simulink model "ABB_1010"  (R2024a)
(part 11 of 16)

et336 = Lxcm6.*Lz5.*dQ4.*dQ5.*m6.*t3.*t4.*t5.*t6.*t7.*t10.*-4.0-Lxcm6.*Lz5.*dQ1.*dQ2.*m6.*t2.*t4.*t7.*t9.*t10.*t11.*4.0-Lxcm6.*Lz5.*dQ1.*dQ4.*m6.*t2.*t3.*t7.*t8.*t10.*t11.*4.0+Lxcm6.*Lz4.*dQ1.*dQ6.*m6.*t2.*t3.*t7.*t8.*t10.*t11.*4.0-Lxcm6.*Lz5.*dQ1.*dQ3.*m6.*t2.*t4.*t7.*t9.*t10.*t11.*4.0-Lxcm6.*Lz5.*dQ1.*dQ2.*m6.*t3.*t4.*t8.*t9.*t10.*t11.*4.0-Lxcm6.*Lz5.*dQ1.*dQ3.*m6.*t3.*t4.*t8.*t9.*t10.*t11.*4.0-Lxcm6.*Lz5.*dQ2.*dQ4.*m6.*t2.*t4.*t8.*t9.*t10.*t11.*4.0-Lxcm6.*Lz5.*dQ2.*dQ4.*m6.*t3.*t4.*t7.*t9.*t10.*t11.*4.0-Lxcm6.*Lz5.*dQ3.*dQ4.*m6.*t2.*t4.*t8.*t9.*t10.*t11.*4.0-Lxcm6.*Lz5.*dQ3.*dQ4.*m6.*t3.*t4.*t7.*t9.*t10.*t11.*4.0-Lxcm6.*Lz5.*dQ2.*dQ5.*m6.*t5.*t6.*t7.*t8.*t9.*t10.*4.0-Lxcm6.*Lz5.*dQ3.*dQ5.*m6.*t5.*t6.*t7.*t8.*t9.*t10.*4.0-Lxcm6.*Lz4.*dQ1.*dQ4.*m6.*t2.*t5.*t6.*t7.*t9.*t33.*4.0;
et337 = Lxcm6.*Lz5.*dQ1.*dQ2.*m6.*t2.*t5.*t6.*t7.*t10.*t33.*-8.0+Lxcm6.*Lz5.*dQ1.*dQ5.*m6.*t2.*t3.*t6.*t7.*t8.*t34.*4.0-Lxcm6.*Lz4.*dQ1.*dQ4.*m6.*t3.*t5.*t6.*t8.*t9.*t32.*4.0-Lxcm6.*Lz4.*dQ1.*dQ5.*m6.*t2.*t4.*t6.*t7.*t10.*t33.*4.0+Lxcm6.*Lz5.*dQ1.*dQ2.*m6.*t2.*t5.*t6.*t7.*t10.*t34.*4.0-Lxcm6.*Lz5.*dQ1.*dQ2.*m6.*t3.*t5.*t6.*t8.*t10.*t32.*8.0-Lxcm6.*Lz5.*dQ1.*dQ3.*m6.*t2.*t5.*t6.*t7.*t10.*t33.*8.0-Lxcm6.*Lz5.*dQ1.*dQ4.*m6.*t2.*t4.*t5.*t7.*t11.*t33.*4.0-Lxcm6.*Lz5.*dQ1.*dQ5.*m6.*t2.*t3.*t6.*t7.*t8.*t35.*8.0-Lxcm6.*Lz4.*dQ1.*dQ5.*m6.*t3.*t4.*t6.*t8.*t10.*t32.*4.0-Lxcm6.*Lz4.*dQ1.*dQ6.*m6.*t2.*t4.*t5.*t7.*t11.*t33.*4.0+Lxcm6.*Lz5.*dQ1.*dQ3.*m6.*t2.*t5.*t6.*t7.*t10.*t34.*4.0-Lxcm6.*Lz5.*dQ1.*dQ3.*m6.*t3.*t5.*t6.*t8.*t10.*t32.*8.0-Lxcm6.*Lz5.*dQ1.*dQ4.*m6.*t3.*t4.*t5.*t8.*t11.*t32.*4.0;
et338 = Lxcm6.*Lz4.*dQ1.*dQ6.*m6.*t3.*t4.*t5.*t8.*t11.*t32.*-4.0+Lxcm6.*Lz5.*dQ1.*dQ2.*m6.*t3.*t5.*t6.*t8.*t10.*t34.*4.0-Lxcm6.*Lz5.*dQ1.*dQ6.*m6.*t2.*t5.*t6.*t7.*t9.*t33.*4.0+Lxcm6.*Lz5.*dQ1.*dQ3.*m6.*t3.*t5.*t6.*t8.*t10.*t34.*4.0-Lxcm6.*Lz5.*dQ1.*dQ6.*m6.*t3.*t5.*t6.*t8.*t9.*t32.*4.0+Lxcm6.*Lz5.*dQ1.*dQ4.*m6.*t4.*t5.*t6.*t9.*t10.*t32.*4.0+Lxcm6.*Lz5.*dQ2.*dQ4.*m6.*t2.*t5.*t6.*t8.*t10.*t34.*4.0+Lxcm6.*Lz5.*dQ2.*dQ4.*m6.*t3.*t5.*t6.*t7.*t10.*t34.*4.0+Lxcm6.*Lz5.*dQ1.*dQ4.*m6.*t4.*t5.*t6.*t9.*t10.*t33.*4.0+Lxcm6.*Lz5.*dQ3.*dQ4.*m6.*t2.*t5.*t6.*t8.*t10.*t34.*4.0+Lxcm6.*Lz5.*dQ3.*dQ4.*m6.*t3.*t5.*t6.*t7.*t10.*t34.*4.0+Lxcm6.*Lz5.*dQ1.*dQ5.*m6.*t2.*t7.*t9.*t10.*t11.*t33.*4.0+Lxcm6.*Lz5.*dQ1.*dQ5.*m6.*t3.*t8.*t9.*t10.*t11.*t32.*4.0-Lxcm6.*Lz5.*dQ1.*dQ4.*m6.*t2.*t6.*t7.*t9.*t33.*t35.*8.0;
et339 = Lxcm6.*Lz5.*dQ1.*dQ4.*m6.*t3.*t6.*t8.*t9.*t32.*t35.*-8.0-Lxcm6.*Lz5.*dQ1.*dQ6.*m6.*t2.*t4.*t7.*t11.*t33.*t35.*8.0-Lxcm6.*Lz5.*dQ1.*dQ5.*m6.*t4.*t5.*t9.*t11.*t32.*t33.*4.0-Lxcm6.*Lz5.*dQ1.*dQ6.*m6.*t3.*t4.*t8.*t11.*t32.*t35.*8.0-Lxcm6.*Lz5.*dQ1.*dQ6.*m6.*t4.*t6.*t9.*t10.*t32.*t33.*4.0-Lxcm6.*Lz5.*dQ1.*dQ6.*m6.*t5.*t10.*t11.*t32.*t33.*t34.*4.0+Lxcm6.*Lzcm6.*dQ1.*dQ2.*m6.*t2.*t3.*t4.*t6.*t7.*t8.*8.0+Lxcm6.*Lzcm6.*dQ1.*dQ3.*m6.*t2.*t3.*t4.*t6.*t7.*t8.*8.0+Lxcm5.*Lzcm5.*dQ2.*dQ3.*m5.*t2.*t3.*t4.*t5.*t9.*t10.*4.0+Lxcm6.*Lzcm6.*dQ1.*dQ5.*m6.*t2.*t4.*t5.*t6.*t7.*t10.*8.0+Lxcm6.*Lzcm6.*dQ1.*dQ5.*m6.*t3.*t4.*t5.*t6.*t8.*t10.*8.0+Lxcm6.*Lzcm6.*dQ2.*dQ5.*m6.*t2.*t3.*t5.*t6.*t9.*t10.*4.0+Lxcm6.*Lzcm6.*dQ3.*dQ5.*m6.*t2.*t3.*t5.*t6.*t9.*t10.*4.0-Lxcm6.*Lzcm6.*dQ4.*dQ5.*m6.*t2.*t4.*t5.*t6.*t8.*t10.*4.0;
et340 = Lxcm6.*Lzcm6.*dQ4.*dQ5.*m6.*t3.*t4.*t5.*t6.*t7.*t10.*-4.0-Lxcm5.*Lzcm5.*dQ2.*dQ3.*m5.*t4.*t5.*t7.*t8.*t9.*t10.*4.0-Lxcm6.*Lzcm6.*dQ1.*dQ2.*m6.*t2.*t4.*t7.*t9.*t10.*t11.*4.0-Lxcm6.*Lzcm6.*dQ1.*dQ4.*m6.*t2.*t3.*t7.*t8.*t10.*t11.*4.0-Lxcm6.*Lzcm6.*dQ1.*dQ3.*m6.*t2.*t4.*t7.*t9.*t10.*t11.*4.0-Lxcm6.*Lzcm6.*dQ1.*dQ2.*m6.*t3.*t4.*t8.*t9.*t10.*t11.*4.0-Lxcm6.*Lzcm6.*dQ1.*dQ3.*m6.*t3.*t4.*t8.*t9.*t10.*t11.*4.0-Lxcm6.*Lzcm6.*dQ2.*dQ4.*m6.*t2.*t4.*t8.*t9.*t10.*t11.*4.0-Lxcm6.*Lzcm6.*dQ2.*dQ4.*m6.*t3.*t4.*t7.*t9.*t10.*t11.*4.0-Lxcm6.*Lzcm6.*dQ3.*dQ4.*m6.*t2.*t4.*t8.*t9.*t10.*t11.*4.0-Lxcm6.*Lzcm6.*dQ3.*dQ4.*m6.*t3.*t4.*t7.*t9.*t10.*t11.*4.0-Lxcm6.*Lzcm6.*dQ2.*dQ5.*m6.*t5.*t6.*t7.*t8.*t9.*t10.*4.0-Lxcm6.*Lzcm6.*dQ3.*dQ5.*m6.*t5.*t6.*t7.*t8.*t9.*t10.*4.0-Lxcm5.*Lzcm5.*dQ1.*dQ2.*m5.*t2.*t3.*t4.*t7.*t8.*t35.*1.6e+1;
et341 = Lxcm5.*Lzcm5.*dQ1.*dQ3.*m5.*t2.*t3.*t4.*t7.*t8.*t35.*-1.6e+1-Lxcm5.*Lzcm5.*dQ1.*dQ5.*m5.*t2.*t4.*t5.*t7.*t10.*t33.*1.6e+1-Lxcm5.*Lzcm5.*dQ1.*dQ5.*m5.*t3.*t4.*t5.*t8.*t10.*t32.*1.6e+1-Lxcm6.*Lzcm6.*dQ1.*dQ2.*m6.*t2.*t5.*t6.*t7.*t10.*t33.*8.0+Lxcm6.*Lzcm6.*dQ1.*dQ5.*m6.*t2.*t3.*t6.*t7.*t8.*t34.*4.0+Lxcm6.*Lzcm6.*dQ1.*dQ2.*m6.*t2.*t5.*t6.*t7.*t10.*t34.*4.0-Lxcm6.*Lzcm6.*dQ1.*dQ2.*m6.*t3.*t5.*t6.*t8.*t10.*t32.*8.0-Lxcm6.*Lzcm6.*dQ1.*dQ3.*m6.*t2.*t5.*t6.*t7.*t10.*t33.*8.0-Lxcm6.*Lzcm6.*dQ1.*dQ4.*m6.*t2.*t4.*t5.*t7.*t11.*t33.*4.0-Lxcm6.*Lzcm6.*dQ1.*dQ5.*m6.*t2.*t3.*t6.*t7.*t8.*t35.*8.0+Lxcm6.*Lzcm6.*dQ1.*dQ3.*m6.*t2.*t5.*t6.*t7.*t10.*t34.*4.0-Lxcm6.*Lzcm6.*dQ1.*dQ3.*m6.*t3.*t5.*t6.*t8.*t10.*t32.*8.0-Lxcm6.*Lzcm6.*dQ1.*dQ4.*m6.*t3.*t4.*t5.*t8.*t11.*t32.*4.0+Lxcm6.*Lzcm6.*dQ1.*dQ2.*m6.*t3.*t5.*t6.*t8.*t10.*t34.*4.0;
et342 = Lxcm6.*Lzcm6.*dQ1.*dQ6.*m6.*t2.*t5.*t6.*t7.*t9.*t33.*-4.0+Lxcm6.*Lzcm6.*dQ1.*dQ3.*m6.*t3.*t5.*t6.*t8.*t10.*t34.*4.0-Lxcm6.*Lzcm6.*dQ1.*dQ6.*m6.*t3.*t5.*t6.*t8.*t9.*t32.*4.0+Lxcm6.*Lzcm6.*dQ1.*dQ4.*m6.*t4.*t5.*t6.*t9.*t10.*t32.*4.0+Lxcm6.*Lzcm6.*dQ2.*dQ4.*m6.*t2.*t5.*t6.*t8.*t10.*t34.*4.0+Lxcm6.*Lzcm6.*dQ2.*dQ4.*m6.*t3.*t5.*t6.*t7.*t10.*t34.*4.0+Lxcm6.*Lzcm6.*dQ1.*dQ4.*m6.*t4.*t5.*t6.*t9.*t10.*t33.*4.0+Lxcm6.*Lzcm6.*dQ3.*dQ4.*m6.*t2.*t5.*t6.*t8.*t10.*t34.*4.0+Lxcm6.*Lzcm6.*dQ3.*dQ4.*m6.*t3.*t5.*t6.*t7.*t10.*t34.*4.0+Lxcm6.*Lzcm6.*dQ1.*dQ5.*m6.*t2.*t7.*t9.*t10.*t11.*t33.*4.0+Lxcm6.*Lzcm6.*dQ1.*dQ5.*m6.*t3.*t8.*t9.*t10.*t11.*t32.*4.0-Lxcm5.*Lzcm5.*dQ1.*dQ2.*m5.*t2.*t5.*t7.*t10.*t33.*t34.*8.0-Lxcm5.*Lzcm5.*dQ1.*dQ2.*m5.*t3.*t5.*t8.*t10.*t32.*t34.*8.0-Lxcm5.*Lzcm5.*dQ1.*dQ3.*m5.*t2.*t5.*t7.*t10.*t33.*t34.*8.0;
et343 = Lxcm5.*Lzcm5.*dQ1.*dQ5.*m5.*t2.*t3.*t7.*t8.*t34.*t35.*-8.0-Lxcm5.*Lzcm5.*dQ1.*dQ3.*m5.*t3.*t5.*t8.*t10.*t32.*t34.*8.0-Lxcm5.*Lzcm5.*dQ1.*dQ4.*m5.*t4.*t5.*t9.*t10.*t32.*t33.*8.0-Lxcm6.*Lzcm6.*dQ1.*dQ4.*m6.*t2.*t6.*t7.*t9.*t33.*t35.*8.0-Lxcm6.*Lzcm6.*dQ1.*dQ4.*m6.*t3.*t6.*t8.*t9.*t32.*t35.*8.0-Lxcm6.*Lzcm6.*dQ1.*dQ6.*m6.*t2.*t4.*t7.*t11.*t33.*t35.*8.0-Lxcm6.*Lzcm6.*dQ1.*dQ5.*m6.*t4.*t5.*t9.*t11.*t32.*t33.*4.0-Lxcm6.*Lzcm6.*dQ1.*dQ6.*m6.*t3.*t4.*t8.*t11.*t32.*t35.*8.0-Lxcm6.*Lzcm6.*dQ1.*dQ6.*m6.*t4.*t6.*t9.*t10.*t32.*t33.*4.0-Lxcm6.*Lzcm6.*dQ1.*dQ6.*m6.*t5.*t10.*t11.*t32.*t33.*t34.*4.0+Lycm6.*Lz4.*dQ1.*dQ2.*m6.*t2.*t3.*t6.*t7.*t8.*t9.*8.0+Lycm6.*Lz4.*dQ1.*dQ3.*m6.*t2.*t3.*t6.*t7.*t8.*t9.*8.0-Lycm6.*Lz5.*dQ1.*dQ2.*m6.*t2.*t3.*t4.*t7.*t8.*t11.*8.0;
et344 = Lycm6.*Lz5.*dQ1.*dQ3.*m6.*t2.*t3.*t4.*t7.*t8.*t11.*-8.0+Lycm6.*Lz4.*dQ1.*dQ5.*m6.*t2.*t3.*t5.*t7.*t8.*t11.*4.0-Lycm6.*Lz5.*dQ1.*dQ2.*m6.*t2.*t4.*t6.*t7.*t9.*t10.*4.0-Lycm6.*Lz5.*dQ1.*dQ4.*m6.*t2.*t3.*t6.*t7.*t8.*t10.*4.0+Lycm6.*Lz4.*dQ1.*dQ6.*m6.*t2.*t3.*t6.*t7.*t8.*t10.*4.0-Lycm6.*Lz5.*dQ1.*dQ3.*m6.*t2.*t4.*t6.*t7.*t9.*t10.*4.0-Lycm6.*Lz5.*dQ1.*dQ2.*m6.*t3.*t4.*t6.*t8.*t9.*t10.*4.0-Lycm6.*Lz5.*dQ1.*dQ3.*m6.*t3.*t4.*t6.*t8.*t9.*t10.*4.0-Lycm6.*Lz5.*dQ1.*dQ5.*m6.*t2.*t4.*t5.*t7.*t10.*t11.*8.0-Lycm6.*Lz5.*dQ2.*dQ4.*m6.*t2.*t4.*t6.*t8.*t9.*t10.*4.0-Lycm6.*Lz5.*dQ2.*dQ4.*m6.*t3.*t4.*t6.*t7.*t9.*t10.*4.0-Lycm6.*Lz5.*dQ3.*dQ4.*m6.*t2.*t4.*t6.*t8.*t9.*t10.*4.0-Lycm6.*Lz5.*dQ3.*dQ4.*m6.*t3.*t4.*t6.*t7.*t9.*t10.*4.0-Lycm6.*Lz5.*dQ1.*dQ5.*m6.*t3.*t4.*t5.*t8.*t10.*t11.*8.0;
et345 = Lycm6.*Lz5.*dQ2.*dQ5.*m6.*t2.*t3.*t5.*t9.*t10.*t11.*-4.0-Lycm6.*Lz5.*dQ3.*dQ5.*m6.*t2.*t3.*t5.*t9.*t10.*t11.*4.0+Lycm6.*Lz5.*dQ4.*dQ5.*m6.*t2.*t4.*t5.*t8.*t10.*t11.*4.0+Lycm6.*Lz5.*dQ4.*dQ5.*m6.*t3.*t4.*t5.*t7.*t10.*t11.*4.0+Lycm6.*Lz5.*dQ2.*dQ5.*m6.*t5.*t7.*t8.*t9.*t10.*t11.*4.0+Lycm6.*Lz5.*dQ3.*dQ5.*m6.*t5.*t7.*t8.*t9.*t10.*t11.*4.0-Lycm6.*Lz5.*dQ1.*dQ4.*m6.*t2.*t4.*t5.*t6.*t7.*t33.*4.0-Lycm6.*Lz4.*dQ1.*dQ6.*m6.*t2.*t4.*t5.*t6.*t7.*t33.*4.0-Lycm6.*Lz5.*dQ1.*dQ4.*m6.*t3.*t4.*t5.*t6.*t8.*t32.*4.0-Lycm6.*Lz4.*dQ1.*dQ6.*m6.*t3.*t4.*t5.*t6.*t8.*t32.*4.0+Lycm6.*Lz4.*dQ1.*dQ4.*m6.*t2.*t5.*t7.*t9.*t11.*t33.*4.0+Lycm6.*Lz5.*dQ1.*dQ2.*m6.*t2.*t5.*t7.*t10.*t11.*t33.*8.0-Lycm6.*Lz5.*dQ1.*dQ5.*m6.*t2.*t3.*t7.*t8.*t11.*t34.*4.0+Lycm6.*Lz4.*dQ1.*dQ4.*m6.*t3.*t5.*t8.*t9.*t11.*t32.*4.0;
et346 = Lycm6.*Lz4.*dQ1.*dQ5.*m6.*t2.*t4.*t7.*t10.*t11.*t33.*4.0-Lycm6.*Lz5.*dQ1.*dQ2.*m6.*t2.*t5.*t7.*t10.*t11.*t34.*4.0+Lycm6.*Lz5.*dQ1.*dQ2.*m6.*t3.*t5.*t8.*t10.*t11.*t32.*8.0+Lycm6.*Lz5.*dQ1.*dQ3.*m6.*t2.*t5.*t7.*t10.*t11.*t33.*8.0+Lycm6.*Lz5.*dQ1.*dQ5.*m6.*t2.*t3.*t7.*t8.*t11.*t35.*8.0+Lycm6.*Lz4.*dQ1.*dQ5.*m6.*t3.*t4.*t8.*t10.*t11.*t32.*4.0-Lycm6.*Lz5.*dQ1.*dQ3.*m6.*t2.*t5.*t7.*t10.*t11.*t34.*4.0+Lycm6.*Lz5.*dQ1.*dQ3.*m6.*t3.*t5.*t8.*t10.*t11.*t32.*8.0+Lycm6.*Lz5.*dQ1.*dQ5.*m6.*t2.*t6.*t7.*t9.*t10.*t33.*4.0-Lycm6.*Lz5.*dQ1.*dQ2.*m6.*t3.*t5.*t8.*t10.*t11.*t34.*4.0+Lycm6.*Lz5.*dQ1.*dQ5.*m6.*t3.*t6.*t8.*t9.*t10.*t32.*4.0+Lycm6.*Lz5.*dQ1.*dQ6.*m6.*t2.*t5.*t7.*t9.*t11.*t33.*4.0-Lycm6.*Lz5.*dQ1.*dQ3.*m6.*t3.*t5.*t8.*t10.*t11.*t34.*4.0+Lycm6.*Lz5.*dQ1.*dQ6.*m6.*t3.*t5.*t8.*t9.*t11.*t32.*4.0;
et347 = Lycm6.*Lz5.*dQ1.*dQ4.*m6.*t4.*t5.*t9.*t10.*t11.*t32.*-4.0-Lycm6.*Lz5.*dQ2.*dQ4.*m6.*t2.*t5.*t8.*t10.*t11.*t34.*4.0-Lycm6.*Lz5.*dQ2.*dQ4.*m6.*t3.*t5.*t7.*t10.*t11.*t34.*4.0-Lycm6.*Lz5.*dQ2.*dQ5.*m6.*t2.*t4.*t8.*t9.*t11.*t35.*4.0-Lycm6.*Lz5.*dQ2.*dQ5.*m6.*t3.*t4.*t7.*t9.*t11.*t35.*4.0-Lycm6.*Lz5.*dQ1.*dQ4.*m6.*t4.*t5.*t9.*t10.*t11.*t33.*4.0-Lycm6.*Lz5.*dQ3.*dQ4.*m6.*t2.*t5.*t8.*t10.*t11.*t34.*4.0-Lycm6.*Lz5.*dQ3.*dQ4.*m6.*t3.*t5.*t7.*t10.*t11.*t34.*4.0-Lycm6.*Lz5.*dQ3.*dQ5.*m6.*t2.*t4.*t8.*t9.*t11.*t35.*4.0-Lycm6.*Lz5.*dQ3.*dQ5.*m6.*t3.*t4.*t7.*t9.*t11.*t35.*4.0-Lycm6.*Lz5.*dQ1.*dQ6.*m6.*t2.*t4.*t6.*t7.*t33.*t35.*8.0-Lycm6.*Lz5.*dQ1.*dQ5.*m6.*t4.*t5.*t6.*t9.*t32.*t33.*4.0-Lycm6.*Lz5.*dQ1.*dQ6.*m6.*t3.*t4.*t6.*t8.*t32.*t35.*8.0+Lycm6.*Lz5.*dQ1.*dQ4.*m6.*t2.*t7.*t9.*t11.*t33.*t35.*8.0;
et348 = Lycm6.*Lz5.*dQ1.*dQ4.*m6.*t3.*t8.*t9.*t11.*t32.*t35.*8.0+Lycm6.*Lz5.*dQ1.*dQ6.*m6.*t4.*t9.*t10.*t11.*t32.*t33.*4.0-Lycm6.*Lz5.*dQ1.*dQ6.*m6.*t5.*t6.*t10.*t32.*t33.*t34.*4.0+Lycm5.*Lzcm5.*dQ1.*dQ2.*m5.*t2.*t3.*t5.*t7.*t8.*t9.*8.0+Lycm5.*Lzcm5.*dQ1.*dQ3.*m5.*t2.*t3.*t5.*t7.*t8.*t9.*8.0-Lycm6.*Lzcm6.*dQ1.*dQ2.*m6.*t2.*t3.*t4.*t7.*t8.*t11.*8.0-Lycm6.*Lzcm6.*dQ1.*dQ3.*m6.*t2.*t3.*t4.*t7.*t8.*t11.*8.0-Lycm6.*Lzcm6.*dQ1.*dQ2.*m6.*t2.*t4.*t6.*t7.*t9.*t10.*4.0-Lycm6.*Lzcm6.*dQ1.*dQ4.*m6.*t2.*t3.*t6.*t7.*t8.*t10.*4.0-Lycm6.*Lzcm6.*dQ1.*dQ3.*m6.*t2.*t4.*t6.*t7.*t9.*t10.*4.0-Lycm6.*Lzcm6.*dQ1.*dQ2.*m6.*t3.*t4.*t6.*t8.*t9.*t10.*4.0-Lycm6.*Lzcm6.*dQ1.*dQ3.*m6.*t3.*t4.*t6.*t8.*t9.*t10.*4.0-Lycm6.*Lzcm6.*dQ1.*dQ5.*m6.*t2.*t4.*t5.*t7.*t10.*t11.*8.0-Lycm6.*Lzcm6.*dQ2.*dQ4.*m6.*t2.*t4.*t6.*t8.*t9.*t10.*4.0;
et349 = Lycm6.*Lzcm6.*dQ2.*dQ4.*m6.*t3.*t4.*t6.*t7.*t9.*t10.*-4.0-Lycm6.*Lzcm6.*dQ3.*dQ4.*m6.*t2.*t4.*t6.*t8.*t9.*t10.*4.0-Lycm6.*Lzcm6.*dQ3.*dQ4.*m6.*t3.*t4.*t6.*t7.*t9.*t10.*4.0-Lycm6.*Lzcm6.*dQ1.*dQ5.*m6.*t3.*t4.*t5.*t8.*t10.*t11.*8.0-Lycm6.*Lzcm6.*dQ2.*dQ5.*m6.*t2.*t3.*t5.*t9.*t10.*t11.*4.0-Lycm6.*Lzcm6.*dQ3.*dQ5.*m6.*t2.*t3.*t5.*t9.*t10.*t11.*4.0+Lycm6.*Lzcm6.*dQ4.*dQ5.*m6.*t2.*t4.*t5.*t8.*t10.*t11.*4.0+Lycm6.*Lzcm6.*dQ4.*dQ5.*m6.*t3.*t4.*t5.*t7.*t10.*t11.*4.0+Lycm6.*Lzcm6.*dQ2.*dQ5.*m6.*t5.*t7.*t8.*t9.*t10.*t11.*4.0+Lycm6.*Lzcm6.*dQ3.*dQ5.*m6.*t5.*t7.*t8.*t9.*t10.*t11.*4.0-Lycm6.*Lzcm6.*dQ1.*dQ4.*m6.*t2.*t4.*t5.*t6.*t7.*t33.*4.0-Lycm6.*Lzcm6.*dQ1.*dQ4.*m6.*t3.*t4.*t5.*t6.*t8.*t32.*4.0+Lycm5.*Lzcm5.*dQ1.*dQ2.*m5.*t2.*t4.*t7.*t9.*t10.*t33.*8.0+Lycm5.*Lzcm5.*dQ1.*dQ2.*m5.*t3.*t4.*t8.*t9.*t10.*t32.*8.0;
et350 = Lycm5.*Lzcm5.*dQ1.*dQ3.*m5.*t2.*t4.*t7.*t9.*t10.*t33.*8.0+Lycm5.*Lzcm5.*dQ1.*dQ4.*m5.*t2.*t3.*t7.*t8.*t10.*t34.*8.0+Lycm5.*Lzcm5.*dQ1.*dQ3.*m5.*t3.*t4.*t8.*t9.*t10.*t32.*8.0+Lycm6.*Lzcm6.*dQ1.*dQ2.*m6.*t2.*t5.*t7.*t10.*t11.*t33.*8.0-Lycm6.*Lzcm6.*dQ1.*dQ5.*m6.*t2.*t3.*t7.*t8.*t11.*t34.*4.0-Lycm6.*Lzcm6.*dQ1.*dQ2.*m6.*t2.*t5.*t7.*t10.*t11.*t34.*4.0+Lycm6.*Lzcm6.*dQ1.*dQ2.*m6.*t3.*t5.*t8.*t10.*t11.*t32.*8.0+Lycm6.*Lzcm6.*dQ1.*dQ3.*m6.*t2.*t5.*t7.*t10.*t11.*t33.*8.0+Lycm6.*Lzcm6.*dQ1.*dQ5.*m6.*t2.*t3.*t7.*t8.*t11.*t35.*8.0-Lycm6.*Lzcm6.*dQ1.*dQ3.*m6.*t2.*t5.*t7.*t10.*t11.*t34.*4.0+Lycm6.*Lzcm6.*dQ1.*dQ3.*m6.*t3.*t5.*t8.*t10.*t11.*t32.*8.0+Lycm6.*Lzcm6.*dQ1.*dQ5.*m6.*t2.*t6.*t7.*t9.*t10.*t33.*4.0-Lycm6.*Lzcm6.*dQ1.*dQ2.*m6.*t3.*t5.*t8.*t10.*t11.*t34.*4.0+Lycm6.*Lzcm6.*dQ1.*dQ5.*m6.*t3.*t6.*t8.*t9.*t10.*t32.*4.0;
et351 = Lycm6.*Lzcm6.*dQ1.*dQ6.*m6.*t2.*t5.*t7.*t9.*t11.*t33.*4.0-Lycm6.*Lzcm6.*dQ1.*dQ3.*m6.*t3.*t5.*t8.*t10.*t11.*t34.*4.0+Lycm6.*Lzcm6.*dQ1.*dQ6.*m6.*t3.*t5.*t8.*t9.*t11.*t32.*4.0-Lycm6.*Lzcm6.*dQ1.*dQ4.*m6.*t4.*t5.*t9.*t10.*t11.*t32.*4.0-Lycm6.*Lzcm6.*dQ2.*dQ4.*m6.*t2.*t5.*t8.*t10.*t11.*t34.*4.0-Lycm6.*Lzcm6.*dQ2.*dQ4.*m6.*t3.*t5.*t7.*t10.*t11.*t34.*4.0-Lycm6.*Lzcm6.*dQ2.*dQ5.*m6.*t2.*t4.*t8.*t9.*t11.*t35.*4.0-Lycm6.*Lzcm6.*dQ2.*dQ5.*m6.*t3.*t4.*t7.*t9.*t11.*t35.*4.0-Lycm6.*Lzcm6.*dQ1.*dQ4.*m6.*t4.*t5.*t9.*t10.*t11.*t33.*4.0-Lycm6.*Lzcm6.*dQ3.*dQ4.*m6.*t2.*t5.*t8.*t10.*t11.*t34.*4.0-Lycm6.*Lzcm6.*dQ3.*dQ4.*m6.*t3.*t5.*t7.*t10.*t11.*t34.*4.0-Lycm6.*Lzcm6.*dQ3.*dQ5.*m6.*t2.*t4.*t8.*t9.*t11.*t35.*4.0-Lycm6.*Lzcm6.*dQ3.*dQ5.*m6.*t3.*t4.*t7.*t9.*t11.*t35.*4.0-Lycm6.*Lzcm6.*dQ1.*dQ6.*m6.*t2.*t4.*t6.*t7.*t33.*t35.*8.0;
et352 = Lycm6.*Lzcm6.*dQ1.*dQ5.*m6.*t4.*t5.*t6.*t9.*t32.*t33.*-4.0-Lycm6.*Lzcm6.*dQ1.*dQ6.*m6.*t3.*t4.*t6.*t8.*t32.*t35.*8.0+Lycm6.*Lzcm6.*dQ1.*dQ4.*m6.*t2.*t7.*t9.*t11.*t33.*t35.*8.0+Lycm6.*Lzcm6.*dQ1.*dQ4.*m6.*t3.*t8.*t9.*t11.*t32.*t35.*8.0+Lycm6.*Lzcm6.*dQ1.*dQ6.*m6.*t4.*t9.*t10.*t11.*t32.*t33.*4.0-Lycm6.*Lzcm6.*dQ1.*dQ6.*m6.*t5.*t6.*t10.*t32.*t33.*t34.*4.0-Lz4.*Lz5.*dQ1.*dQ2.*m6.*t2.*t3.*t4.*t7.*t8.*t10.*8.0-Lz4.*Lz5.*dQ1.*dQ3.*m6.*t2.*t3.*t4.*t7.*t8.*t10.*8.0-Lz4.*Lzcm5.*dQ1.*dQ2.*m5.*t2.*t3.*t4.*t7.*t8.*t10.*8.0-Lz4.*Lzcm5.*dQ1.*dQ3.*m5.*t2.*t3.*t4.*t7.*t8.*t10.*8.0-Lz4.*Lzcm6.*dQ1.*dQ2.*m6.*t2.*t3.*t4.*t7.*t8.*t10.*8.0-Lz4.*Lzcm6.*dQ1.*dQ3.*m6.*t2.*t3.*t4.*t7.*t8.*t10.*8.0+Lz5.*Lzcm6.*dQ1.*dQ4.*m6.*t2.*t3.*t4.*t7.*t8.*t9.*8.0;
et353 = Lz5.*Lzcm6.*dQ1.*dQ5.*m6.*t2.*t3.*t5.*t7.*t8.*t10.*-8.0+Lz5.*Lzcm6.*dQ2.*dQ5.*m6.*t2.*t4.*t5.*t8.*t9.*t10.*4.0+Lz5.*Lzcm6.*dQ2.*dQ5.*m6.*t3.*t4.*t5.*t7.*t9.*t10.*4.0+Lz5.*Lzcm6.*dQ3.*dQ5.*m6.*t2.*t4.*t5.*t8.*t9.*t10.*4.0+Lz5.*Lzcm6.*dQ3.*dQ5.*m6.*t3.*t4.*t5.*t7.*t9.*t10.*4.0-Lz5.*Lzcm6.*dQ1.*dQ4.*m6.*t2.*t5.*t7.*t9.*t10.*t33.*8.0-Lz5.*Lzcm6.*dQ1.*dQ4.*m6.*t3.*t5.*t8.*t9.*t10.*t32.*8.0+Lx3.*Lxcm6.*dQ1.*dQ4.*m6.*t2.*t3.*t5.*t6.*t7.*t8.*t9.*4.0+Lx3.*Lxcm6.*dQ1.*dQ5.*m6.*t2.*t3.*t4.*t6.*t7.*t8.*t10.*4.0+Lx3.*Lxcm6.*dQ1.*dQ6.*m6.*t2.*t3.*t4.*t5.*t7.*t8.*t11.*4.0+Lx3.*Lycm6.*dQ1.*dQ6.*m6.*t2.*t3.*t4.*t5.*t6.*t7.*t8.*4.0-Lx3.*Lycm6.*dQ1.*dQ4.*m6.*t2.*t3.*t5.*t7.*t8.*t9.*t11.*4.0-Lx3.*Lycm6.*dQ1.*dQ5.*m6.*t2.*t3.*t4.*t7.*t8.*t10.*t11.*4.0-Lxcm5.*Lycm5.*dQ1.*dQ5.*m5.*t2.*t3.*t4.*t7.*t8.*t9.*t10.*4.0;
et354 = Lxcm6.*Lycm6.*dQ1.*dQ5.*m6.*t2.*t3.*t4.*t7.*t8.*t9.*t10.*4.0+Lxcm6.*Lycm6.*dQ1.*dQ4.*m6.*t2.*t5.*t6.*t7.*t9.*t10.*t11.*4.0+Lxcm6.*Lycm6.*dQ2.*dQ3.*m6.*t2.*t5.*t6.*t8.*t9.*t10.*t11.*4.0+Lxcm6.*Lycm6.*dQ2.*dQ3.*m6.*t3.*t5.*t6.*t7.*t9.*t10.*t11.*4.0+Lxcm6.*Lycm6.*dQ1.*dQ4.*m6.*t3.*t5.*t6.*t8.*t9.*t10.*t11.*4.0-Lxcm6.*Lycm6.*dQ2.*dQ3.*m6.*t2.*t3.*t4.*t6.*t9.*t11.*t35.*4.0-Lxcm6.*Lycm6.*dQ1.*dQ2.*m6.*t2.*t3.*t7.*t8.*t9.*t10.*t36.*1.6e+1-Lxcm6.*Lycm6.*dQ1.*dQ3.*m6.*t2.*t3.*t7.*t8.*t9.*t10.*t36.*1.6e+1-Lxcm6.*Lycm6.*dQ1.*dQ6.*m6.*t2.*t6.*t7.*t9.*t10.*t11.*t33.*1.6e+1+Lxcm6.*Lycm6.*dQ2.*dQ3.*m6.*t4.*t6.*t7.*t8.*t9.*t11.*t35.*4.0-Lxcm6.*Lycm6.*dQ1.*dQ6.*m6.*t3.*t6.*t8.*t9.*t10.*t11.*t32.*1.6e+1+Lxcm6.*Lycm6.*dQ1.*dQ2.*m6.*t2.*t4.*t5.*t7.*t9.*t33.*t36.*1.6e+1+Lxcm6.*Lycm6.*dQ1.*dQ2.*m6.*t3.*t4.*t5.*t8.*t9.*t32.*t36.*1.6e+1;
et355 = Lxcm6.*Lycm6.*dQ1.*dQ3.*m6.*t2.*t4.*t5.*t7.*t9.*t33.*t36.*1.6e+1+Lxcm6.*Lycm6.*dQ1.*dQ4.*m6.*t2.*t3.*t5.*t7.*t8.*t34.*t36.*1.6e+1+Lxcm6.*Lycm6.*dQ1.*dQ3.*m6.*t3.*t4.*t5.*t8.*t9.*t32.*t36.*1.6e+1+Lxcm6.*Lycm6.*dQ1.*dQ2.*m6.*t4.*t5.*t6.*t10.*t11.*t32.*t33.*1.6e+1+Lxcm6.*Lycm6.*dQ1.*dQ5.*m6.*t2.*t4.*t6.*t7.*t11.*t33.*t35.*1.6e+1+Lxcm6.*Lycm6.*dQ1.*dQ6.*m6.*t2.*t4.*t5.*t7.*t10.*t33.*t36.*1.6e+1+Lxcm6.*Lycm6.*dQ1.*dQ3.*m6.*t4.*t5.*t6.*t10.*t11.*t32.*t33.*1.6e+1+Lxcm6.*Lycm6.*dQ1.*dQ5.*m6.*t3.*t4.*t6.*t8.*t11.*t32.*t35.*1.6e+1+Lxcm6.*Lycm6.*dQ1.*dQ6.*m6.*t3.*t4.*t5.*t8.*t10.*t32.*t36.*1.6e+1+Lxcm6.*Lycm6.*dQ1.*dQ6.*m6.*t4.*t5.*t6.*t9.*t11.*t32.*t33.*1.6e+1+Lxcm6.*Lycm6.*dQ1.*dQ2.*m6.*t2.*t6.*t7.*t11.*t33.*t34.*t35.*8.0+Lxcm6.*Lycm6.*dQ1.*dQ2.*m6.*t3.*t6.*t8.*t11.*t32.*t34.*t35.*8.0+Lxcm6.*Lycm6.*dQ1.*dQ3.*m6.*t2.*t6.*t7.*t11.*t33.*t34.*t35.*8.0;
et356 = Lxcm6.*Lycm6.*dQ1.*dQ6.*m6.*t2.*t3.*t7.*t8.*t34.*t35.*t36.*8.0+Lxcm6.*Lycm6.*dQ1.*dQ3.*m6.*t3.*t6.*t8.*t11.*t32.*t34.*t35.*8.0+Lxcm6.*Lycm6.*dQ1.*dQ4.*m6.*t4.*t6.*t9.*t11.*t32.*t33.*t35.*8.0+Lxcm6.*Lycm6.*dQ1.*dQ5.*m6.*t5.*t6.*t10.*t11.*t32.*t33.*t34.*8.0-Lxcm6.*Lz4.*dQ1.*dQ2.*m6.*t2.*t3.*t4.*t5.*t6.*t7.*t8.*8.0-Lxcm6.*Lz4.*dQ1.*dQ3.*m6.*t2.*t3.*t4.*t5.*t6.*t7.*t8.*8.0+Lxcm6.*Lz5.*dQ2.*dQ3.*m6.*t2.*t3.*t4.*t5.*t6.*t9.*t10.*4.0+Lxcm6.*Lz5.*dQ1.*dQ2.*m6.*t2.*t3.*t5.*t7.*t8.*t9.*t11.*8.0+Lxcm6.*Lz5.*dQ1.*dQ3.*m6.*t2.*t3.*t5.*t7.*t8.*t9.*t11.*8.0+Lxcm6.*Lz5.*dQ1.*dQ6.*m6.*t2.*t3.*t5.*t7.*t8.*t10.*t11.*4.0-Lxcm6.*Lz5.*dQ2.*dQ3.*m6.*t4.*t5.*t6.*t7.*t8.*t9.*t10.*4.0-Lxcm6.*Lz5.*dQ2.*dQ6.*m6.*t2.*t4.*t5.*t8.*t9.*t10.*t11.*2.0-Lxcm6.*Lz5.*dQ2.*dQ6.*m6.*t3.*t4.*t5.*t7.*t9.*t10.*t11.*2.0;
et357 = Lxcm6.*Lz5.*dQ3.*dQ6.*m6.*t2.*t4.*t5.*t8.*t9.*t10.*t11.*-2.0-Lxcm6.*Lz5.*dQ3.*dQ6.*m6.*t3.*t4.*t5.*t7.*t9.*t10.*t11.*2.0-Lxcm6.*Lz5.*dQ1.*dQ2.*m6.*t2.*t3.*t4.*t6.*t7.*t8.*t35.*1.6e+1-Lxcm6.*Lz5.*dQ1.*dQ3.*m6.*t2.*t3.*t4.*t6.*t7.*t8.*t35.*1.6e+1-Lxcm6.*Lz5.*dQ1.*dQ5.*m6.*t2.*t4.*t5.*t6.*t7.*t10.*t33.*1.6e+1-Lxcm6.*Lz5.*dQ1.*dQ5.*m6.*t3.*t4.*t5.*t6.*t8.*t10.*t32.*1.6e+1+Lxcm6.*Lz5.*dQ1.*dQ2.*m6.*t2.*t4.*t7.*t9.*t10.*t11.*t33.*8.0+Lxcm6.*Lz5.*dQ1.*dQ2.*m6.*t3.*t4.*t8.*t9.*t10.*t11.*t32.*8.0+Lxcm6.*Lz5.*dQ1.*dQ3.*m6.*t2.*t4.*t7.*t9.*t10.*t11.*t33.*8.0+Lxcm6.*Lz5.*dQ1.*dQ4.*m6.*t2.*t3.*t7.*t8.*t10.*t11.*t34.*8.0+Lxcm6.*Lz5.*dQ1.*dQ3.*m6.*t3.*t4.*t8.*t9.*t10.*t11.*t32.*8.0-Lxcm6.*Lz5.*dQ1.*dQ2.*m6.*t2.*t5.*t6.*t7.*t10.*t33.*t34.*8.0;
et358 = Lxcm6.*Lz5.*dQ1.*dQ2.*m6.*t3.*t5.*t6.*t8.*t10.*t32.*t34.*-8.0-Lxcm6.*Lz5.*dQ1.*dQ3.*m6.*t2.*t5.*t6.*t7.*t10.*t33.*t34.*8.0-Lxcm6.*Lz5.*dQ1.*dQ5.*m6.*t2.*t3.*t6.*t7.*t8.*t34.*t35.*8.0-Lxcm6.*Lz5.*dQ1.*dQ3.*m6.*t3.*t5.*t6.*t8.*t10.*t32.*t34.*8.0-Lxcm6.*Lz5.*dQ1.*dQ4.*m6.*t4.*t5.*t6.*t9.*t10.*t32.*t33.*8.0+Lxcm6.*Lzcm6.*dQ2.*dQ3.*m6.*t2.*t3.*t4.*t5.*t6.*t9.*t10.*4.0+Lxcm6.*Lzcm6.*dQ1.*dQ2.*m6.*t2.*t3.*t5.*t7.*t8.*t9.*t11.*8.0+Lxcm6.*Lzcm6.*dQ1.*dQ3.*m6.*t2.*t3.*t5.*t7.*t8.*t9.*t11.*8.0+Lxcm6.*Lzcm6.*dQ1.*dQ6.*m6.*t2.*t3.*t5.*t7.*t8.*t10.*t11.*4.0-Lxcm6.*Lzcm6.*dQ2.*dQ3.*m6.*t4.*t5.*t6.*t7.*t8.*t9.*t10.*4.0-Lxcm6.*Lzcm6.*dQ2.*dQ6.*m6.*t2.*t4.*t5.*t8.*t9.*t10.*t11.*2.0-Lxcm6.*Lzcm6.*dQ2.*dQ6.*m6.*t3.*t4.*t5.*t7.*t9.*t10.*t11.*2.0-Lxcm6.*Lzcm6.*dQ3.*dQ6.*m6.*t2.*t4.*t5.*t8.*t9.*t10.*t11.*2.0;
et359 = Lxcm6.*Lzcm6.*dQ3.*dQ6.*m6.*t3.*t4.*t5.*t7.*t9.*t10.*t11.*-2.0-Lxcm6.*Lzcm6.*dQ1.*dQ2.*m6.*t2.*t3.*t4.*t6.*t7.*t8.*t35.*1.6e+1-Lxcm6.*Lzcm6.*dQ1.*dQ3.*m6.*t2.*t3.*t4.*t6.*t7.*t8.*t35.*1.6e+1-Lxcm6.*Lzcm6.*dQ1.*dQ5.*m6.*t2.*t4.*t5.*t6.*t7.*t10.*t33.*1.6e+1-Lxcm6.*Lzcm6.*dQ1.*dQ5.*m6.*t3.*t4.*t5.*t6.*t8.*t10.*t32.*1.6e+1+Lxcm6.*Lzcm6.*dQ1.*dQ2.*m6.*t2.*t4.*t7.*t9.*t10.*t11.*t33.*8.0+Lxcm6.*Lzcm6.*dQ1.*dQ2.*m6.*t3.*t4.*t8.*t9.*t10.*t11.*t32.*8.0+Lxcm6.*Lzcm6.*dQ1.*dQ3.*m6.*t2.*t4.*t7.*t9.*t10.*t11.*t33.*8.0+Lxcm6.*Lzcm6.*dQ1.*dQ4.*m6.*t2.*t3.*t7.*t8.*t10.*t11.*t34.*8.0+Lxcm6.*Lzcm6.*dQ1.*dQ3.*m6.*t3.*t4.*t8.*t9.*t10.*t11.*t32.*8.0-Lxcm6.*Lzcm6.*dQ1.*dQ2.*m6.*t2.*t5.*t6.*t7.*t10.*t33.*t34.*8.0-Lxcm6.*Lzcm6.*dQ1.*dQ2.*m6.*t3.*t5.*t6.*t8.*t10.*t32.*t34.*8.0;
et360 = Lxcm6.*Lzcm6.*dQ1.*dQ3.*m6.*t2.*t5.*t6.*t7.*t10.*t33.*t34.*-8.0-Lxcm6.*Lzcm6.*dQ1.*dQ5.*m6.*t2.*t3.*t6.*t7.*t8.*t34.*t35.*8.0-Lxcm6.*Lzcm6.*dQ1.*dQ3.*m6.*t3.*t5.*t6.*t8.*t10.*t32.*t34.*8.0-Lxcm6.*Lzcm6.*dQ1.*dQ4.*m6.*t4.*t5.*t6.*t9.*t10.*t32.*t33.*8.0+Lycm6.*Lz4.*dQ1.*dQ2.*m6.*t2.*t3.*t4.*t5.*t7.*t8.*t11.*8.0+Lycm6.*Lz4.*dQ1.*dQ3.*m6.*t2.*t3.*t4.*t5.*t7.*t8.*t11.*8.0+Lycm6.*Lz5.*dQ1.*dQ2.*m6.*t2.*t3.*t5.*t6.*t7.*t8.*t9.*8.0+Lycm6.*Lz5.*dQ1.*dQ3.*m6.*t2.*t3.*t5.*t6.*t7.*t8.*t9.*8.0+Lycm6.*Lz5.*dQ1.*dQ6.*m6.*t2.*t3.*t5.*t6.*t7.*t8.*t10.*4.0-Lycm6.*Lz5.*dQ2.*dQ3.*m6.*t2.*t3.*t4.*t5.*t9.*t10.*t11.*4.0-Lycm6.*Lz5.*dQ2.*dQ6.*m6.*t2.*t4.*t5.*t6.*t8.*t9.*t10.*2.0-Lycm6.*Lz5.*dQ2.*dQ6.*m6.*t3.*t4.*t5.*t6.*t7.*t9.*t10.*2.0-Lycm6.*Lz5.*dQ3.*dQ6.*m6.*t2.*t4.*t5.*t6.*t8.*t9.*t10.*2.0;
et361 = Lycm6.*Lz5.*dQ3.*dQ6.*m6.*t3.*t4.*t5.*t6.*t7.*t9.*t10.*-2.0+Lycm6.*Lz5.*dQ2.*dQ3.*m6.*t4.*t5.*t7.*t8.*t9.*t10.*t11.*4.0+Lycm6.*Lz5.*dQ1.*dQ2.*m6.*t2.*t3.*t4.*t7.*t8.*t11.*t35.*1.6e+1+Lycm6.*Lz5.*dQ1.*dQ2.*m6.*t2.*t4.*t6.*t7.*t9.*t10.*t33.*8.0+Lycm6.*Lz5.*dQ1.*dQ3.*m6.*t2.*t3.*t4.*t7.*t8.*t11.*t35.*1.6e+1+Lycm6.*Lz5.*dQ1.*dQ2.*m6.*t3.*t4.*t6.*t8.*t9.*t10.*t32.*8.0+Lycm6.*Lz5.*dQ1.*dQ3.*m6.*t2.*t4.*t6.*t7.*t9.*t10.*t33.*8.0+Lycm6.*Lz5.*dQ1.*dQ4.*m6.*t2.*t3.*t6.*t7.*t8.*t10.*t34.*8.0+Lycm6.*Lz5.*dQ1.*dQ3.*m6.*t3.*t4.*t6.*t8.*t9.*t10.*t32.*8.0+Lycm6.*Lz5.*dQ1.*dQ5.*m6.*t2.*t4.*t5.*t7.*t10.*t11.*t33.*1.6e+1+Lycm6.*Lz5.*dQ1.*dQ5.*m6.*t3.*t4.*t5.*t8.*t10.*t11.*t32.*1.6e+1+Lycm6.*Lz5.*dQ1.*dQ2.*m6.*t2.*t5.*t7.*t10.*t11.*t33.*t34.*8.0+Lycm6.*Lz5.*dQ1.*dQ2.*m6.*t3.*t5.*t8.*t10.*t11.*t32.*t34.*8.0;
et362 = Lycm6.*Lz5.*dQ1.*dQ3.*m6.*t2.*t5.*t7.*t10.*t11.*t33.*t34.*8.0+Lycm6.*Lz5.*dQ1.*dQ5.*m6.*t2.*t3.*t7.*t8.*t11.*t34.*t35.*8.0+Lycm6.*Lz5.*dQ1.*dQ3.*m6.*t3.*t5.*t8.*t10.*t11.*t32.*t34.*8.0+Lycm6.*Lz5.*dQ1.*dQ4.*m6.*t4.*t5.*t9.*t10.*t11.*t32.*t33.*8.0+Lycm5.*Lzcm5.*dQ1.*dQ5.*m5.*t2.*t3.*t4.*t5.*t7.*t8.*t9.*4.0+Lycm6.*Lzcm6.*dQ1.*dQ2.*m6.*t2.*t3.*t5.*t6.*t7.*t8.*t9.*8.0+Lycm6.*Lzcm6.*dQ1.*dQ3.*m6.*t2.*t3.*t5.*t6.*t7.*t8.*t9.*8.0+Lycm6.*Lzcm6.*dQ1.*dQ6.*m6.*t2.*t3.*t5.*t6.*t7.*t8.*t10.*4.0-Lycm6.*Lzcm6.*dQ2.*dQ3.*m6.*t2.*t3.*t4.*t5.*t9.*t10.*t11.*4.0-Lycm6.*Lzcm6.*dQ2.*dQ6.*m6.*t2.*t4.*t5.*t6.*t8.*t9.*t10.*2.0-Lycm6.*Lzcm6.*dQ2.*dQ6.*m6.*t3.*t4.*t5.*t6.*t7.*t9.*t10.*2.0-Lycm6.*Lzcm6.*dQ3.*dQ6.*m6.*t2.*t4.*t5.*t6.*t8.*t9.*t10.*2.0-Lycm6.*Lzcm6.*dQ3.*dQ6.*m6.*t3.*t4.*t5.*t6.*t7.*t9.*t10.*2.0;
et363 = Lycm6.*Lzcm6.*dQ2.*dQ3.*m6.*t4.*t5.*t7.*t8.*t9.*t10.*t11.*4.0+Lycm6.*Lzcm6.*dQ1.*dQ2.*m6.*t2.*t3.*t4.*t7.*t8.*t11.*t35.*1.6e+1+Lycm6.*Lzcm6.*dQ1.*dQ2.*m6.*t2.*t4.*t6.*t7.*t9.*t10.*t33.*8.0+Lycm6.*Lzcm6.*dQ1.*dQ3.*m6.*t2.*t3.*t4.*t7.*t8.*t11.*t35.*1.6e+1+Lycm6.*Lzcm6.*dQ1.*dQ2.*m6.*t3.*t4.*t6.*t8.*t9.*t10.*t32.*8.0+Lycm6.*Lzcm6.*dQ1.*dQ3.*m6.*t2.*t4.*t6.*t7.*t9.*t10.*t33.*8.0+Lycm6.*Lzcm6.*dQ1.*dQ4.*m6.*t2.*t3.*t6.*t7.*t8.*t10.*t34.*8.0+Lycm6.*Lzcm6.*dQ1.*dQ3.*m6.*t3.*t4.*t6.*t8.*t9.*t10.*t32.*8.0+Lycm6.*Lzcm6.*dQ1.*dQ5.*m6.*t2.*t4.*t5.*t7.*t10.*t11.*t33.*1.6e+1+Lycm6.*Lzcm6.*dQ1.*dQ5.*m6.*t3.*t4.*t5.*t8.*t10.*t11.*t32.*1.6e+1+Lycm6.*Lzcm6.*dQ1.*dQ2.*m6.*t2.*t5.*t7.*t10.*t11.*t33.*t34.*8.0+Lycm6.*Lzcm6.*dQ1.*dQ2.*m6.*t3.*t5.*t8.*t10.*t11.*t32.*t34.*8.0+Lycm6.*Lzcm6.*dQ1.*dQ3.*m6.*t2.*t5.*t7.*t10.*t11.*t33.*t34.*8.0;
et364 = Lycm6.*Lzcm6.*dQ1.*dQ5.*m6.*t2.*t3.*t7.*t8.*t11.*t34.*t35.*8.0+Lycm6.*Lzcm6.*dQ1.*dQ3.*m6.*t3.*t5.*t8.*t10.*t11.*t32.*t34.*8.0+Lycm6.*Lzcm6.*dQ1.*dQ4.*m6.*t4.*t5.*t9.*t10.*t11.*t32.*t33.*8.0-Lz5.*Lzcm6.*dQ1.*dQ2.*m6.*t2.*t3.*t4.*t5.*t7.*t8.*t10.*1.6e+1-Lz5.*Lzcm6.*dQ1.*dQ3.*m6.*t2.*t3.*t4.*t5.*t7.*t8.*t10.*1.6e+1-Lz5.*Lzcm6.*dQ1.*dQ4.*m6.*t2.*t3.*t4.*t7.*t8.*t9.*t35.*8.0-Lz5.*Lzcm6.*dQ1.*dQ5.*m6.*t2.*t3.*t5.*t7.*t8.*t10.*t34.*8.0-Ixy6.*dQ1.*dQ2.*t2.*t3.*t4.*t5.*t6.*t7.*t8.*t10.*t11.*8.0-Ixy6.*dQ1.*dQ3.*t2.*t3.*t4.*t5.*t6.*t7.*t8.*t10.*t11.*8.0-Ixy6.*dQ1.*dQ4.*t2.*t3.*t4.*t6.*t7.*t8.*t9.*t11.*t35.*4.0-Iyx6.*dQ1.*dQ2.*t2.*t3.*t4.*t5.*t6.*t7.*t8.*t10.*t11.*8.0-Iyx6.*dQ1.*dQ3.*t2.*t3.*t4.*t5.*t6.*t7.*t8.*t10.*t11.*8.0;
et365 = Iyx6.*dQ1.*dQ4.*t2.*t3.*t4.*t6.*t7.*t8.*t9.*t11.*t35.*-4.0-dQ1.*dQ2.*m6.*t2.*t3.*t6.*t7.*t8.*t9.*t10.*t11.*t17.*8.0-dQ1.*dQ3.*m6.*t2.*t3.*t6.*t7.*t8.*t9.*t10.*t11.*t17.*8.0+dQ1.*dQ2.*m6.*t2.*t3.*t6.*t7.*t8.*t9.*t10.*t11.*t20.*8.0+dQ1.*dQ3.*m6.*t2.*t3.*t6.*t7.*t8.*t9.*t10.*t11.*t20.*8.0+dQ1.*dQ2.*m6.*t2.*t3.*t4.*t5.*t7.*t8.*t10.*t17.*t36.*8.0+dQ1.*dQ3.*m6.*t2.*t3.*t4.*t5.*t7.*t8.*t10.*t17.*t36.*8.0+dQ1.*dQ2.*m6.*t2.*t4.*t5.*t6.*t7.*t9.*t11.*t17.*t33.*8.0-dQ1.*dQ2.*m6.*t2.*t3.*t4.*t5.*t7.*t8.*t10.*t20.*t36.*8.0+dQ1.*dQ2.*m6.*t3.*t4.*t5.*t6.*t8.*t9.*t11.*t17.*t32.*8.0+dQ1.*dQ3.*m6.*t2.*t4.*t5.*t6.*t7.*t9.*t11.*t17.*t33.*8.0+dQ1.*dQ4.*m6.*t2.*t3.*t5.*t6.*t7.*t8.*t11.*t17.*t34.*8.0+dQ1.*dQ6.*m6.*t2.*t3.*t4.*t5.*t7.*t8.*t9.*t17.*t36.*8.0;
et366 = dQ1.*dQ3.*m6.*t2.*t3.*t4.*t5.*t7.*t8.*t10.*t20.*t36.*-8.0+dQ1.*dQ3.*m6.*t3.*t4.*t5.*t6.*t8.*t9.*t11.*t17.*t32.*8.0-dQ1.*dQ2.*m6.*t2.*t4.*t5.*t6.*t7.*t9.*t11.*t20.*t33.*8.0-dQ1.*dQ2.*m6.*t3.*t4.*t5.*t6.*t8.*t9.*t11.*t20.*t32.*8.0-dQ1.*dQ3.*m6.*t2.*t4.*t5.*t6.*t7.*t9.*t11.*t20.*t33.*8.0-dQ1.*dQ4.*m6.*t2.*t3.*t5.*t6.*t7.*t8.*t11.*t20.*t34.*8.0-dQ1.*dQ6.*m6.*t2.*t3.*t4.*t5.*t7.*t8.*t9.*t20.*t36.*8.0-dQ1.*dQ3.*m6.*t3.*t4.*t5.*t6.*t8.*t9.*t11.*t20.*t32.*8.0+dQ1.*dQ6.*m6.*t2.*t4.*t5.*t6.*t7.*t10.*t11.*t17.*t33.*8.0+dQ1.*dQ6.*m6.*t3.*t4.*t5.*t6.*t8.*t10.*t11.*t17.*t32.*8.0-dQ1.*dQ6.*m6.*t2.*t4.*t5.*t6.*t7.*t10.*t11.*t20.*t33.*8.0-dQ1.*dQ6.*m6.*t3.*t4.*t5.*t6.*t8.*t10.*t11.*t20.*t32.*8.0;
et367 = dQ1.*dQ4.*m6.*t2.*t3.*t4.*t7.*t8.*t9.*t17.*t35.*t36.*4.0+dQ1.*dQ5.*m6.*t2.*t3.*t5.*t7.*t8.*t10.*t17.*t34.*t36.*4.0-dQ1.*dQ4.*m6.*t2.*t3.*t4.*t7.*t8.*t9.*t20.*t35.*t36.*4.0+dQ1.*dQ6.*m6.*t2.*t3.*t6.*t7.*t8.*t11.*t17.*t34.*t35.*4.0-dQ1.*dQ5.*m6.*t2.*t3.*t5.*t7.*t8.*t10.*t20.*t34.*t36.*4.0-dQ1.*dQ6.*m6.*t2.*t3.*t6.*t7.*t8.*t11.*t20.*t34.*t35.*4.0-dQ1.*dQ5.*m6.*t2.*t3.*t4.*t6.*t7.*t8.*t9.*t10.*t11.*t17.*4.0+dQ1.*dQ5.*m6.*t2.*t3.*t4.*t6.*t7.*t8.*t9.*t10.*t11.*t20.*4.0-Lxcm6.*Lycm6.*dQ1.*dQ4.*m6.*t2.*t3.*t4.*t6.*t7.*t8.*t9.*t11.*8.0-Lxcm6.*Lycm6.*dQ1.*dQ5.*m6.*t2.*t3.*t5.*t6.*t7.*t8.*t10.*t11.*8.0-Lxcm6.*Lycm6.*dQ1.*dQ5.*m6.*t2.*t3.*t4.*t7.*t8.*t9.*t10.*t36.*8.0-Lxcm6.*Lycm6.*dQ1.*dQ4.*m6.*t2.*t5.*t6.*t7.*t9.*t10.*t11.*t33.*8.0;
et368 = Lxcm6.*Lycm6.*dQ1.*dQ4.*m6.*t3.*t5.*t6.*t8.*t9.*t10.*t11.*t32.*-8.0+Lxcm6.*Lz5.*dQ1.*dQ5.*m6.*t2.*t3.*t4.*t5.*t7.*t8.*t9.*t11.*4.0+Lxcm6.*Lz5.*dQ1.*dQ6.*m6.*t2.*t3.*t4.*t6.*t7.*t8.*t9.*t10.*4.0+Lxcm6.*Lz5.*dQ1.*dQ6.*m6.*t2.*t3.*t5.*t7.*t8.*t10.*t11.*t34.*4.0+Lxcm5.*Lzcm5.*dQ1.*dQ4.*m5.*t2.*t3.*t4.*t5.*t7.*t8.*t9.*t10.*8.0+Lxcm6.*Lzcm6.*dQ1.*dQ5.*m6.*t2.*t3.*t4.*t5.*t7.*t8.*t9.*t11.*4.0+Lxcm6.*Lzcm6.*dQ1.*dQ6.*m6.*t2.*t3.*t4.*t6.*t7.*t8.*t9.*t10.*4.0+Lxcm6.*Lzcm6.*dQ1.*dQ6.*m6.*t2.*t3.*t5.*t7.*t8.*t10.*t11.*t34.*4.0+Lycm6.*Lz5.*dQ1.*dQ5.*m6.*t2.*t3.*t4.*t5.*t6.*t7.*t8.*t9.*4.0-Lycm6.*Lz5.*dQ1.*dQ6.*m6.*t2.*t3.*t4.*t7.*t8.*t9.*t10.*t11.*4.0+Lycm6.*Lz5.*dQ1.*dQ6.*m6.*t2.*t3.*t5.*t6.*t7.*t8.*t10.*t34.*4.0+Lycm6.*Lzcm6.*dQ1.*dQ5.*m6.*t2.*t3.*t4.*t5.*t6.*t7.*t8.*t9.*4.0-Lycm6.*Lzcm6.*dQ1.*dQ6.*m6.*t2.*t3.*t4.*t7.*t8.*t9.*t10.*t11.*4.0;
et369 = Lycm6.*Lzcm6.*dQ1.*dQ6.*m6.*t2.*t3.*t5.*t6.*t7.*t8.*t10.*t34.*4.0-Lxcm6.*Lycm6.*dQ1.*dQ2.*m6.*t2.*t3.*t4.*t5.*t6.*t7.*t8.*t10.*t11.*1.6e+1-Lxcm6.*Lycm6.*dQ1.*dQ3.*m6.*t2.*t3.*t4.*t5.*t6.*t7.*t8.*t10.*t11.*1.6e+1-Lxcm6.*Lycm6.*dQ1.*dQ6.*m6.*t2.*t3.*t4.*t5.*t6.*t7.*t8.*t9.*t11.*1.6e+1-Lxcm6.*Lycm6.*dQ1.*dQ4.*m6.*t2.*t3.*t4.*t6.*t7.*t8.*t9.*t11.*t35.*8.0-Lxcm6.*Lycm6.*dQ1.*dQ5.*m6.*t2.*t3.*t5.*t6.*t7.*t8.*t10.*t11.*t34.*8.0+Lxcm6.*Lz5.*dQ1.*dQ4.*m6.*t2.*t3.*t4.*t5.*t6.*t7.*t8.*t9.*t10.*8.0+Lxcm6.*Lzcm6.*dQ1.*dQ4.*m6.*t2.*t3.*t4.*t5.*t6.*t7.*t8.*t9.*t10.*8.0-Lycm6.*Lz5.*dQ1.*dQ4.*m6.*t2.*t3.*t4.*t5.*t7.*t8.*t9.*t10.*t11.*8.0-Lycm6.*Lzcm6.*dQ1.*dQ4.*m6.*t2.*t3.*t4.*t5.*t7.*t8.*t9.*t10.*t11.*8.0;
et370 = et1+et2+et3+et4+et5+et6+et7+et8+et9+et10+et11+et12+et13+et14+et15+et16+et17+et18+et19+et20+et21+et22+et23+et24+et25+et26+et27+et28+et29+et30+et31+et32+et33+et34+et35+et36+et37+et38+et39+et40+et41+et42+et43+et44+et45+et46+et47+et48+et49+et50+et51+et52+et53+et54+et55+et56+et57+et58+et59+et60+et61+et62+et63+et64+et65+et66+et67+et68+et69+et70+et71+et72+et73+et74+et75+et76+et77+et78+et79+et80+et81+et82+et83+et84+et85+et86+et87+et88+et89+et90+et91+et92+et93+et94+et95+et96+et97+et98+et99+et100+et101+et102+et103+et104+et105+et106+et107+et108+et109+et110+et111+et112+et113+et114+et115+et116+et117+et118+et119+et120+et121+et122+et123+et124+et125+et126+et127+et128+et129+et130+et131+et132+et133+et134+et135+et136+et137+et138+et139+et140+et141+et142+et143+et144+et145+et146+et147+et148+et149+et150+et151+et152+et153+et154+et155+et156+et157+et158+et159+et160+et161+et162+et163+et164+et165+et166+et167+et168+et169+et170+et171+et172+et173+et174+et175+et176+et177+et178+et179+et180+et181+et182+et183+et184+et185+et186+et187+et188+et189+et190+et191+et192+et193+et194+et195+et196+et197+et198+et199+et200;
et371 = et201+et202+et203+et204+et205+et206+et207+et208+et209+et210+et211+et212+et213+et214+et215+et216+et217+et218+et219+et220+et221+et222+et223+et224+et225+et226+et227+et228+et229+et230+et231+et232+et233+et234+et235+et236+et237+et238+et239+et240+et241+et242+et243+et244+et245+et246+et247+et248+et249+et250+et251+et252+et253+et254+et255+et256+et257+et258+et259+et260+et261+et262+et263+et264+et265+et266+et267+et268+et269+et270+et271+et272+et273+et274+et275+et276+et277+et278+et279+et280+et281+et282+et283+et284+et285+et286+et287+et288+et289+et290+et291+et292+et293+et294+et295+et296+et297+et298+et299+et300+et301+et302+et303+et304+et305+et306+et307+et308+et309+et310+et311+et312+et313+et314+et315+et316+et317+et318+et319+et320+et321+et322+et323+et324+et325+et326+et327+et328+et329+et330+et331+et332+et333+et334+et335+et336+et337+et338+et339+et340+et341+et342+et343+et344+et345+et346+et347+et348+et349+et350+et351+et352+et353+et354+et355+et356+et357+et358+et359+et360+et361+et362+et363+et364+et365+et366+et367+et368+et369;
et372 = t42+t43+t44+t45+t46+t47+t48+t49+t50+t51+t54+t55+t56+t57+t58+t61+t62+t63+t64+t67+t68+t69+t72+t73+t78+t79+t80+t81+t82+t83+t84+t85+t86+t87+t88+t89+t90+t91+t92+t93+t94+t96+t100+t102+t106+t107+t118+t119+t120+t121+t122+t123+t124+t125+t126+t127+t128+t129+t132+t138+t139+t141+t142+t143+t144+t145+t146+t147+t148+t149+t150+t151+t152+t153+t154+t155+t156+t157+t170+t171+t174+t177+t178+t179+t180+t185+t186+t201+t202+t203+t204+t205+t206+t207+t208+t209+t210+t211+t212+t213+t214+t215+t216+t217+t218+t219+t220+t222+t225+t227+t228+t229+t230+t231+t232+t233+t234+t235+t236+t237+t242+t243+t244+t245+t250+t251+t252+t253+t258+t259+t260+t263+t264+t265+t266+t269+t270+t273+t274+t276+t277+t278+t279+t282+t283+t286+t287+t289+t290+t292+t293+t297+t298+t299+t300+t301+t302+t303+t304+t305+t306+t307+t308+t309+t310+t311+t312+t313+t314+t315+t316+t317+t318+t319+t320+t321+t322+t323+t324+t325+t326+t327+t328+t331+t332+t333+t334+t340+t341+t342+t343+t349+t351+t358+t363+t364+t367+t368+t369+t370;
et373 = t377+t378+t379+t380+t381+t382+t383+t384+t385+t386+t402+t403+t404+t405+t406+t407+t415+t416+t417+t418+t419+t430+t431+t432+t433+t434+t435+t436+t437+t438+t442+t443+t444+t445+t446+t447+t454+t455+t456+t457+t458+t459+t460+t461+t462+t463+t464+t465+t466+t467+t468+t469+t470+t471+t472+t473+t474+t475+t476+t477+t478+t479+t480+t481+t482+t483+t484+t485+t486+t487+t488+t489+t490+t491+t492+t493+t494+t495+t496+t497+t498+t500+t506+t512+t514+t515+t516+t527+t528+t529+t540+t542+t543+t544+t546+t547+t548+t550+t552+t554+t555+t556+t557+t558+t559+t560+t561+t562+t563+t564+t565+t566+t567+t568+t569+t570+t571+t572+t573+t574+t575+t576+t577+t578+t579+t580+t581+t582+t583+t584+t585+t586+t587+t588+t589+t590+t591+t592+t593+t594+t595+t596+t597+t598+t599+t600+t601+t602+t603+t604+t605+t606+t607+t608+t609+t610+t611+t612+t613+t614+t615+t616+t617+t618+t619+t620+t621+t622+t623+t624+t625+t626+t627+t628+t629+t630+t631+t632+t635+t636+t637+t638+t648+t650+t651+t658+t659+t660+t661+t662+t663+t664+t669+t670+t671+t674+t675+t676+t677+t681;
et374 = t684+t687+t688+t689+t690+t694+t697+t698+t699+t700+t701+t702+t703+t704+t705+t706+t707+t708+t709+t710+t711+t716+t717+t718+t719+t720+t721+t724+t725+t728+t729+t730+t731+t732+t733+t734+t735+t737+t738+t739+t746+t748+t749+t750+t752+t754+t755+t756+t759+t760+t761+t762+t774+t775+t776+t777+t778+t779+t780+t781+t782+t783+t785+t788+t791+t792+t793+t794+t795+t798+t800+t801+t803+t804+t806+t807+t809+t810+t828+t829+t830+t831+t832+t833+t834+t835+t836+t837+t838+t839+t840+t843+t844+t845+t848+t849+t851+t852+t857+t858+t861+t862+t868+t869+t870+t871+t872+t873+t874+t875+t876+t877+t878+t879+t880+t881+t882+t883+t884+t885+t886+t887+t888+t889+t890+t891+t892+t893+t894+t895+t896+t897+t898+t899+t900+t901+t902+t903+t904+t905+t906+t907+t908+t909+t910+t911+t912+t913+t914+t915+t916+t917+t918+t919+t920+t921+t922+t923+t924+t925+t926+t927+t928+t929+t930+t931+t932+t933+t934+t935+t936+t938+t939+t940+t941+t942+t943+t950+t951+t952+t953+t954+t955+t956+t957+t958+t959+t960+t961+t962+t963+t964+t965+t966+t967+t968+t969+t972+t973+t978;
et375 = t979+t984+t985+t988+t989+t990+t991+t992+t993+t994+t995+t996+t997+t998+t1001+t1002+t1003+t1004+t1005+t1006+t1007+t1008+t1009+t1010+t1011+t1012+t1013+t1014+t1015+t1016+t1017+t1018+t1019+t1020+t1021+t1022+t1023+t1024+t1025+t1026+t1027+t1028+t1029+t1030+t1033+t1034+t1035+t1036+t1037+t1038+t1039+t1041+t1046+t1060+t1061+t1062+t1063+t1064+t1065+t1066+t1067+t1072+t1073+t1074+t1075+t1076+t1077+t1078+t1079+t1082+t1083+t1084+t1085+t1093+t1094+t1095+t1096+t1097+t1098+t1099+t1103+t1104+t1105+t1106+t1107+t1108+t1109+t1110+t1111+t1112+t1113+t1114+t1115+t1116+t1117+t1118+t1120+t1127+t1139+t1140+t1145+t1146+t1147+t1148+t1149+t1150+t1154+t1155+t1158+t1159+t1167+t1169+t1170+t1173+t1174+t1175+t1177+t1178+t1179+t1180+t1181+t1182+t1187+t1193+t1194+t1197+t1198+t1199+t1200+t1202+t1204+t1205+t1206+t1208+t1213+t1214+t1215+t1216+t1217+t1218+t1219+t1223+t1224+t1225+t1226+t1227+t1228+t1229+t1230+t1231+t1242+t1243+t1246+t1249+t1250+t1251+t1252+t1253+t1254+t1255+t1256+t1257+t1258+t1259+t1262+t1263+t1264+t1265+t1266+t1269+t1272+t1275+t1276+t1278+t1279+t1283+t1285+t1286+t1287+t1288+t1289+t1290+t1291+t1292+t1293+t1294+t1295+t1296+t1297+t1298+t1299+t1300+t1301+t1302+t1303+t1304+t1305+t1306+t1307+t1308;
et376 = t1309+t1310+t1311+t1312+t1313+t1314+t1315+t1316+t1317+t1318+t1319+t1320+t1321+t1322+t1323+t1324+t1325+t1326+t1327+t1328+t1329+t1330+t1331+t1332+t1333+t1334+t1335+t1336+t1337+t1338+t1339+t1340+t1341+t1342+t1343+t1344+t1345+t1346+t1347+t1348+t1349+t1350+t1351+t1352+t1353+t1354+t1355+t1356+t1357+t1358+t1359+t1360+t1361+t1362+t1363+t1364+t1365+t1366+t1367+t1368+t1369+t1370+t1371+t1372+t1373+t1374+t1375+t1376+t1377+t1378+t1379+t1381+t1382+t1383+t1384+t1385+t1386+t1387+t1388+t1389+t1390+t1391+t1392+t1393+t1394+t1395+t1396+t1397+t1398+t1399+t1400+t1401+t1402+t1403+t1404+t1405+t1406+t1407+t1408+t1409+t1410+t1411+t1420+t1421+t1422+t1423+t1424+t1425+t1426+t1427+t1428+t1429+t1430+t1431+t1432+t1433+t1434+t1435+t1436+t1437+t1438+t1439+t1440+t1441+t1442+t1443+t1444+t1445+t1446+t1447+t1448+t1449+t1450+t1451+t1452+t1453+t1454+t1455+t1456+t1457+t1458+t1469+t1471+t1472+t1474+t1475+t1481+t1482+t1484+t1487+t1490+t1493+t1496+t1497+t1498+t1499+t1500+t1501+t1502+t1503+t1504+t1505+t1506+t1507+t1508+t1509+t1510+t1511+t1512+t1513+t1514+t1515+t1516+t1517+t1518+t1519+t1520+t1521+t1522+t1523+t1524+t1525+t1526+t1531+t1532+t1533+t1534+t1535+t1536+t1539+t1540+t1547+t1548+t1549+t1550+t1555+t1560+t1561+t1562+t1565;
et377 = t1566+t1575+t1576+t1577+t1578+t1579+t1580+t1581+t1582+t1583+t1589+t1590+t1591+t1592+t1593+t1594+t1595+t1596+t1597+t1600+t1601+t1602+t1603+t1604+t1605+t1610+t1613+t1617+t1618+t1619+t1627+t1628+t1629+t1630+t1631+t1632+t1633+t1634+t1637+t1639+t1640+t1641+t1642+t1643+t1644+t1645+t1646+t1647+t1648+t1649+t1650+t1651+t1652+t1653+t1654+t1655+t1656+t1657+t1658+t1659+t1660+t1661+t1662+t1663+t1664+t1665+t1672+t1673+t1674+t1675+t1676+t1677+t1678+t1679+t1680+t1683+t1684+t1687+t1688+t1691+t1694+t1695+t1696+t1697+t1698+t1699+t1700+t1721+t1722+t1725+t1726+t1730+t1731+t1733+t1734+t1735+t1736+t1740+t1744+t1745+t1754+t1755+t1756+t1759+t1760+t1761+t1762+t1763+t1764+t1765+t1766+t1767+t1768+t1769+t1770+t1771+t1772+t1773+t1774+t1775+t1777+t1778+t1779+t1780+t1781+t1782+t1783+t1784+t1785+t1786+t1787+t1788+t1789+t1790+t1791+t1792+t1793+t1794+t1795+t1796+t1797+t1798+t1799+t1800+t1801+t1802+t1803+t1804+t1814+t1815+t1816+t1817+t1818+t1819+t1820+t1821+t1822+t1823+t1827+t1828+t1829+t1830+t1831+t1832+t1833+t1834+t1835+t1840+t1841+t1847+t1850+t1851+t1852+t1853+t1854+t1855+t1856+t1857+t1858+t1859+t1860+t1861+t1862+t1863+t1864+t1865+t1866+t1867+t1868+t1869+t1870+t1871+t1872+t1873+t1874+t1875+t1876+t1877+t1878+t1879;
et378 = t1880+t1884+t1885+t1886+t1887+t1888+t1889+t1890+t1891+t1892+t1893+t1894+t1895+t1896+t1897+t1898+t1899+t1900+t1901+t1902+t1903+t1904+t1905+t1906+t1907+t1908+t1909+t1910+t1911+t1912+t1913+t1914+t1915+t1916+t1917+t1918+t1919+t1920+t1921+t1922+t1924+t1925+t1926+t1927+t1934+t1935+t1936+t1937+t1938+t1939+t1940+t1944+t1945+t1946+t1947+t1948+t1949+t1950+t1951+t1952+t1959+t1960+t1961+t1962+t1969+t1970+t1971+t1972+t1973+t1974+t1975+t1981+t1982+t1983+t1984+t1985+t1986+t1987+t1988+t1989+t1990+t1991+t1992+t1993+t1994+t1995+t1996+t1997+t1998+t1999+t2000+t2001+t2002+t2003+t2023+t2024+t2025+t2026+t2027+t2034+t2035+t2036+t2037+t2038+t2039+t2040+t2041+t2042+t2043+t2044+t2045+t2047+t2048+t2049+t2050+t2051+t2061+t2062+t2063+t2064+t2065+t2066+t2067+t2068+t2076+t2077+t2078+t2082+t2083+t2084+t2091+t2092+t2093+t2094+t2096+t2097+t2098+t2099+t2100+t2101+t2102+t2103+t2104+t2105+t2106+t2107+t2108+t2109+t2110+t2111+t2112+t2113+t2114+t2115+t2116+t2117+t2118+t2119+t2120+t2121+t2122+t2123+t2125+t2126+t2127+t2128+t2129+t2130+t2131+t2132+t2133+t2134+t2135+t2136+t2137+t2138+t2139+t2140+t2141+t2142+t2143+t2144+t2145+t2147+t2148+t2149+t2150+t2151+t2152+t2153+t2154+t2155+t2156+t2157+t2158+t2159+t2160+t2161+t2162+t2163;
et379 = t2164+t2165+t2166+t2167+t2168+t2169+t2170+t2171+t2172+t2173+t2174+t2175+t2183+t2184+t2185+t2186+t2187+t2188+t2189+t2190+t2191+t2192+t2193+t2194+t2195+t2196+t2198+t2199+t2200+t2201+t2202+t2203+t2204+t2205+t2206+t2207+t2214+t2215+t2218+t2219+t2220+t2221+t2222+t2223+t2230+t2231+t2232+t2235+t2236+t2237+t2243+t2244+t2245+t2246+t2247+t2248+t2263+t2264+t2265+t2266+t2267+t2268+t2269+t2270+t2271+t2272+t2273+t2274+t2275+t2276+t2277+t2278+t2279+t2280+t2281+t2282+t2283+t2284+t2287+t2288+t2289+t2290+t2291+t2292+t2293+t2294+t2295+t2296+t2297+t2298+t2314+t2315+t2316+t2317+t2318+t2319+t2320+t2321+t2322+t2323+t2324+t2325+t2326+t2327+t2331+t2332+t2333+t2334+t2336+t2337+t2338+t2339+t2340+t2341+t2342+t2343+t2344+t2345+t2346+t2347+t2348+t2353+t2354+t2355+t2360+t2362+t2363+t2364+t2365+t2366+t2367+t2368+t2369+t2370+t2371+t2372+t2373+t2374+t2375+t2376+t2377+t2378+t2383+t2384+t2385+t2386+t2387+t2388+t2389+t2390+t2391+t2392+t2393+t2394+t2395+t2396+t2397+t2398+t2399+t2404+t2405+t2406+t2407+t2408+t2409+t2412+t2413+t2414+t2415+t2416+t2417-Lx2.*Lx3.*dQ2.*dQ3.*m4.*t8.*2.0-Lx2.*Lx3.*dQ2.*dQ3.*m5.*t8.*2.0-Lx2.*Lx3.*dQ2.*dQ3.*m6.*t8.*2.0;
et380 = Lx2.*Lxcm3.*dQ2.*dQ3.*m3.*t8.*-2.0+Lx2.*Lz4.*dQ2.*dQ3.*m5.*t3.*2.0+Lx2.*Lz4.*dQ2.*dQ3.*m6.*t3.*2.0+Lx2.*Lzcm3.*dQ2.*dQ3.*m3.*t3.*2.0+Lx2.*Lzcm4.*dQ2.*dQ3.*m4.*t3.*2.0+Lx2.*Lxcm4.*dQ1.*dQ4.*m4.*t4.*t7.*2.0-Lx2.*Lxcm4.*dQ2.*dQ3.*m4.*t4.*t8.*2.0-Lx2.*Lxcm4.*dQ2.*dQ4.*m4.*t3.*t9.*2.0-Lx2.*Lxcm4.*dQ3.*dQ4.*m4.*t3.*t9.*2.0-Lx2.*Lxcm5.*dQ2.*dQ3.*m5.*t3.*t10.*2.0-Lx2.*Lxcm5.*dQ2.*dQ5.*m5.*t5.*t8.*2.0-Lx2.*Lxcm5.*dQ3.*dQ5.*m5.*t5.*t8.*2.0-Lx2.*Lycm4.*dQ2.*dQ4.*m4.*t3.*t4.*2.0-Lx2.*Lycm4.*dQ3.*dQ4.*m4.*t3.*t4.*2.0-Lx2.*Lycm5.*dQ2.*dQ4.*m5.*t3.*t4.*2.0-Lx2.*Lycm5.*dQ3.*dQ4.*m5.*t3.*t4.*2.0-Lx2.*Lycm4.*dQ1.*dQ4.*m4.*t7.*t9.*2.0+Lx2.*Lycm4.*dQ2.*dQ3.*m4.*t8.*t9.*2.0-Lx2.*Lycm5.*dQ1.*dQ4.*m5.*t7.*t9.*2.0+Lx2.*Lycm5.*dQ2.*dQ3.*m5.*t8.*t9.*2.0+Lx2.*Lz5.*dQ2.*dQ3.*m6.*t3.*t5.*2.0;
et381 = Lx2.*Lz5.*dQ2.*dQ5.*m6.*t8.*t10.*-2.0-Lx2.*Lz5.*dQ3.*dQ5.*m6.*t8.*t10.*2.0+Lx2.*Lzcm5.*dQ2.*dQ3.*m5.*t3.*t5.*2.0+Lx2.*Lzcm6.*dQ2.*dQ3.*m6.*t3.*t5.*2.0-Lx2.*Lzcm5.*dQ2.*dQ5.*m5.*t8.*t10.*2.0-Lx2.*Lzcm5.*dQ3.*dQ5.*m5.*t8.*t10.*2.0-Lx2.*Lzcm6.*dQ2.*dQ5.*m6.*t8.*t10.*2.0-Lx2.*Lzcm6.*dQ3.*dQ5.*m6.*t8.*t10.*2.0+Lx2.*Lxcm5.*dQ1.*dQ4.*m5.*t4.*t5.*t7.*2.0-Lx2.*Lxcm5.*dQ2.*dQ3.*m5.*t4.*t5.*t8.*2.0-Lx2.*Lxcm5.*dQ2.*dQ4.*m5.*t3.*t5.*t9.*2.0-Lx2.*Lxcm5.*dQ2.*dQ5.*m5.*t3.*t4.*t10.*2.0-Lx2.*Lxcm5.*dQ3.*dQ4.*m5.*t3.*t5.*t9.*2.0-Lx2.*Lxcm5.*dQ3.*dQ5.*m5.*t3.*t4.*t10.*2.0+Lx2.*Lxcm6.*dQ1.*dQ6.*m6.*t4.*t6.*t7.*2.0-Lx2.*Lxcm6.*dQ2.*dQ3.*m6.*t3.*t6.*t10.*2.0-Lx2.*Lxcm6.*dQ2.*dQ4.*m6.*t3.*t4.*t11.*2.0-Lx2.*Lxcm6.*dQ3.*dQ4.*m6.*t3.*t4.*t11.*2.0-Lx2.*Lxcm6.*dQ2.*dQ5.*m6.*t5.*t6.*t8.*2.0;
et382 = Lx2.*Lxcm6.*dQ2.*dQ6.*m6.*t3.*t6.*t9.*-2.0-Lx2.*Lxcm6.*dQ3.*dQ5.*m6.*t5.*t6.*t8.*2.0-Lx2.*Lxcm6.*dQ3.*dQ6.*m6.*t3.*t6.*t9.*2.0-Lx2.*Lxcm6.*dQ4.*dQ6.*m6.*t4.*t6.*t8.*2.0-Lx2.*Lxcm5.*dQ1.*dQ5.*m5.*t7.*t9.*t10.*2.0-Lx2.*Lxcm6.*dQ5.*dQ6.*m6.*t3.*t5.*t11.*2.0-Lx2.*Lxcm6.*dQ1.*dQ4.*m6.*t7.*t9.*t11.*2.0+Lx2.*Lxcm6.*dQ2.*dQ3.*m6.*t8.*t9.*t11.*2.0+Lx2.*Lxcm5.*dQ4.*dQ5.*m5.*t8.*t9.*t10.*2.0+Lx2.*Lxcm6.*dQ2.*dQ6.*m6.*t8.*t10.*t11.*2.0+Lx2.*Lxcm6.*dQ3.*dQ6.*m6.*t8.*t10.*t11.*2.0-Lx2.*Lycm6.*dQ2.*dQ4.*m6.*t3.*t4.*t6.*2.0-Lx2.*Lycm6.*dQ3.*dQ4.*m6.*t3.*t4.*t6.*2.0-Lx2.*Lycm6.*dQ5.*dQ6.*m6.*t3.*t5.*t6.*2.0-Lx2.*Lycm6.*dQ1.*dQ4.*m6.*t6.*t7.*t9.*2.0+Lx2.*Lycm6.*dQ2.*dQ3.*m6.*t6.*t8.*t9.*2.0-Lx2.*Lycm6.*dQ1.*dQ6.*m6.*t4.*t7.*t11.*2.0+Lx2.*Lycm6.*dQ2.*dQ3.*m6.*t3.*t10.*t11.*2.0;
et383 = Lx2.*Lycm6.*dQ2.*dQ5.*m6.*t5.*t8.*t11.*2.0+Lx2.*Lycm6.*dQ2.*dQ6.*m6.*t3.*t9.*t11.*2.0+Lx2.*Lycm6.*dQ2.*dQ6.*m6.*t6.*t8.*t10.*2.0+Lx2.*Lycm6.*dQ3.*dQ5.*m6.*t5.*t8.*t11.*2.0+Lx2.*Lycm6.*dQ3.*dQ6.*m6.*t3.*t9.*t11.*2.0+Lx2.*Lycm6.*dQ3.*dQ6.*m6.*t6.*t8.*t10.*2.0+Lx2.*Lycm6.*dQ4.*dQ6.*m6.*t4.*t8.*t11.*2.0+Lx2.*Lz5.*dQ2.*dQ5.*m6.*t3.*t4.*t5.*2.0+Lx2.*Lz5.*dQ3.*dQ5.*m6.*t3.*t4.*t5.*2.0+Lx2.*Lz5.*dQ1.*dQ4.*m6.*t4.*t7.*t10.*2.0+Lx2.*Lz5.*dQ1.*dQ5.*m6.*t5.*t7.*t9.*2.0-Lx2.*Lz5.*dQ2.*dQ3.*m6.*t4.*t8.*t10.*2.0-Lx2.*Lz5.*dQ2.*dQ4.*m6.*t3.*t9.*t10.*2.0-Lx2.*Lz5.*dQ3.*dQ4.*m6.*t3.*t9.*t10.*2.0-Lx2.*Lz5.*dQ4.*dQ5.*m6.*t5.*t8.*t9.*2.0+Lx2.*Lzcm5.*dQ2.*dQ5.*m5.*t3.*t4.*t5.*2.0+Lx2.*Lzcm5.*dQ3.*dQ5.*m5.*t3.*t4.*t5.*2.0+Lx2.*Lzcm6.*dQ2.*dQ5.*m6.*t3.*t4.*t5.*2.0+Lx2.*Lzcm6.*dQ3.*dQ5.*m6.*t3.*t4.*t5.*2.0;
et384 = Lx2.*Lzcm5.*dQ1.*dQ4.*m5.*t4.*t7.*t10.*2.0+Lx2.*Lzcm5.*dQ1.*dQ5.*m5.*t5.*t7.*t9.*2.0-Lx2.*Lzcm5.*dQ2.*dQ3.*m5.*t4.*t8.*t10.*2.0-Lx2.*Lzcm5.*dQ2.*dQ4.*m5.*t3.*t9.*t10.*2.0+Lx2.*Lzcm6.*dQ1.*dQ4.*m6.*t4.*t7.*t10.*2.0-Lx2.*Lzcm5.*dQ3.*dQ4.*m5.*t3.*t9.*t10.*2.0+Lx2.*Lzcm6.*dQ1.*dQ5.*m6.*t5.*t7.*t9.*2.0-Lx2.*Lzcm6.*dQ2.*dQ3.*m6.*t4.*t8.*t10.*2.0-Lx2.*Lzcm6.*dQ2.*dQ4.*m6.*t3.*t9.*t10.*2.0-Lx2.*Lzcm5.*dQ4.*dQ5.*m5.*t5.*t8.*t9.*2.0-Lx2.*Lzcm6.*dQ3.*dQ4.*m6.*t3.*t9.*t10.*2.0-Lx2.*Lzcm6.*dQ4.*dQ5.*m6.*t5.*t8.*t9.*2.0+Lx2.*Lxcm6.*dQ1.*dQ4.*m6.*t4.*t5.*t6.*t7.*2.0-Lx2.*Lxcm6.*dQ2.*dQ3.*m6.*t4.*t5.*t6.*t8.*2.0-Lx2.*Lxcm6.*dQ2.*dQ4.*m6.*t3.*t5.*t6.*t9.*2.0-Lx2.*Lxcm6.*dQ2.*dQ5.*m6.*t3.*t4.*t6.*t10.*2.0-Lx2.*Lxcm6.*dQ3.*dQ4.*m6.*t3.*t5.*t6.*t9.*2.0-Lx2.*Lxcm6.*dQ2.*dQ6.*m6.*t3.*t4.*t5.*t11.*2.0;
et385 = Lx2.*Lxcm6.*dQ3.*dQ5.*m6.*t3.*t4.*t6.*t10.*-2.0-Lx2.*Lxcm6.*dQ3.*dQ6.*m6.*t3.*t4.*t5.*t11.*2.0-Lx2.*Lxcm6.*dQ1.*dQ5.*m6.*t6.*t7.*t9.*t10.*2.0-Lx2.*Lxcm6.*dQ1.*dQ6.*m6.*t5.*t7.*t9.*t11.*2.0+Lx2.*Lxcm6.*dQ4.*dQ5.*m6.*t6.*t8.*t9.*t10.*2.0+Lx2.*Lxcm6.*dQ4.*dQ6.*m6.*t5.*t8.*t9.*t11.*2.0+Lx2.*Lxcm6.*dQ5.*dQ6.*m6.*t4.*t8.*t10.*t11.*2.0-Lx2.*Lycm6.*dQ2.*dQ6.*m6.*t3.*t4.*t5.*t6.*2.0-Lx2.*Lycm6.*dQ3.*dQ6.*m6.*t3.*t4.*t5.*t6.*2.0-Lx2.*Lycm6.*dQ1.*dQ4.*m6.*t4.*t5.*t7.*t11.*2.0+Lx2.*Lycm6.*dQ2.*dQ3.*m6.*t4.*t5.*t8.*t11.*2.0-Lx2.*Lycm6.*dQ1.*dQ6.*m6.*t5.*t6.*t7.*t9.*2.0+Lx2.*Lycm6.*dQ2.*dQ4.*m6.*t3.*t5.*t9.*t11.*2.0+Lx2.*Lycm6.*dQ2.*dQ5.*m6.*t3.*t4.*t10.*t11.*2.0+Lx2.*Lycm6.*dQ3.*dQ4.*m6.*t3.*t5.*t9.*t11.*2.0+Lx2.*Lycm6.*dQ3.*dQ5.*m6.*t3.*t4.*t10.*t11.*2.0+Lx2.*Lycm6.*dQ4.*dQ6.*m6.*t5.*t6.*t8.*t9.*2.0;
et386 = Lx2.*Lycm6.*dQ5.*dQ6.*m6.*t4.*t6.*t8.*t10.*2.0+Lx2.*Lycm6.*dQ1.*dQ5.*m6.*t7.*t9.*t10.*t11.*2.0-Lx2.*Lycm6.*dQ4.*dQ5.*m6.*t8.*t9.*t10.*t11.*2.0;
et387 = t42+t43+t44+t45+t46+t47+t48+t49+t50+t51+t54+t55+t56+t57+t58+t61+t62+t63+t64+t67+t68+t69+t72+t73+t78+t79+t80+t81+t82+t83+t84+t85+t86+t87+t88+t89+t90+t91+t92+t93+t94+t96+t100+t102+t106+t107+t118+t119+t120+t121+t122+t123+t124+t125+t126+t127+t128+t129+t132+t138+t139+t141+t142+t143+t144+t145+t146+t147+t148+t149+t150+t151+t152+t153+t154+t155+t156+t157+t170+t171+t174+t177+t178+t179+t180+t185+t186+t201+t202+t203+t204+t205+t206+t207+t208+t209+t210+t211+t212+t213+t214+t215+t216+t217+t218+t219+t220+t222+t225+t227+t228+t229+t230+t231+t232+t233+t234+t235+t236+t237+t242+t243+t244+t245+t250+t251+t252+t253+t258+t259+t260+t263+t264+t265+t266+t269+t270+t273+t274+t276+t277+t278+t279+t282+t283+t286+t287+t289+t290+t292+t293+t297+t298+t299+t300+t301+t302+t303+t304+t305+t306+t307+t308+t309+t310+t311+t312+t313+t314+t315+t316+t317+t318+t319+t320+t321+t322+t323+t324+t325+t326+t327+t328+t331+t332+t333+t334+t340+t341+t342+t343+t349+t351+t358+t363+t364+t367+t368+t369+t370;
et388 = t377+t378+t379+t380+t381+t382+t383+t384+t385+t386+t402+t403+t404+t405+t406+t407+t415+t416+t417+t418+t419+t430+t431+t432+t433+t434+t435+t436+t437+t438+t442+t443+t444+t445+t446+t447+t454+t455+t456+t457+t458+t459+t460+t461+t462+t463+t464+t465+t466+t467+t468+t469+t470+t471+t472+t473+t474+t475+t476+t477+t478+t479+t480+t481+t482+t483+t484+t485+t486+t487+t488+t489+t490+t491+t492+t493+t494+t495+t496+t497+t498+t500+t506+t512+t514+t515+t516+t527+t528+t529+t540+t542+t543+t544+t546+t547+t548+t550+t552+t554+t555+t556+t557+t558+t559+t560+t561+t562+t563+t564+t565+t566+t567+t568+t569+t570+t571+t572+t573+t574+t575+t576+t577+t578+t579+t580+t581+t582+t583+t584+t585+t586+t587+t588+t589+t590+t591+t592+t593+t594+t595+t596+t597+t598+t599+t600+t601+t602+t603+t604+t605+t606+t607+t608+t609+t610+t611+t612+t613+t614+t615+t616+t617+t618+t619+t620+t621+t622+t623+t624+t625+t626+t627+t628+t629+t630+t631+t632+t635+t636+t637+t638+t648+t650+t651+t658+t659+t660+t661+t662+t663+t664+t669+t670+t671+t674+t675+t676+t677+t681;
et389 = t684+t687+t688+t689+t690+t694+t697+t698+t699+t700+t701+t702+t703+t704+t705+t706+t707+t708+t709+t710+t711+t716+t717+t718+t719+t720+t721+t724+t725+t728+t729+t730+t731+t732+t733+t734+t735+t737+t738+t739+t746+t748+t749+t750+t752+t754+t755+t756+t759+t760+t761+t762+t774+t775+t776+t777+t778+t779+t780+t781+t782+t783+t785+t788+t791+t792+t793+t794+t795+t798+t800+t801+t803+t804+t806+t807+t809+t810+t828+t829+t830+t831+t832+t833+t834+t835+t836+t837+t838+t839+t840+t843+t844+t845+t848+t849+t851+t852+t857+t858+t861+t862+t868+t869+t870+t871+t872+t873+t874+t875+t876+t877+t878+t879+t880+t881+t882+t883+t884+t885+t886+t887+t888+t889+t890+t891+t892+t893+t894+t895+t896+t897+t898+t899+t900+t901+t902+t903+t904+t905+t906+t907+t908+t909+t910+t911+t912+t913+t914+t915+t916+t917+t918+t919+t920+t921+t922+t923+t924+t925+t926+t927+t928+t929+t930+t931+t932+t933+t934+t935+t936+t938+t939+t940+t941+t942+t943+t950+t951+t952+t953+t954+t955+t956+t957+t958+t959+t960+t961+t962+t963+t964+t965+t966+t967+t968+t969+t972+t973+t978;
et390 = t979+t984+t985+t988+t989+t990+t991+t992+t993+t994+t995+t996+t997+t998+t1001+t1002+t1003+t1004+t1005+t1006+t1007+t1008+t1009+t1010+t1011+t1012+t1013+t1014+t1015+t1016+t1017+t1018+t1019+t1020+t1021+t1022+t1023+t1024+t1025+t1026+t1027+t1028+t1029+t1030+t1033+t1034+t1035+t1036+t1037+t1038+t1039+t1041+t1046+t1060+t1061+t1062+t1063+t1064+t1065+t1066+t1067+t1072+t1073+t1074+t1075+t1076+t1077+t1078+t1079+t1082+t1083+t1084+t1085+t1093+t1094+t1095+t1096+t1097+t1098+t1099+t1103+t1104+t1105+t1106+t1107+t1108+t1109+t1110+t1111+t1112+t1113+t1114+t1115+t1116+t1117+t1118+t1120+t1127+t1139+t1140+t1145+t1146+t1147+t1148+t1149+t1150+t1154+t1155+t1158+t1159+t1167+t1169+t1170+t1173+t1174+t1175+t1177+t1178+t1179+t1180+t1181+t1182+t1187+t1193+t1194+t1197+t1198+t1199+t1200+t1202+t1204+t1205+t1206+t1208+t1213+t1214+t1215+t1216+t1217+t1218+t1219+t1223+t1224+t1225+t1226+t1227+t1228+t1229+t1230+t1231+t1242+t1243+t1246+t1249+t1250+t1251+t1252+t1253+t1254+t1255+t1256+t1257+t1258+t1259+t1262+t1263+t1264+t1265+t1266+t1269+t1272+t1275+t1276+t1278+t1279+t1283+t1285+t1286+t1287+t1288+t1289+t1290+t1291+t1292+t1293+t1294+t1295+t1296+t1297+t1298+t1299+t1300+t1301+t1302+t1303+t1304+t1305+t1306+t1307+t1308;
et391 = t1309+t1310+t1311+t1312+t1313+t1314+t1315+t1316+t1317+t1318+t1319+t1320+t1321+t1322+t1323+t1324+t1325+t1326+t1327+t1328+t1329+t1330+t1331+t1332+t1333+t1334+t1335+t1336+t1337+t1338+t1339+t1340+t1341+t1342+t1343+t1344+t1345+t1346+t1347+t1348+t1349+t1350+t1351+t1352+t1353+t1354+t1355+t1356+t1357+t1358+t1359+t1360+t1361+t1362+t1363+t1364+t1365+t1366+t1367+t1368+t1369+t1370+t1371+t1372+t1373+t1374+t1375+t1376+t1377+t1378+t1379+t1381+t1382+t1383+t1384+t1385+t1386+t1387+t1388+t1389+t1390+t1391+t1392+t1393+t1394+t1395+t1396+t1397+t1398+t1399+t1400+t1401+t1402+t1403+t1404+t1405+t1406+t1407+t1408+t1409+t1410+t1411+t1420+t1421+t1422+t1423+t1424+t1425+t1426+t1427+t1428+t1429+t1430+t1431+t1432+t1433+t1434+t1435+t1436+t1437+t1438+t1439+t1440+t1441+t1442+t1443+t1444+t1445+t1446+t1447+t1448+t1449+t1450+t1451+t1452+t1453+t1454+t1455+t1456+t1457+t1458+t1469+t1471+t1472+t1474+t1475+t1481+t1482+t1484+t1487+t1490+t1493+t1496+t1497+t1498+t1499+t1500+t1501+t1502+t1503+t1504+t1505+t1506+t1507+t1508+t1509+t1510+t1511+t1512+t1513+t1514+t1515+t1516+t1517+t1518+t1519+t1520+t1521+t1522+t1523+t1524+t1525+t1526+t1531+t1532+t1533+t1534+t1535+t1536+t1539+t1540+t1547+t1548+t1549+t1550+t1555+t1560+t1561+t1562+t1565;
et392 = t1566+t1575+t1576+t1577+t1578+t1579+t1580+t1581+t1582+t1583+t1589+t1590+t1591+t1592+t1593+t1594+t1595+t1596+t1597+t1600+t1601+t1602+t1603+t1604+t1605+t1610+t1613+t1617+t1618+t1619+t1627+t1628+t1629+t1630+t1631+t1632+t1633+t1634+t1637+t1639+t1640+t1641+t1642+t1643+t1644+t1645+t1646+t1647+t1648+t1649+t1650+t1651+t1652+t1653+t1654+t1655+t1656+t1657+t1658+t1659+t1660+t1661+t1662+t1663+t1664+t1665+t1672+t1673+t1674+t1675+t1676+t1677+t1678+t1679+t1680+t1683+t1684+t1687+t1688+t1691+t1694+t1695+t1696+t1697+t1698+t1699+t1700+t1721+t1722+t1725+t1726+t1730+t1731+t1733+t1734+t1735+t1736+t1740+t1744+t1745+t1754+t1755+t1756+t1759+t1760+t1761+t1762+t1763+t1764+t1765+t1766+t1767+t1768+t1769+t1770+t1771+t1772+t1773+t1774+t1775+t1777+t1778+t1779+t1780+t1781+t1782+t1783+t1784+t1785+t1786+t1787+t1788+t1789+t1790+t1791+t1792+t1793+t1794+t1795+t1796+t1797+t1798+t1799+t1800+t1801+t1802+t1803+t1804+t1814+t1815+t1816+t1817+t1818+t1819+t1820+t1821+t1822+t1823+t1827+t1828+t1829+t1830+t1831+t1832+t1833+t1834+t1835+t1840+t1841+t1847+t1850+t1851+t1852+t1853+t1854+t1855+t1856+t1857+t1858+t1859+t1860+t1861+t1862+t1863+t1864+t1865+t1866+t1867+t1868+t1869+t1870+t1871+t1872+t1873+t1874+t1875+t1876+t1877+t1878+t1879;
et393 = t1880+t1884+t1885+t1886+t1887+t1888+t1889+t1890+t1891+t1892+t1893+t1894+t1895+t1896+t1897+t1898+t1899+t1900+t1901+t1902+t1903+t1904+t1905+t1906+t1907+t1908+t1909+t1910+t1911+t1912+t1913+t1914+t1915+t1916+t1917+t1918+t1919+t1920+t1921+t1922+t1924+t1925+t1926+t1927+t1934+t1935+t1936+t1937+t1938+t1939+t1940+t1944+t1945+t1946+t1947+t1948+t1949+t1950+t1951+t1952+t1959+t1960+t1961+t1962+t1969+t1970+t1971+t1972+t1973+t1974+t1975+t1981+t1982+t1983+t1984+t1985+t1986+t1987+t1988+t1989+t1990+t1991+t1992+t1993+t1994+t1995+t1996+t1997+t1998+t1999+t2000+t2001+t2002+t2003+t2023+t2024+t2025+t2026+t2027+t2034+t2035+t2036+t2037+t2038+t2039+t2040+t2041+t2042+t2043+t2044+t2045+t2047+t2048+t2049+t2050+t2051+t2061+t2062+t2063+t2064+t2065+t2066+t2067+t2068+t2076+t2077+t2078+t2082+t2083+t2084+t2091+t2092+t2093+t2094+t2096+t2097+t2098+t2099+t2100+t2101+t2102+t2103+t2104+t2105+t2106+t2107+t2108+t2109+t2110+t2111+t2112+t2113+t2114+t2115+t2116+t2117+t2118+t2119+t2120+t2121+t2122+t2123+t2125+t2126+t2127+t2128+t2129+t2130+t2131+t2132+t2133+t2134+t2135+t2136+t2137+t2138+t2139+t2140+t2141+t2142+t2143+t2144+t2145+t2147+t2148+t2149+t2150+t2151+t2152+t2153+t2154+t2155+t2156+t2157+t2158+t2159+t2160+t2161+t2162+t2163;
et394 = t2164+t2165+t2166+t2167+t2168+t2169+t2170+t2171+t2172+t2173+t2174+t2175+t2183+t2184+t2185+t2186+t2187+t2188+t2189+t2190+t2191+t2192+t2193+t2194+t2195+t2196+t2198+t2199+t2200+t2201+t2202+t2203+t2204+t2205+t2206+t2207+t2214+t2215+t2218+t2219+t2220+t2221+t2222+t2223+t2230+t2231+t2232+t2235+t2236+t2237+t2243+t2244+t2245+t2246+t2247+t2248+t2263+t2264+t2265+t2266+t2267+t2268+t2269+t2270+t2271+t2272+t2273+t2274+t2275+t2276+t2277+t2278+t2279+t2280+t2281+t2282+t2283+t2284+t2287+t2288+t2289+t2290+t2291+t2292+t2293+t2294+t2295+t2296+t2297+t2298+t2314+t2315+t2316+t2317+t2318+t2319+t2320+t2321+t2322+t2323+t2324+t2325+t2326+t2327+t2331+t2332+t2333+t2334+t2336+t2337+t2338+t2339+t2340+t2341+t2342+t2343+t2344+t2345+t2346+t2347+t2348+t2353+t2354+t2355+t2360+t2362+t2363+t2364+t2365+t2366+t2367+t2368+t2369+t2370+t2371+t2372+t2373+t2374+t2375+t2376+t2377+t2378+t2383+t2384+t2385+t2386+t2387+t2388+t2389+t2390+t2391+t2392+t2393+t2394+t2395+t2396+t2397+t2398+t2399+t2404+t2405+t2406+t2407+t2408+t2409+t2412+t2413+t2414+t2415+t2416+t2417;
et395 = -Ixy4.*dQ2.*dQ3-Ixy6.*dQ4.*dQ6-Ixz5.*dQ4.*dQ5-Iyx4.*dQ2.*dQ3-Iyx6.*dQ4.*dQ6-Izx5.*dQ4.*dQ5+t5.*t9.*t10.*t44.*2.0+t5.*t9.*t10.*t45.*2.0+t5.*t9.*t10.*t48.*2.0+t5.*t9.*t10.*t49.*2.0+t5.*t9.*t10.*t55.*2.0+t5.*t9.*t10.*t56.*2.0+t5.*t9.*t10.*t62.*2.0+t5.*t9.*t10.*t63.*2.0-t5.*t9.*t10.*t70.*2.0-t5.*t9.*t10.*t71.*2.0-t5.*t9.*t10.*t74.*2.0-t5.*t9.*t10.*t75.*2.0+Ixx5.*dQ2.*dQ5.*t9+Ixx5.*dQ3.*dQ5.*t9+Ixx6.*dQ2.*dQ5.*t9+Ixx6.*dQ3.*dQ5.*t9+Ixx6.*dQ5.*dQ6.*t10-Ixx4.*dQ2.*dQ3.*t39+Ixx6.*dQ2.*dQ3.*t39+Ixx5.*dQ4.*dQ5.*t40-Ixx6.*dQ4.*dQ6.*t41-Ixy5.*dQ2.*dQ3.*t5+Ixy6.*dQ2.*dQ3.*t5+Ixy4.*dQ2.*dQ3.*t34.*2.0+Ixy6.*dQ4.*dQ6.*t35+Ixy6.*dQ4.*dQ6.*t36.*2.0-Ixz6.*dQ4.*dQ5.*t6;
et396 = Ixz5.*dQ4.*dQ5.*t35.*2.0-Iyx5.*dQ2.*dQ3.*t5+Iyx6.*dQ2.*dQ3.*t5+Iyx4.*dQ2.*dQ3.*t34.*2.0+Iyx6.*dQ4.*dQ6.*t35+Iyx6.*dQ4.*dQ6.*t36.*2.0+Iyy5.*dQ2.*dQ5.*t9+Iyy5.*dQ3.*dQ5.*t9+Iyy6.*dQ2.*dQ5.*t9+Iyy6.*dQ3.*dQ5.*t9-Iyy6.*dQ5.*dQ6.*t10+Iyy4.*dQ2.*dQ3.*t39+Iyy5.*dQ2.*dQ3.*t39+Iyy6.*dQ4.*dQ5.*t40+Iyy6.*dQ4.*dQ6.*t41-Iyz5.*dQ2.*dQ3.*t10+Iyz6.*dQ4.*dQ5.*t11-Izx6.*dQ4.*dQ5.*t6+Izx5.*dQ4.*dQ5.*t35.*2.0-Izy5.*dQ2.*dQ3.*t10+Izy6.*dQ4.*dQ5.*t11-Izz5.*dQ2.*dQ5.*t9-Izz5.*dQ3.*dQ5.*t9-Izz6.*dQ2.*dQ5.*t9-Izz6.*dQ3.*dQ5.*t9-Izz6.*dQ5.*dQ6.*t10-Izz5.*dQ2.*dQ3.*t39-Izz6.*dQ2.*dQ3.*t39-Izz5.*dQ4.*dQ5.*t40-Izz6.*dQ4.*dQ5.*t40-Lxcm4.*Lycm4.*dQ2.*dQ3.*m4.*2.0-Lxcm6.*Lycm6.*dQ4.*dQ6.*m6.*2.0;
et397 = Lxcm5.*Lzcm5.*dQ4.*dQ5.*m5.*-2.0-Ixx4.*dQ1.*dQ2.*t2.*t8-Ixx4.*dQ1.*dQ2.*t3.*t7-Ixx4.*dQ1.*dQ3.*t2.*t8-Ixx4.*dQ1.*dQ3.*t3.*t7-Ixx5.*dQ1.*dQ2.*t2.*t8-Ixx5.*dQ1.*dQ2.*t3.*t7-Ixx5.*dQ1.*dQ3.*t2.*t8-Ixx5.*dQ1.*dQ3.*t3.*t7+Ixx6.*dQ1.*dQ2.*t2.*t8+Ixx6.*dQ1.*dQ2.*t3.*t7+Ixx6.*dQ1.*dQ3.*t2.*t8+Ixx6.*dQ1.*dQ3.*t3.*t7+Ixx6.*dQ2.*dQ6.*t4.*t10+Ixx6.*dQ3.*dQ6.*t4.*t10-Ixx5.*dQ2.*dQ5.*t9.*t35.*2.0-Ixx5.*dQ3.*dQ5.*t9.*t35.*2.0-Ixx6.*dQ5.*dQ6.*t10.*t36.*2.0-Ixy6.*dQ1.*dQ6.*t2.*t3+Ixy5.*dQ2.*dQ5.*t4.*t5+Ixy5.*dQ3.*dQ5.*t4.*t5-Ixy6.*dQ2.*dQ5.*t4.*t5-Ixy6.*dQ3.*dQ5.*t4.*t5+Ixy6.*dQ1.*dQ6.*t7.*t8+Ixy5.*dQ2.*dQ3.*t5.*t34.*2.0-Ixy6.*dQ2.*dQ3.*t5.*t34.*2.0-Ixy6.*dQ2.*dQ3.*t5.*t36.*2.0;
et398 = Ixy6.*dQ4.*dQ6.*t35.*t36.*-2.0-Ixz5.*dQ1.*dQ5.*t2.*t3+Ixz5.*dQ1.*dQ5.*t7.*t8-Ixz6.*dQ2.*dQ3.*t10.*t11-Ixz6.*dQ2.*dQ6.*t9.*t11-Ixz6.*dQ3.*dQ6.*t9.*t11+Ixz6.*dQ4.*dQ5.*t6.*t35.*2.0-Iyx6.*dQ1.*dQ6.*t2.*t3+Iyx5.*dQ2.*dQ5.*t4.*t5+Iyx5.*dQ3.*dQ5.*t4.*t5-Iyx6.*dQ2.*dQ5.*t4.*t5-Iyx6.*dQ3.*dQ5.*t4.*t5+Iyx6.*dQ1.*dQ6.*t7.*t8+Iyx5.*dQ2.*dQ3.*t5.*t34.*2.0-Iyx6.*dQ2.*dQ3.*t5.*t34.*2.0-Iyx6.*dQ2.*dQ3.*t5.*t36.*2.0-Iyx6.*dQ4.*dQ6.*t35.*t36.*2.0+Iyy4.*dQ1.*dQ2.*t2.*t8+Iyy4.*dQ1.*dQ2.*t3.*t7+Iyy4.*dQ1.*dQ3.*t2.*t8+Iyy4.*dQ1.*dQ3.*t3.*t7+Iyy5.*dQ1.*dQ2.*t2.*t8+Iyy5.*dQ1.*dQ2.*t3.*t7+Iyy5.*dQ1.*dQ3.*t2.*t8+Iyy5.*dQ1.*dQ3.*t3.*t7-Iyy6.*dQ1.*dQ2.*t2.*t8-Iyy6.*dQ1.*dQ2.*t3.*t7-Iyy6.*dQ1.*dQ3.*t2.*t8;
et399 = -Iyy6.*dQ1.*dQ3.*t3.*t7-Iyy6.*dQ2.*dQ6.*t4.*t10-Iyy6.*dQ3.*dQ6.*t4.*t10-Iyy6.*dQ2.*dQ5.*t9.*t35.*2.0-Iyy6.*dQ3.*dQ5.*t9.*t35.*2.0+Iyy6.*dQ5.*dQ6.*t10.*t36.*2.0+Iyz5.*dQ2.*dQ5.*t4.*t10+Iyz5.*dQ3.*dQ5.*t4.*t10-Iyz6.*dQ2.*dQ3.*t6.*t10-Iyz6.*dQ2.*dQ6.*t6.*t9-Iyz6.*dQ3.*dQ6.*t6.*t9+Iyz5.*dQ2.*dQ3.*t10.*t34.*2.0-Iyz6.*dQ4.*dQ5.*t11.*t35.*2.0-Izx5.*dQ1.*dQ5.*t2.*t3+Izx5.*dQ1.*dQ5.*t7.*t8-Izx6.*dQ2.*dQ3.*t10.*t11-Izx6.*dQ2.*dQ6.*t9.*t11-Izx6.*dQ3.*dQ6.*t9.*t11+Izx6.*dQ4.*dQ5.*t6.*t35.*2.0+Izy5.*dQ2.*dQ5.*t4.*t10+Izy5.*dQ3.*dQ5.*t4.*t10-Izy6.*dQ2.*dQ3.*t6.*t10-Izy6.*dQ2.*dQ6.*t6.*t9-Izy6.*dQ3.*dQ6.*t6.*t9+Izy5.*dQ2.*dQ3.*t10.*t34.*2.0-Izy6.*dQ4.*dQ5.*t11.*t35.*2.0;
et400 = -Izz4.*dQ1.*dQ2.*t2.*t8-Izz4.*dQ1.*dQ2.*t3.*t7-Izz4.*dQ1.*dQ3.*t2.*t8-Izz4.*dQ1.*dQ3.*t3.*t7-Izz5.*dQ1.*dQ2.*t2.*t8-Izz5.*dQ1.*dQ2.*t3.*t7-Izz5.*dQ1.*dQ3.*t2.*t8-Izz5.*dQ1.*dQ3.*t3.*t7-Izz6.*dQ1.*dQ2.*t2.*t8-Izz6.*dQ1.*dQ2.*t3.*t7-Izz6.*dQ1.*dQ3.*t2.*t8-Izz6.*dQ1.*dQ3.*t3.*t7-Izz6.*dQ2.*dQ6.*t4.*t10-Izz6.*dQ3.*dQ6.*t4.*t10+Izz5.*dQ2.*dQ5.*t9.*t35.*2.0+Izz5.*dQ3.*dQ5.*t9.*t35.*2.0+Izz6.*dQ2.*dQ5.*t9.*t35.*2.0+Izz6.*dQ3.*dQ5.*t9.*t35.*2.0+dQ2.*dQ5.*m6.*t9.*t22.*2.0-dQ5.*dQ6.*m6.*t10.*t17.*2.0+dQ3.*dQ5.*m6.*t9.*t22.*2.0+dQ2.*dQ5.*m5.*t9.*t25.*2.0+dQ3.*dQ5.*m5.*t9.*t25.*2.0+dQ2.*dQ5.*m6.*t9.*t26.*2.0+dQ3.*dQ5.*m6.*t9.*t26.*2.0+dQ2.*dQ3.*m4.*t15.*t39;
et401 = -dQ2.*dQ3.*m4.*t18.*t39-dQ2.*dQ3.*m6.*t17.*t39-dQ2.*dQ3.*m5.*t19.*t39-dQ4.*dQ5.*m5.*t16.*t40+dQ2.*dQ3.*m6.*t22.*t39+dQ2.*dQ3.*m5.*t25.*t39+dQ4.*dQ6.*m6.*t17.*t41-dQ4.*dQ5.*m6.*t20.*t40+dQ2.*dQ3.*m6.*t26.*t39+dQ4.*dQ5.*m6.*t22.*t40-dQ4.*dQ6.*m6.*t20.*t41+dQ4.*dQ5.*m5.*t25.*t40+dQ4.*dQ5.*m6.*t26.*t40-t4.*t6.*t10.*t11.*t239.*2.0-t4.*t6.*t10.*t11.*t240.*2.0+t4.*t6.*t10.*t11.*t243.*2.0+t4.*t6.*t10.*t11.*t244.*2.0+t4.*t6.*t10.*t11.*t938+t4.*t6.*t10.*t11.*t939+Lx3.*Lxcm4.*dQ2.*dQ3.*m4.*t9.*2.0+Lx3.*Lycm4.*dQ2.*dQ3.*m4.*t4.*2.0+Lx3.*Lycm5.*dQ2.*dQ3.*m5.*t4.*2.0-Lxcm5.*Lycm5.*dQ2.*dQ3.*m5.*t5.*2.0+Lxcm6.*Lycm6.*dQ2.*dQ3.*m6.*t5.*2.0+Lxcm4.*Lycm4.*dQ2.*dQ3.*m4.*t34.*4.0+Lxcm6.*Lycm6.*dQ4.*dQ6.*m6.*t35.*2.0+Lxcm6.*Lycm6.*dQ4.*dQ6.*m6.*t36.*4.0;
et402 = Lxcm6.*Lz5.*dQ4.*dQ5.*m6.*t6.*-2.0-Lxcm6.*Lzcm6.*dQ4.*dQ5.*m6.*t6.*2.0+Lxcm5.*Lzcm5.*dQ4.*dQ5.*m5.*t35.*4.0+Lycm6.*Lz5.*dQ4.*dQ5.*m6.*t11.*2.0-Lycm5.*Lzcm5.*dQ2.*dQ3.*m5.*t10.*2.0+Lycm6.*Lzcm6.*dQ4.*dQ5.*m6.*t11.*2.0+Lz5.*Lzcm6.*dQ2.*dQ5.*m6.*t9.*4.0+Lz5.*Lzcm6.*dQ3.*dQ5.*m6.*t9.*4.0+Lz5.*Lzcm6.*dQ2.*dQ3.*m6.*t39.*2.0+Lz5.*Lzcm6.*dQ4.*dQ5.*m6.*t40.*2.0-Ixx5.*dQ1.*dQ5.*t2.*t4.*t8-Ixx5.*dQ1.*dQ5.*t3.*t4.*t7-Ixx6.*dQ1.*dQ5.*t2.*t4.*t8-Ixx6.*dQ1.*dQ5.*t3.*t4.*t7+Ixx6.*dQ2.*dQ3.*t5.*t6.*t11.*2.0+Ixx4.*dQ1.*dQ2.*t2.*t8.*t34.*2.0+Ixx4.*dQ1.*dQ2.*t3.*t7.*t34.*2.0+Ixx4.*dQ1.*dQ3.*t2.*t8.*t34.*2.0+Ixx4.*dQ1.*dQ3.*t3.*t7.*t34.*2.0-Ixx6.*dQ1.*dQ2.*t2.*t8.*t34.*2.0-Ixx6.*dQ1.*dQ2.*t3.*t7.*t34.*2.0-Ixx6.*dQ1.*dQ3.*t2.*t8.*t34.*2.0-Ixx6.*dQ1.*dQ3.*t3.*t7.*t34.*2.0;
et403 = Ixx6.*dQ1.*dQ2.*t2.*t8.*t36.*-2.0-Ixx6.*dQ1.*dQ2.*t3.*t7.*t36.*2.0-Ixx6.*dQ1.*dQ3.*t2.*t8.*t36.*2.0-Ixx6.*dQ1.*dQ3.*t3.*t7.*t36.*2.0-Ixx5.*dQ2.*dQ3.*t4.*t9.*t35.*2.0-Ixx6.*dQ2.*dQ3.*t4.*t9.*t36.*2.0-Ixx6.*dQ2.*dQ6.*t4.*t10.*t36.*2.0-Ixx6.*dQ3.*dQ6.*t4.*t10.*t36.*2.0+Ixx6.*dQ4.*dQ5.*t5.*t10.*t36.*2.0+Ixx6.*dQ4.*dQ6.*t6.*t11.*t35.*2.0-Ixx6.*dQ2.*dQ5.*t9.*t35.*t36.*2.0-Ixx6.*dQ3.*dQ5.*t9.*t35.*t36.*2.0+Ixy6.*dQ2.*dQ6.*t5.*t9.*t10+Ixy6.*dQ3.*dQ6.*t5.*t9.*t10-Ixy6.*dQ5.*dQ6.*t6.*t10.*t11.*2.0+Ixy6.*dQ1.*dQ6.*t2.*t3.*t35+Ixy6.*dQ1.*dQ6.*t2.*t3.*t36.*2.0+Ixy6.*dQ2.*dQ5.*t4.*t5.*t36.*2.0+Ixy6.*dQ3.*dQ5.*t4.*t5.*t36.*2.0-Ixy6.*dQ1.*dQ6.*t7.*t8.*t35-Ixy6.*dQ1.*dQ6.*t7.*t8.*t36.*2.0+Ixy6.*dQ2.*dQ3.*t5.*t34.*t36.*4.0+Ixz4.*dQ1.*dQ2.*t2.*t3.*t4+Ixz4.*dQ1.*dQ3.*t2.*t3.*t4;
et404 = -Ixz5.*dQ1.*dQ2.*t2.*t3.*t4-Ixz5.*dQ1.*dQ3.*t2.*t3.*t4-Ixz6.*dQ1.*dQ5.*t2.*t3.*t6-Ixz4.*dQ1.*dQ2.*t4.*t7.*t8-Ixz4.*dQ1.*dQ3.*t4.*t7.*t8+Ixz5.*dQ1.*dQ2.*t4.*t7.*t8+Ixz5.*dQ1.*dQ3.*t4.*t7.*t8+Ixz6.*dQ1.*dQ5.*t6.*t7.*t8+Ixz6.*dQ2.*dQ5.*t4.*t10.*t11+Ixz6.*dQ3.*dQ5.*t4.*t10.*t11-Ixz6.*dQ4.*dQ6.*t5.*t10.*t11+Ixz5.*dQ1.*dQ5.*t2.*t3.*t35.*2.0-Ixz5.*dQ1.*dQ5.*t7.*t8.*t35.*2.0+Ixz6.*dQ2.*dQ3.*t10.*t11.*t34.*2.0+Ixz6.*dQ2.*dQ6.*t9.*t11.*t35+Ixz6.*dQ3.*dQ6.*t9.*t11.*t35+Iyx6.*dQ2.*dQ6.*t5.*t9.*t10+Iyx6.*dQ3.*dQ6.*t5.*t9.*t10-Iyx6.*dQ5.*dQ6.*t6.*t10.*t11.*2.0+Iyx6.*dQ1.*dQ6.*t2.*t3.*t35+Iyx6.*dQ1.*dQ6.*t2.*t3.*t36.*2.0+Iyx6.*dQ2.*dQ5.*t4.*t5.*t36.*2.0+Iyx6.*dQ3.*dQ5.*t4.*t5.*t36.*2.0-Iyx6.*dQ1.*dQ6.*t7.*t8.*t35-Iyx6.*dQ1.*dQ6.*t7.*t8.*t36.*2.0;
et405 = Iyx6.*dQ2.*dQ3.*t5.*t34.*t36.*4.0-Iyy5.*dQ1.*dQ5.*t2.*t4.*t8-Iyy5.*dQ1.*dQ5.*t3.*t4.*t7-Iyy6.*dQ1.*dQ5.*t2.*t4.*t8-Iyy6.*dQ1.*dQ5.*t3.*t4.*t7-Iyy6.*dQ2.*dQ3.*t5.*t6.*t11.*2.0-Iyy4.*dQ1.*dQ2.*t2.*t8.*t34.*2.0-Iyy4.*dQ1.*dQ2.*t3.*t7.*t34.*2.0-Iyy4.*dQ1.*dQ3.*t2.*t8.*t34.*2.0-Iyy4.*dQ1.*dQ3.*t3.*t7.*t34.*2.0-Iyy5.*dQ1.*dQ2.*t2.*t8.*t34.*2.0-Iyy5.*dQ1.*dQ2.*t3.*t7.*t34.*2.0-Iyy5.*dQ1.*dQ3.*t2.*t8.*t34.*2.0-Iyy5.*dQ1.*dQ3.*t3.*t7.*t34.*2.0+Iyy6.*dQ1.*dQ2.*t2.*t8.*t36.*2.0+Iyy6.*dQ1.*dQ2.*t3.*t7.*t36.*2.0+Iyy6.*dQ1.*dQ3.*t2.*t8.*t36.*2.0+Iyy6.*dQ1.*dQ3.*t3.*t7.*t36.*2.0-Iyy6.*dQ2.*dQ3.*t4.*t9.*t35.*2.0+Iyy6.*dQ2.*dQ3.*t4.*t9.*t36.*2.0+Iyy6.*dQ2.*dQ6.*t4.*t10.*t36.*2.0+Iyy6.*dQ3.*dQ6.*t4.*t10.*t36.*2.0-Iyy6.*dQ4.*dQ5.*t5.*t10.*t36.*2.0;
et406 = Iyy6.*dQ4.*dQ6.*t6.*t11.*t35.*-2.0+Iyy6.*dQ2.*dQ5.*t9.*t35.*t36.*2.0+Iyy6.*dQ3.*dQ5.*t9.*t35.*t36.*2.0-Iyz4.*dQ1.*dQ2.*t2.*t3.*t9-Iyz4.*dQ1.*dQ3.*t2.*t3.*t9+Iyz6.*dQ1.*dQ5.*t2.*t3.*t11+Iyz4.*dQ1.*dQ2.*t7.*t8.*t9+Iyz4.*dQ1.*dQ3.*t7.*t8.*t9+Iyz6.*dQ2.*dQ5.*t4.*t6.*t10+Iyz6.*dQ3.*dQ5.*t4.*t6.*t10-Iyz6.*dQ4.*dQ6.*t5.*t6.*t10-Iyz6.*dQ1.*dQ5.*t7.*t8.*t11+Iyz6.*dQ2.*dQ3.*t6.*t10.*t34.*2.0+Iyz6.*dQ2.*dQ6.*t6.*t9.*t35+Iyz6.*dQ3.*dQ6.*t6.*t9.*t35+Izx4.*dQ1.*dQ2.*t2.*t3.*t4+Izx4.*dQ1.*dQ3.*t2.*t3.*t4-Izx5.*dQ1.*dQ2.*t2.*t3.*t4-Izx5.*dQ1.*dQ3.*t2.*t3.*t4-Izx6.*dQ1.*dQ5.*t2.*t3.*t6-Izx4.*dQ1.*dQ2.*t4.*t7.*t8-Izx4.*dQ1.*dQ3.*t4.*t7.*t8+Izx5.*dQ1.*dQ2.*t4.*t7.*t8+Izx5.*dQ1.*dQ3.*t4.*t7.*t8+Izx6.*dQ1.*dQ5.*t6.*t7.*t8;
et407 = Izx6.*dQ2.*dQ5.*t4.*t10.*t11+Izx6.*dQ3.*dQ5.*t4.*t10.*t11-Izx6.*dQ4.*dQ6.*t5.*t10.*t11+Izx5.*dQ1.*dQ5.*t2.*t3.*t35.*2.0-Izx5.*dQ1.*dQ5.*t7.*t8.*t35.*2.0+Izx6.*dQ2.*dQ3.*t10.*t11.*t34.*2.0+Izx6.*dQ2.*dQ6.*t9.*t11.*t35+Izx6.*dQ3.*dQ6.*t9.*t11.*t35-Izy4.*dQ1.*dQ2.*t2.*t3.*t9-Izy4.*dQ1.*dQ3.*t2.*t3.*t9+Izy6.*dQ1.*dQ5.*t2.*t3.*t11+Izy4.*dQ1.*dQ2.*t7.*t8.*t9+Izy4.*dQ1.*dQ3.*t7.*t8.*t9+Izy6.*dQ2.*dQ5.*t4.*t6.*t10+Izy6.*dQ3.*dQ5.*t4.*t6.*t10-Izy6.*dQ4.*dQ6.*t5.*t6.*t10-Izy6.*dQ1.*dQ5.*t7.*t8.*t11+Izy6.*dQ2.*dQ3.*t6.*t10.*t34.*2.0+Izy6.*dQ2.*dQ6.*t6.*t9.*t35+Izy6.*dQ3.*dQ6.*t6.*t9.*t35+Izz5.*dQ1.*dQ5.*t2.*t4.*t8+Izz5.*dQ1.*dQ5.*t3.*t4.*t7+Izz6.*dQ1.*dQ5.*t2.*t4.*t8+Izz6.*dQ1.*dQ5.*t3.*t4.*t7+Izz5.*dQ1.*dQ2.*t2.*t8.*t34.*2.0+Izz5.*dQ1.*dQ2.*t3.*t7.*t34.*2.0;
et408 = Izz5.*dQ1.*dQ3.*t2.*t8.*t34.*2.0+Izz5.*dQ1.*dQ3.*t3.*t7.*t34.*2.0+Izz6.*dQ1.*dQ2.*t2.*t8.*t34.*2.0+Izz6.*dQ1.*dQ2.*t3.*t7.*t34.*2.0+Izz6.*dQ1.*dQ3.*t2.*t8.*t34.*2.0+Izz6.*dQ1.*dQ3.*t3.*t7.*t34.*2.0+Izz5.*dQ2.*dQ3.*t4.*t9.*t35.*2.0+Izz6.*dQ2.*dQ3.*t4.*t9.*t35.*2.0-dQ1.*dQ2.*m4.*t2.*t8.*t18.*2.0-dQ1.*dQ2.*m4.*t3.*t7.*t18.*2.0-dQ1.*dQ2.*m6.*t2.*t8.*t17.*2.0-dQ1.*dQ2.*m6.*t3.*t7.*t17.*2.0-dQ1.*dQ3.*m4.*t2.*t8.*t18.*2.0-dQ1.*dQ3.*m4.*t3.*t7.*t18.*2.0-dQ1.*dQ2.*m5.*t2.*t8.*t19.*2.0-dQ1.*dQ2.*m5.*t3.*t7.*t19.*2.0-dQ1.*dQ3.*m6.*t2.*t8.*t17.*2.0-dQ1.*dQ3.*m6.*t3.*t7.*t17.*2.0-dQ1.*dQ3.*m5.*t2.*t8.*t19.*2.0-dQ1.*dQ3.*m5.*t3.*t7.*t19.*2.0-dQ2.*dQ6.*m6.*t4.*t10.*t17.*2.0-dQ3.*dQ6.*m6.*t4.*t10.*t17.*2.0+dQ2.*dQ5.*m5.*t9.*t16.*t35.*2.0;
et409 = dQ3.*dQ5.*m5.*t9.*t16.*t35.*2.0+dQ2.*dQ5.*m6.*t9.*t20.*t35.*2.0+dQ3.*dQ5.*m6.*t9.*t20.*t35.*2.0-dQ2.*dQ5.*m6.*t9.*t22.*t35.*2.0-dQ3.*dQ5.*m6.*t9.*t22.*t35.*2.0+dQ5.*dQ6.*m6.*t10.*t17.*t36.*2.0-dQ2.*dQ5.*m5.*t9.*t25.*t35.*2.0-dQ3.*dQ5.*m5.*t9.*t25.*t35.*2.0-dQ2.*dQ5.*m6.*t9.*t26.*t35.*2.0-dQ5.*dQ6.*m6.*t10.*t20.*t36.*2.0-dQ3.*dQ5.*m6.*t9.*t26.*t35.*2.0-Lx2.*Lxcm4.*dQ1.*dQ2.*m4.*t4.*t7.*2.0+Lx3.*Lxcm5.*dQ2.*dQ3.*m5.*t5.*t9.*2.0+Lx3.*Lxcm6.*dQ2.*dQ3.*m6.*t4.*t11.*2.0+Lx2.*Lycm4.*dQ1.*dQ2.*m4.*t7.*t9.*2.0+Lx3.*Lycm6.*dQ2.*dQ3.*m6.*t4.*t6.*2.0+Lx2.*Lycm5.*dQ1.*dQ2.*m5.*t7.*t9.*2.0-Lxcm6.*Lycm6.*dQ1.*dQ6.*m6.*t2.*t3.*2.0+Lxcm5.*Lycm5.*dQ2.*dQ5.*m5.*t4.*t5.*2.0+Lxcm5.*Lycm5.*dQ3.*dQ5.*m5.*t4.*t5.*2.0-Lxcm6.*Lycm6.*dQ2.*dQ5.*m6.*t4.*t5.*2.0-Lxcm6.*Lycm6.*dQ3.*dQ5.*m6.*t4.*t5.*2.0;
et410 = Lxcm6.*Lycm6.*dQ1.*dQ6.*m6.*t7.*t8.*2.0+Lxcm5.*Lycm5.*dQ2.*dQ3.*m5.*t5.*t34.*4.0-Lxcm6.*Lycm6.*dQ2.*dQ3.*m6.*t5.*t34.*4.0-Lxcm6.*Lycm6.*dQ2.*dQ3.*m6.*t5.*t36.*4.0-Lxcm6.*Lycm6.*dQ4.*dQ6.*m6.*t35.*t36.*4.0+Lx3.*Lz5.*dQ2.*dQ3.*m6.*t9.*t10.*2.0+Lx3.*Lzcm5.*dQ2.*dQ3.*m5.*t9.*t10.*2.0+Lx3.*Lzcm6.*dQ2.*dQ3.*m6.*t9.*t10.*2.0-Lxcm6.*Lz5.*dQ2.*dQ3.*m6.*t10.*t11.*2.0-Lxcm6.*Lz5.*dQ2.*dQ6.*m6.*t9.*t11.*2.0-Lxcm6.*Lz5.*dQ3.*dQ6.*m6.*t9.*t11.*2.0+Lxcm6.*Lz5.*dQ4.*dQ5.*m6.*t6.*t35.*4.0-Lxcm5.*Lzcm5.*dQ1.*dQ5.*m5.*t2.*t3.*2.0+Lxcm5.*Lzcm5.*dQ1.*dQ5.*m5.*t7.*t8.*2.0-Lxcm6.*Lzcm6.*dQ2.*dQ3.*m6.*t10.*t11.*2.0-Lxcm6.*Lzcm6.*dQ2.*dQ6.*m6.*t9.*t11.*2.0-Lxcm6.*Lzcm6.*dQ3.*dQ6.*m6.*t9.*t11.*2.0+Lxcm6.*Lzcm6.*dQ4.*dQ5.*m6.*t6.*t35.*4.0-Lycm6.*Lz5.*dQ2.*dQ3.*m6.*t6.*t10.*2.0-Lycm6.*Lz5.*dQ2.*dQ6.*m6.*t6.*t9.*2.0;
et411 = Lycm6.*Lz5.*dQ3.*dQ6.*m6.*t6.*t9.*-2.0-Lycm6.*Lz5.*dQ4.*dQ5.*m6.*t11.*t35.*4.0+Lycm5.*Lzcm5.*dQ2.*dQ5.*m5.*t4.*t10.*2.0+Lycm5.*Lzcm5.*dQ3.*dQ5.*m5.*t4.*t10.*2.0-Lycm6.*Lzcm6.*dQ2.*dQ3.*m6.*t6.*t10.*2.0-Lycm6.*Lzcm6.*dQ2.*dQ6.*m6.*t6.*t9.*2.0-Lycm6.*Lzcm6.*dQ3.*dQ6.*m6.*t6.*t9.*2.0+Lycm5.*Lzcm5.*dQ2.*dQ3.*m5.*t10.*t34.*4.0-Lycm6.*Lzcm6.*dQ4.*dQ5.*m6.*t11.*t35.*4.0-Lz5.*Lzcm6.*dQ2.*dQ5.*m6.*t9.*t35.*4.0-Lz5.*Lzcm6.*dQ3.*dQ5.*m6.*t9.*t35.*4.0+Ixx5.*dQ1.*dQ5.*t2.*t3.*t5.*t10.*2.0-Ixx6.*dQ1.*dQ6.*t2.*t3.*t6.*t11.*2.0-Ixx6.*dQ2.*dQ5.*t4.*t5.*t6.*t11.*2.0-Ixx6.*dQ3.*dQ5.*t4.*t5.*t6.*t11.*2.0-Ixx5.*dQ1.*dQ5.*t5.*t7.*t8.*t10.*2.0+Ixx6.*dQ1.*dQ6.*t2.*t8.*t9.*t10+Ixx6.*dQ1.*dQ6.*t3.*t7.*t9.*t10+Ixx6.*dQ1.*dQ6.*t6.*t7.*t8.*t11.*2.0+Ixx5.*dQ1.*dQ5.*t2.*t4.*t8.*t35.*2.0+Ixx5.*dQ1.*dQ5.*t3.*t4.*t7.*t35.*2.0;
et412 = Ixx6.*dQ2.*dQ3.*t5.*t6.*t11.*t34.*-4.0+Ixx5.*dQ1.*dQ2.*t2.*t8.*t34.*t35.*2.0+Ixx5.*dQ1.*dQ2.*t3.*t7.*t34.*t35.*2.0+Ixx5.*dQ1.*dQ3.*t2.*t8.*t34.*t35.*2.0+Ixx5.*dQ1.*dQ3.*t3.*t7.*t34.*t35.*2.0+Ixx6.*dQ1.*dQ2.*t2.*t8.*t34.*t36.*2.0+Ixx6.*dQ1.*dQ2.*t3.*t7.*t34.*t36.*2.0+Ixx6.*dQ1.*dQ3.*t2.*t8.*t34.*t36.*2.0+Ixx6.*dQ1.*dQ3.*t3.*t7.*t34.*t36.*2.0-Ixx6.*dQ2.*dQ3.*t4.*t9.*t35.*t36.*2.0+Ixy4.*dQ1.*dQ2.*t2.*t4.*t8.*t9.*2.0+Ixy4.*dQ1.*dQ2.*t3.*t4.*t7.*t9.*2.0+Ixy4.*dQ1.*dQ3.*t2.*t4.*t8.*t9.*2.0+Ixy4.*dQ1.*dQ3.*t3.*t4.*t7.*t9.*2.0+Ixy5.*dQ1.*dQ2.*t2.*t3.*t9.*t10+Ixy5.*dQ1.*dQ3.*t2.*t3.*t9.*t10-Ixy6.*dQ1.*dQ2.*t2.*t3.*t9.*t10-Ixy6.*dQ1.*dQ3.*t2.*t3.*t9.*t10+Ixy5.*dQ1.*dQ5.*t2.*t5.*t8.*t9+Ixy5.*dQ1.*dQ5.*t3.*t5.*t7.*t9-Ixy6.*dQ1.*dQ2.*t2.*t6.*t8.*t11.*2.0-Ixy6.*dQ1.*dQ2.*t3.*t6.*t7.*t11.*2.0;
et413 = -Ixy6.*dQ1.*dQ5.*t2.*t5.*t8.*t9-Ixy6.*dQ1.*dQ5.*t3.*t5.*t7.*t9-Ixy6.*dQ1.*dQ3.*t2.*t6.*t8.*t11.*2.0-Ixy6.*dQ1.*dQ3.*t3.*t6.*t7.*t11.*2.0-Ixy6.*dQ2.*dQ3.*t4.*t6.*t9.*t11.*2.0-Ixy5.*dQ1.*dQ2.*t7.*t8.*t9.*t10-Ixy5.*dQ1.*dQ3.*t7.*t8.*t9.*t10+Ixy6.*dQ1.*dQ2.*t7.*t8.*t9.*t10+Ixy6.*dQ1.*dQ3.*t7.*t8.*t9.*t10-Ixy6.*dQ2.*dQ6.*t4.*t6.*t10.*t11.*2.0-Ixy6.*dQ3.*dQ6.*t4.*t6.*t10.*t11.*2.0+Ixy6.*dQ4.*dQ5.*t5.*t6.*t10.*t11.*2.0-Ixy6.*dQ2.*dQ5.*t6.*t9.*t11.*t35.*2.0-Ixy6.*dQ2.*dQ6.*t5.*t9.*t10.*t36.*2.0-Ixy6.*dQ3.*dQ5.*t6.*t9.*t11.*t35.*2.0-Ixy6.*dQ3.*dQ6.*t5.*t9.*t10.*t36.*2.0-Ixy6.*dQ1.*dQ6.*t2.*t3.*t35.*t36.*2.0+Ixy6.*dQ1.*dQ6.*t7.*t8.*t35.*t36.*2.0-Ixz6.*dQ1.*dQ2.*t2.*t3.*t4.*t6-Ixz6.*dQ1.*dQ3.*t2.*t3.*t4.*t6;
et414 = Ixz6.*dQ1.*dQ2.*t4.*t6.*t7.*t8+Ixz6.*dQ1.*dQ3.*t4.*t6.*t7.*t8+Ixz5.*dQ2.*dQ3.*t4.*t5.*t9.*t10.*2.0+Ixz6.*dQ1.*dQ6.*t2.*t4.*t8.*t11+Ixz6.*dQ1.*dQ6.*t3.*t4.*t7.*t11+Ixz5.*dQ1.*dQ2.*t2.*t3.*t4.*t35.*2.0+Ixz5.*dQ1.*dQ3.*t2.*t3.*t4.*t35.*2.0+Ixz6.*dQ1.*dQ5.*t2.*t3.*t6.*t35.*2.0-Ixz5.*dQ1.*dQ2.*t4.*t7.*t8.*t35.*2.0-Ixz5.*dQ1.*dQ3.*t4.*t7.*t8.*t35.*2.0-Ixz6.*dQ1.*dQ5.*t6.*t7.*t8.*t35.*2.0+Iyx4.*dQ1.*dQ2.*t2.*t4.*t8.*t9.*2.0+Iyx4.*dQ1.*dQ2.*t3.*t4.*t7.*t9.*2.0+Iyx4.*dQ1.*dQ3.*t2.*t4.*t8.*t9.*2.0+Iyx4.*dQ1.*dQ3.*t3.*t4.*t7.*t9.*2.0+Iyx5.*dQ1.*dQ2.*t2.*t3.*t9.*t10+Iyx5.*dQ1.*dQ3.*t2.*t3.*t9.*t10-Iyx6.*dQ1.*dQ2.*t2.*t3.*t9.*t10-Iyx6.*dQ1.*dQ3.*t2.*t3.*t9.*t10+Iyx5.*dQ1.*dQ5.*t2.*t5.*t8.*t9+Iyx5.*dQ1.*dQ5.*t3.*t5.*t7.*t9-Iyx6.*dQ1.*dQ2.*t2.*t6.*t8.*t11.*2.0;
et415 = Iyx6.*dQ1.*dQ2.*t3.*t6.*t7.*t11.*-2.0-Iyx6.*dQ1.*dQ5.*t2.*t5.*t8.*t9-Iyx6.*dQ1.*dQ5.*t3.*t5.*t7.*t9-Iyx6.*dQ1.*dQ3.*t2.*t6.*t8.*t11.*2.0-Iyx6.*dQ1.*dQ3.*t3.*t6.*t7.*t11.*2.0-Iyx6.*dQ2.*dQ3.*t4.*t6.*t9.*t11.*2.0-Iyx5.*dQ1.*dQ2.*t7.*t8.*t9.*t10-Iyx5.*dQ1.*dQ3.*t7.*t8.*t9.*t10+Iyx6.*dQ1.*dQ2.*t7.*t8.*t9.*t10+Iyx6.*dQ1.*dQ3.*t7.*t8.*t9.*t10-Iyx6.*dQ2.*dQ6.*t4.*t6.*t10.*t11.*2.0-Iyx6.*dQ3.*dQ6.*t4.*t6.*t10.*t11.*2.0+Iyx6.*dQ4.*dQ5.*t5.*t6.*t10.*t11.*2.0-Iyx6.*dQ2.*dQ5.*t6.*t9.*t11.*t35.*2.0-Iyx6.*dQ2.*dQ6.*t5.*t9.*t10.*t36.*2.0-Iyx6.*dQ3.*dQ5.*t6.*t9.*t11.*t35.*2.0-Iyx6.*dQ3.*dQ6.*t5.*t9.*t10.*t36.*2.0-Iyx6.*dQ1.*dQ6.*t2.*t3.*t35.*t36.*2.0+Iyx6.*dQ1.*dQ6.*t7.*t8.*t35.*t36.*2.0+Iyy6.*dQ1.*dQ5.*t2.*t3.*t5.*t10.*2.0;
et416 = Iyy6.*dQ1.*dQ6.*t2.*t3.*t6.*t11.*2.0+Iyy6.*dQ2.*dQ5.*t4.*t5.*t6.*t11.*2.0+Iyy6.*dQ3.*dQ5.*t4.*t5.*t6.*t11.*2.0-Iyy6.*dQ1.*dQ5.*t5.*t7.*t8.*t10.*2.0-Iyy6.*dQ1.*dQ6.*t2.*t8.*t9.*t10-Iyy6.*dQ1.*dQ6.*t3.*t7.*t9.*t10-Iyy6.*dQ1.*dQ6.*t6.*t7.*t8.*t11.*2.0+Iyy6.*dQ1.*dQ5.*t2.*t4.*t8.*t35.*2.0+Iyy6.*dQ1.*dQ5.*t3.*t4.*t7.*t35.*2.0+Iyy6.*dQ2.*dQ3.*t5.*t6.*t11.*t34.*4.0+Iyy6.*dQ1.*dQ2.*t2.*t8.*t34.*t35.*2.0+Iyy6.*dQ1.*dQ2.*t3.*t7.*t34.*t35.*2.0-Iyy6.*dQ1.*dQ2.*t2.*t8.*t34.*t36.*2.0-Iyy6.*dQ1.*dQ2.*t3.*t7.*t34.*t36.*2.0+Iyy6.*dQ1.*dQ3.*t2.*t8.*t34.*t35.*2.0+Iyy6.*dQ1.*dQ3.*t3.*t7.*t34.*t35.*2.0-Iyy6.*dQ1.*dQ3.*t2.*t8.*t34.*t36.*2.0-Iyy6.*dQ1.*dQ3.*t3.*t7.*t34.*t36.*2.0+Iyy6.*dQ2.*dQ3.*t4.*t9.*t35.*t36.*2.0-Iyz5.*dQ1.*dQ2.*t2.*t3.*t5.*t9-Iyz5.*dQ1.*dQ3.*t2.*t3.*t5.*t9;
et417 = Iyz6.*dQ1.*dQ2.*t2.*t3.*t4.*t11+Iyz6.*dQ1.*dQ3.*t2.*t3.*t4.*t11+Iyz6.*dQ1.*dQ6.*t2.*t4.*t6.*t8+Iyz6.*dQ1.*dQ6.*t3.*t4.*t6.*t7+Iyz5.*dQ1.*dQ2.*t5.*t7.*t8.*t9+Iyz5.*dQ1.*dQ3.*t5.*t7.*t8.*t9-Iyz6.*dQ1.*dQ2.*t4.*t7.*t8.*t11+Iyz5.*dQ1.*dQ5.*t2.*t8.*t9.*t10+Iyz5.*dQ1.*dQ5.*t3.*t7.*t9.*t10-Iyz6.*dQ1.*dQ3.*t4.*t7.*t8.*t11-Iyz6.*dQ1.*dQ5.*t2.*t3.*t11.*t35.*2.0+Iyz6.*dQ1.*dQ5.*t7.*t8.*t11.*t35.*2.0-Izx6.*dQ1.*dQ2.*t2.*t3.*t4.*t6-Izx6.*dQ1.*dQ3.*t2.*t3.*t4.*t6+Izx6.*dQ1.*dQ2.*t4.*t6.*t7.*t8+Izx6.*dQ1.*dQ3.*t4.*t6.*t7.*t8+Izx5.*dQ2.*dQ3.*t4.*t5.*t9.*t10.*2.0+Izx6.*dQ1.*dQ6.*t2.*t4.*t8.*t11+Izx6.*dQ1.*dQ6.*t3.*t4.*t7.*t11+Izx5.*dQ1.*dQ2.*t2.*t3.*t4.*t35.*2.0+Izx5.*dQ1.*dQ3.*t2.*t3.*t4.*t35.*2.0+Izx6.*dQ1.*dQ5.*t2.*t3.*t6.*t35.*2.0;
et418 = Izx5.*dQ1.*dQ2.*t4.*t7.*t8.*t35.*-2.0-Izx5.*dQ1.*dQ3.*t4.*t7.*t8.*t35.*2.0-Izx6.*dQ1.*dQ5.*t6.*t7.*t8.*t35.*2.0-Izy5.*dQ1.*dQ2.*t2.*t3.*t5.*t9-Izy5.*dQ1.*dQ3.*t2.*t3.*t5.*t9+Izy6.*dQ1.*dQ2.*t2.*t3.*t4.*t11+Izy6.*dQ1.*dQ3.*t2.*t3.*t4.*t11+Izy6.*dQ1.*dQ6.*t2.*t4.*t6.*t8+Izy6.*dQ1.*dQ6.*t3.*t4.*t6.*t7+Izy5.*dQ1.*dQ2.*t5.*t7.*t8.*t9+Izy5.*dQ1.*dQ3.*t5.*t7.*t8.*t9-Izy6.*dQ1.*dQ2.*t4.*t7.*t8.*t11+Izy5.*dQ1.*dQ5.*t2.*t8.*t9.*t10+Izy5.*dQ1.*dQ5.*t3.*t7.*t9.*t10-Izy6.*dQ1.*dQ3.*t4.*t7.*t8.*t11-Izy6.*dQ1.*dQ5.*t2.*t3.*t11.*t35.*2.0+Izy6.*dQ1.*dQ5.*t7.*t8.*t11.*t35.*2.0-Izz5.*dQ1.*dQ5.*t2.*t3.*t5.*t10.*2.0-Izz6.*dQ1.*dQ5.*t2.*t3.*t5.*t10.*2.0+Izz5.*dQ1.*dQ5.*t5.*t7.*t8.*t10.*2.0+Izz6.*dQ1.*dQ5.*t5.*t7.*t8.*t10.*2.0;
et419 = -Izz6.*dQ1.*dQ6.*t2.*t8.*t9.*t10-Izz6.*dQ1.*dQ6.*t3.*t7.*t9.*t10-Izz5.*dQ1.*dQ5.*t2.*t4.*t8.*t35.*2.0-Izz5.*dQ1.*dQ5.*t3.*t4.*t7.*t35.*2.0-Izz6.*dQ1.*dQ5.*t2.*t4.*t8.*t35.*2.0-Izz6.*dQ1.*dQ5.*t3.*t4.*t7.*t35.*2.0-Izz5.*dQ1.*dQ2.*t2.*t8.*t34.*t35.*2.0-Izz5.*dQ1.*dQ2.*t3.*t7.*t34.*t35.*2.0-Izz5.*dQ1.*dQ3.*t2.*t8.*t34.*t35.*2.0-Izz5.*dQ1.*dQ3.*t3.*t7.*t34.*t35.*2.0-Izz6.*dQ1.*dQ2.*t2.*t8.*t34.*t35.*2.0-Izz6.*dQ1.*dQ2.*t3.*t7.*t34.*t35.*2.0-Izz6.*dQ1.*dQ3.*t2.*t8.*t34.*t35.*2.0-Izz6.*dQ1.*dQ3.*t3.*t7.*t34.*t35.*2.0-dQ1.*dQ5.*m6.*t2.*t4.*t8.*t22.*2.0-dQ1.*dQ5.*m6.*t3.*t4.*t7.*t22.*2.0-dQ1.*dQ5.*m5.*t2.*t4.*t8.*t25.*2.0-dQ1.*dQ5.*m5.*t3.*t4.*t7.*t25.*2.0-dQ2.*dQ3.*m6.*t5.*t6.*t11.*t17.*2.0-dQ1.*dQ5.*m6.*t2.*t4.*t8.*t26.*2.0;
et420 = dQ1.*dQ5.*m6.*t3.*t4.*t7.*t26.*-2.0+dQ2.*dQ3.*m6.*t5.*t6.*t11.*t20.*2.0-dQ1.*dQ2.*m4.*t2.*t8.*t15.*t34.*2.0-dQ1.*dQ2.*m4.*t3.*t7.*t15.*t34.*2.0-dQ1.*dQ3.*m4.*t2.*t8.*t15.*t34.*2.0-dQ1.*dQ3.*m4.*t3.*t7.*t15.*t34.*2.0+dQ1.*dQ2.*m4.*t2.*t8.*t18.*t34.*2.0+dQ1.*dQ2.*m4.*t3.*t7.*t18.*t34.*2.0+dQ1.*dQ2.*m6.*t2.*t8.*t17.*t34.*2.0+dQ1.*dQ2.*m6.*t3.*t7.*t17.*t34.*2.0+dQ1.*dQ3.*m4.*t2.*t8.*t18.*t34.*2.0+dQ1.*dQ3.*m4.*t3.*t7.*t18.*t34.*2.0+dQ1.*dQ2.*m5.*t2.*t8.*t19.*t34.*2.0+dQ1.*dQ2.*m5.*t3.*t7.*t19.*t34.*2.0+dQ1.*dQ3.*m6.*t2.*t8.*t17.*t34.*2.0+dQ1.*dQ3.*m6.*t3.*t7.*t17.*t34.*2.0+dQ1.*dQ2.*m6.*t2.*t8.*t17.*t36.*2.0+dQ1.*dQ2.*m6.*t3.*t7.*t17.*t36.*2.0+dQ1.*dQ3.*m5.*t2.*t8.*t19.*t34.*2.0+dQ1.*dQ3.*m5.*t3.*t7.*t19.*t34.*2.0+dQ1.*dQ3.*m6.*t2.*t8.*t17.*t36.*2.0;
et421 = dQ1.*dQ3.*m6.*t3.*t7.*t17.*t36.*2.0+dQ2.*dQ3.*m5.*t4.*t9.*t16.*t35.*2.0-dQ1.*dQ2.*m6.*t2.*t8.*t20.*t36.*2.0-dQ1.*dQ2.*m6.*t2.*t8.*t22.*t34.*2.0-dQ1.*dQ2.*m6.*t3.*t7.*t20.*t36.*2.0-dQ1.*dQ2.*m6.*t3.*t7.*t22.*t34.*2.0-dQ1.*dQ3.*m6.*t2.*t8.*t20.*t36.*2.0-dQ1.*dQ3.*m6.*t2.*t8.*t22.*t34.*2.0-dQ1.*dQ3.*m6.*t3.*t7.*t20.*t36.*2.0-dQ1.*dQ3.*m6.*t3.*t7.*t22.*t34.*2.0-dQ1.*dQ2.*m5.*t2.*t8.*t25.*t34.*2.0-dQ1.*dQ2.*m5.*t3.*t7.*t25.*t34.*2.0+dQ2.*dQ3.*m6.*t4.*t9.*t17.*t36.*2.0-dQ1.*dQ3.*m5.*t2.*t8.*t25.*t34.*2.0-dQ1.*dQ3.*m5.*t3.*t7.*t25.*t34.*2.0-dQ1.*dQ2.*m6.*t2.*t8.*t26.*t34.*2.0-dQ1.*dQ2.*m6.*t3.*t7.*t26.*t34.*2.0+dQ2.*dQ3.*m6.*t4.*t9.*t20.*t35.*2.0-dQ1.*dQ3.*m6.*t2.*t8.*t26.*t34.*2.0-dQ1.*dQ3.*m6.*t3.*t7.*t26.*t34.*2.0;
et422 = dQ2.*dQ3.*m6.*t4.*t9.*t20.*t36.*-2.0-dQ2.*dQ3.*m6.*t4.*t9.*t22.*t35.*2.0+dQ2.*dQ6.*m6.*t4.*t10.*t17.*t36.*2.0+dQ3.*dQ6.*m6.*t4.*t10.*t17.*t36.*2.0-dQ2.*dQ3.*m5.*t4.*t9.*t25.*t35.*2.0-dQ4.*dQ5.*m6.*t5.*t10.*t17.*t36.*2.0-dQ2.*dQ6.*m6.*t4.*t10.*t20.*t36.*2.0-dQ2.*dQ3.*m6.*t4.*t9.*t26.*t35.*2.0-dQ3.*dQ6.*m6.*t4.*t10.*t20.*t36.*2.0-dQ4.*dQ6.*m6.*t6.*t11.*t17.*t35.*2.0+dQ4.*dQ5.*m6.*t5.*t10.*t20.*t36.*2.0+dQ4.*dQ6.*m6.*t6.*t11.*t20.*t35.*2.0+dQ2.*dQ5.*m6.*t9.*t17.*t35.*t36.*2.0+dQ3.*dQ5.*m6.*t9.*t17.*t35.*t36.*2.0-dQ2.*dQ5.*m6.*t9.*t20.*t35.*t36.*2.0-dQ3.*dQ5.*m6.*t9.*t20.*t35.*t36.*2.0-Lx3.*Lxcm4.*dQ1.*dQ2.*m4.*t2.*t4.*t8.*2.0-Lx3.*Lxcm4.*dQ1.*dQ2.*m4.*t3.*t4.*t7.*2.0-Lx3.*Lxcm4.*dQ1.*dQ3.*m4.*t2.*t4.*t8.*2.0-Lx3.*Lxcm4.*dQ1.*dQ3.*m4.*t3.*t4.*t7.*2.0;
et423 = Lx2.*Lxcm5.*dQ1.*dQ2.*m5.*t4.*t5.*t7.*-2.0+Lx3.*Lxcm6.*dQ2.*dQ3.*m6.*t5.*t6.*t9.*2.0+Lx2.*Lxcm6.*dQ1.*dQ2.*m6.*t7.*t9.*t11.*2.0+Lx3.*Lycm4.*dQ1.*dQ2.*m4.*t2.*t8.*t9.*2.0+Lx3.*Lycm4.*dQ1.*dQ2.*m4.*t3.*t7.*t9.*2.0+Lx3.*Lycm4.*dQ1.*dQ3.*m4.*t2.*t8.*t9.*2.0+Lx3.*Lycm4.*dQ1.*dQ3.*m4.*t3.*t7.*t9.*2.0+Lx3.*Lycm5.*dQ1.*dQ2.*m5.*t2.*t8.*t9.*2.0+Lx3.*Lycm5.*dQ1.*dQ2.*m5.*t3.*t7.*t9.*2.0+Lx3.*Lycm5.*dQ1.*dQ3.*m5.*t2.*t8.*t9.*2.0+Lx3.*Lycm5.*dQ1.*dQ3.*m5.*t3.*t7.*t9.*2.0+Lx2.*Lycm6.*dQ1.*dQ2.*m6.*t6.*t7.*t9.*2.0-Lx3.*Lycm6.*dQ2.*dQ3.*m6.*t5.*t9.*t11.*2.0+Lxcm6.*Lycm6.*dQ2.*dQ6.*m6.*t5.*t9.*t10.*2.0+Lxcm6.*Lycm6.*dQ3.*dQ6.*m6.*t5.*t9.*t10.*2.0-Lxcm6.*Lycm6.*dQ5.*dQ6.*m6.*t6.*t10.*t11.*4.0+Lxcm6.*Lycm6.*dQ1.*dQ6.*m6.*t2.*t3.*t35.*2.0+Lxcm6.*Lycm6.*dQ1.*dQ6.*m6.*t2.*t3.*t36.*4.0+Lxcm6.*Lycm6.*dQ2.*dQ5.*m6.*t4.*t5.*t36.*4.0;
et424 = Lxcm6.*Lycm6.*dQ3.*dQ5.*m6.*t4.*t5.*t36.*4.0-Lxcm6.*Lycm6.*dQ1.*dQ6.*m6.*t7.*t8.*t35.*2.0-Lxcm6.*Lycm6.*dQ1.*dQ6.*m6.*t7.*t8.*t36.*4.0+Lxcm6.*Lycm6.*dQ2.*dQ3.*m6.*t5.*t34.*t36.*8.0-Lx2.*Lz5.*dQ1.*dQ2.*m6.*t4.*t7.*t10.*2.0-Lxcm6.*Lz5.*dQ1.*dQ5.*m6.*t2.*t3.*t6.*2.0-Lx2.*Lzcm5.*dQ1.*dQ2.*m5.*t4.*t7.*t10.*2.0-Lx2.*Lzcm6.*dQ1.*dQ2.*m6.*t4.*t7.*t10.*2.0+Lxcm6.*Lz5.*dQ1.*dQ5.*m6.*t6.*t7.*t8.*2.0+Lxcm6.*Lz5.*dQ2.*dQ5.*m6.*t4.*t10.*t11.*2.0+Lxcm6.*Lz5.*dQ3.*dQ5.*m6.*t4.*t10.*t11.*2.0-Lxcm6.*Lz5.*dQ4.*dQ6.*m6.*t5.*t10.*t11.*2.0+Lxcm6.*Lz5.*dQ2.*dQ3.*m6.*t10.*t11.*t34.*4.0+Lxcm6.*Lz5.*dQ2.*dQ6.*m6.*t9.*t11.*t35.*2.0+Lxcm6.*Lz5.*dQ3.*dQ6.*m6.*t9.*t11.*t35.*2.0+Lxcm4.*Lzcm4.*dQ1.*dQ2.*m4.*t2.*t3.*t4.*2.0+Lxcm4.*Lzcm4.*dQ1.*dQ3.*m4.*t2.*t3.*t4.*2.0-Lxcm5.*Lzcm5.*dQ1.*dQ2.*m5.*t2.*t3.*t4.*2.0-Lxcm5.*Lzcm5.*dQ1.*dQ3.*m5.*t2.*t3.*t4.*2.0;
et425 = Lxcm4.*Lzcm4.*dQ1.*dQ2.*m4.*t4.*t7.*t8.*-2.0-Lxcm4.*Lzcm4.*dQ1.*dQ3.*m4.*t4.*t7.*t8.*2.0-Lxcm6.*Lzcm6.*dQ1.*dQ5.*m6.*t2.*t3.*t6.*2.0+Lxcm5.*Lzcm5.*dQ1.*dQ2.*m5.*t4.*t7.*t8.*2.0+Lxcm5.*Lzcm5.*dQ1.*dQ3.*m5.*t4.*t7.*t8.*2.0+Lxcm6.*Lzcm6.*dQ1.*dQ5.*m6.*t6.*t7.*t8.*2.0+Lxcm5.*Lzcm5.*dQ2.*dQ5.*m5.*t5.*t9.*t10.*4.0+Lxcm5.*Lzcm5.*dQ3.*dQ5.*m5.*t5.*t9.*t10.*4.0+Lxcm6.*Lzcm6.*dQ2.*dQ5.*m6.*t4.*t10.*t11.*2.0+Lxcm6.*Lzcm6.*dQ3.*dQ5.*m6.*t4.*t10.*t11.*2.0-Lxcm6.*Lzcm6.*dQ4.*dQ6.*m6.*t5.*t10.*t11.*2.0+Lxcm5.*Lzcm5.*dQ1.*dQ5.*m5.*t2.*t3.*t35.*4.0-Lxcm5.*Lzcm5.*dQ1.*dQ5.*m5.*t7.*t8.*t35.*4.0+Lxcm6.*Lzcm6.*dQ2.*dQ3.*m6.*t10.*t11.*t34.*4.0+Lxcm6.*Lzcm6.*dQ2.*dQ6.*m6.*t9.*t11.*t35.*2.0+Lxcm6.*Lzcm6.*dQ3.*dQ6.*m6.*t9.*t11.*t35.*2.0-Lycm5.*Lz4.*dQ1.*dQ2.*m5.*t2.*t3.*t9.*2.0-Lycm5.*Lz4.*dQ1.*dQ3.*m5.*t2.*t3.*t9.*2.0+Lycm6.*Lz5.*dQ1.*dQ5.*m6.*t2.*t3.*t11.*2.0;
et426 = Lycm5.*Lz4.*dQ1.*dQ2.*m5.*t7.*t8.*t9.*2.0+Lycm5.*Lz4.*dQ1.*dQ3.*m5.*t7.*t8.*t9.*2.0+Lycm6.*Lz5.*dQ2.*dQ5.*m6.*t4.*t6.*t10.*2.0+Lycm6.*Lz5.*dQ3.*dQ5.*m6.*t4.*t6.*t10.*2.0-Lycm6.*Lz5.*dQ4.*dQ6.*m6.*t5.*t6.*t10.*2.0-Lycm6.*Lz5.*dQ1.*dQ5.*m6.*t7.*t8.*t11.*2.0+Lycm6.*Lz5.*dQ2.*dQ3.*m6.*t6.*t10.*t34.*4.0+Lycm6.*Lz5.*dQ2.*dQ6.*m6.*t6.*t9.*t35.*2.0+Lycm6.*Lz5.*dQ3.*dQ6.*m6.*t6.*t9.*t35.*2.0-Lycm4.*Lzcm4.*dQ1.*dQ2.*m4.*t2.*t3.*t9.*2.0-Lycm4.*Lzcm4.*dQ1.*dQ3.*m4.*t2.*t3.*t9.*2.0+Lycm4.*Lzcm4.*dQ1.*dQ2.*m4.*t7.*t8.*t9.*2.0+Lycm4.*Lzcm4.*dQ1.*dQ3.*m4.*t7.*t8.*t9.*2.0+Lycm6.*Lzcm6.*dQ1.*dQ5.*m6.*t2.*t3.*t11.*2.0+Lycm6.*Lzcm6.*dQ2.*dQ5.*m6.*t4.*t6.*t10.*2.0+Lycm6.*Lzcm6.*dQ3.*dQ5.*m6.*t4.*t6.*t10.*2.0-Lycm6.*Lzcm6.*dQ4.*dQ6.*m6.*t5.*t6.*t10.*2.0-Lycm6.*Lzcm6.*dQ1.*dQ5.*m6.*t7.*t8.*t11.*2.0+Lycm6.*Lzcm6.*dQ2.*dQ3.*m6.*t6.*t10.*t34.*4.0;
et427 = Lycm6.*Lzcm6.*dQ2.*dQ6.*m6.*t6.*t9.*t35.*2.0+Lycm6.*Lzcm6.*dQ3.*dQ6.*m6.*t6.*t9.*t35.*2.0-Lz5.*Lzcm6.*dQ1.*dQ5.*m6.*t2.*t4.*t8.*4.0-Lz5.*Lzcm6.*dQ1.*dQ5.*m6.*t3.*t4.*t7.*4.0-Lz5.*Lzcm6.*dQ1.*dQ2.*m6.*t2.*t8.*t34.*4.0-Lz5.*Lzcm6.*dQ1.*dQ2.*m6.*t3.*t7.*t34.*4.0-Lz5.*Lzcm6.*dQ1.*dQ3.*m6.*t2.*t8.*t34.*4.0-Lz5.*Lzcm6.*dQ1.*dQ3.*m6.*t3.*t7.*t34.*4.0-Lz5.*Lzcm6.*dQ2.*dQ3.*m6.*t4.*t9.*t35.*4.0+Ixx5.*dQ1.*dQ2.*t2.*t3.*t4.*t5.*t10.*2.0+Ixx5.*dQ1.*dQ3.*t2.*t3.*t4.*t5.*t10.*2.0-Ixx5.*dQ1.*dQ2.*t4.*t5.*t7.*t8.*t10.*2.0-Ixx5.*dQ1.*dQ3.*t4.*t5.*t7.*t8.*t10.*2.0+Ixx6.*dQ2.*dQ6.*t5.*t6.*t9.*t10.*t11.*2.0+Ixx6.*dQ3.*dQ6.*t5.*t6.*t9.*t10.*t11.*2.0+Ixx6.*dQ1.*dQ5.*t2.*t3.*t5.*t10.*t36.*2.0+Ixx6.*dQ1.*dQ6.*t2.*t3.*t6.*t11.*t35.*2.0-Ixx6.*dQ1.*dQ5.*t5.*t7.*t8.*t10.*t36.*2.0;
et428 = Ixx6.*dQ1.*dQ6.*t2.*t8.*t9.*t10.*t36.*-2.0-Ixx6.*dQ1.*dQ6.*t3.*t7.*t9.*t10.*t36.*2.0-Ixx6.*dQ1.*dQ6.*t6.*t7.*t8.*t11.*t35.*2.0+Ixx6.*dQ1.*dQ5.*t2.*t4.*t8.*t35.*t36.*2.0+Ixx6.*dQ1.*dQ5.*t3.*t4.*t7.*t35.*t36.*2.0+Ixx6.*dQ1.*dQ2.*t2.*t8.*t34.*t35.*t36.*2.0+Ixx6.*dQ1.*dQ2.*t3.*t7.*t34.*t35.*t36.*2.0+Ixx6.*dQ1.*dQ3.*t2.*t8.*t34.*t35.*t36.*2.0+Ixx6.*dQ1.*dQ3.*t3.*t7.*t34.*t35.*t36.*2.0+Ixy5.*dQ1.*dQ2.*t2.*t4.*t5.*t8.*t9.*2.0+Ixy5.*dQ1.*dQ2.*t3.*t4.*t5.*t7.*t9.*2.0+Ixy5.*dQ1.*dQ3.*t2.*t4.*t5.*t8.*t9.*2.0+Ixy5.*dQ1.*dQ3.*t3.*t4.*t5.*t7.*t9.*2.0-Ixy6.*dQ1.*dQ2.*t2.*t4.*t5.*t8.*t9.*2.0-Ixy6.*dQ1.*dQ2.*t3.*t4.*t5.*t7.*t9.*2.0-Ixy6.*dQ1.*dQ3.*t2.*t4.*t5.*t8.*t9.*2.0-Ixy6.*dQ1.*dQ3.*t3.*t4.*t5.*t7.*t9.*2.0-Ixy6.*dQ1.*dQ6.*t2.*t4.*t5.*t8.*t10-Ixy6.*dQ1.*dQ6.*t3.*t4.*t5.*t7.*t10;
et429 = Ixy6.*dQ1.*dQ2.*t2.*t3.*t9.*t10.*t36.*2.0+Ixy6.*dQ1.*dQ2.*t2.*t6.*t8.*t11.*t34.*2.0+Ixy6.*dQ1.*dQ2.*t3.*t6.*t7.*t11.*t34.*2.0+Ixy6.*dQ1.*dQ3.*t2.*t3.*t9.*t10.*t36.*2.0+Ixy6.*dQ1.*dQ3.*t2.*t6.*t8.*t11.*t34.*2.0+Ixy6.*dQ1.*dQ3.*t3.*t6.*t7.*t11.*t34.*2.0+Ixy6.*dQ1.*dQ5.*t2.*t5.*t8.*t9.*t36.*2.0+Ixy6.*dQ1.*dQ5.*t3.*t5.*t7.*t9.*t36.*2.0-Ixy6.*dQ2.*dQ3.*t4.*t6.*t9.*t11.*t35.*2.0-Ixy6.*dQ1.*dQ2.*t7.*t8.*t9.*t10.*t36.*2.0-Ixy6.*dQ1.*dQ3.*t7.*t8.*t9.*t10.*t36.*2.0-Ixz6.*dQ1.*dQ2.*t2.*t3.*t5.*t9.*t11-Ixz5.*dQ1.*dQ5.*t2.*t4.*t5.*t8.*t10.*2.0-Ixz5.*dQ1.*dQ5.*t3.*t4.*t5.*t7.*t10.*2.0-Ixz6.*dQ1.*dQ3.*t2.*t3.*t5.*t9.*t11-Ixz6.*dQ1.*dQ6.*t2.*t3.*t5.*t10.*t11+Ixz6.*dQ2.*dQ3.*t4.*t5.*t6.*t9.*t10.*2.0+Ixz6.*dQ1.*dQ2.*t5.*t7.*t8.*t9.*t11+Ixz6.*dQ1.*dQ3.*t5.*t7.*t8.*t9.*t11;
et430 = Ixz6.*dQ1.*dQ5.*t2.*t8.*t9.*t10.*t11+Ixz6.*dQ1.*dQ5.*t3.*t7.*t9.*t10.*t11+Ixz6.*dQ1.*dQ6.*t5.*t7.*t8.*t10.*t11+Ixz6.*dQ1.*dQ2.*t2.*t3.*t4.*t6.*t35.*2.0+Ixz6.*dQ1.*dQ3.*t2.*t3.*t4.*t6.*t35.*2.0-Ixz5.*dQ1.*dQ2.*t2.*t5.*t8.*t10.*t34.*2.0-Ixz5.*dQ1.*dQ2.*t3.*t5.*t7.*t10.*t34.*2.0-Ixz5.*dQ1.*dQ3.*t2.*t5.*t8.*t10.*t34.*2.0-Ixz5.*dQ1.*dQ3.*t3.*t5.*t7.*t10.*t34.*2.0-Ixz6.*dQ1.*dQ2.*t4.*t6.*t7.*t8.*t35.*2.0-Ixz6.*dQ1.*dQ3.*t4.*t6.*t7.*t8.*t35.*2.0-Ixz6.*dQ1.*dQ6.*t2.*t4.*t8.*t11.*t35-Ixz6.*dQ1.*dQ6.*t3.*t4.*t7.*t11.*t35+Iyx5.*dQ1.*dQ2.*t2.*t4.*t5.*t8.*t9.*2.0+Iyx5.*dQ1.*dQ2.*t3.*t4.*t5.*t7.*t9.*2.0+Iyx5.*dQ1.*dQ3.*t2.*t4.*t5.*t8.*t9.*2.0+Iyx5.*dQ1.*dQ3.*t3.*t4.*t5.*t7.*t9.*2.0-Iyx6.*dQ1.*dQ2.*t2.*t4.*t5.*t8.*t9.*2.0-Iyx6.*dQ1.*dQ2.*t3.*t4.*t5.*t7.*t9.*2.0;
et431 = Iyx6.*dQ1.*dQ3.*t2.*t4.*t5.*t8.*t9.*-2.0-Iyx6.*dQ1.*dQ3.*t3.*t4.*t5.*t7.*t9.*2.0-Iyx6.*dQ1.*dQ6.*t2.*t4.*t5.*t8.*t10-Iyx6.*dQ1.*dQ6.*t3.*t4.*t5.*t7.*t10+Iyx6.*dQ1.*dQ2.*t2.*t3.*t9.*t10.*t36.*2.0+Iyx6.*dQ1.*dQ2.*t2.*t6.*t8.*t11.*t34.*2.0+Iyx6.*dQ1.*dQ2.*t3.*t6.*t7.*t11.*t34.*2.0+Iyx6.*dQ1.*dQ3.*t2.*t3.*t9.*t10.*t36.*2.0+Iyx6.*dQ1.*dQ3.*t2.*t6.*t8.*t11.*t34.*2.0+Iyx6.*dQ1.*dQ3.*t3.*t6.*t7.*t11.*t34.*2.0+Iyx6.*dQ1.*dQ5.*t2.*t5.*t8.*t9.*t36.*2.0+Iyx6.*dQ1.*dQ5.*t3.*t5.*t7.*t9.*t36.*2.0-Iyx6.*dQ2.*dQ3.*t4.*t6.*t9.*t11.*t35.*2.0-Iyx6.*dQ1.*dQ2.*t7.*t8.*t9.*t10.*t36.*2.0-Iyx6.*dQ1.*dQ3.*t7.*t8.*t9.*t10.*t36.*2.0+Iyy6.*dQ1.*dQ2.*t2.*t3.*t4.*t5.*t10.*2.0+Iyy6.*dQ1.*dQ3.*t2.*t3.*t4.*t5.*t10.*2.0-Iyy6.*dQ1.*dQ2.*t4.*t5.*t7.*t8.*t10.*2.0-Iyy6.*dQ1.*dQ3.*t4.*t5.*t7.*t8.*t10.*2.0;
et432 = Iyy6.*dQ2.*dQ6.*t5.*t6.*t9.*t10.*t11.*-2.0-Iyy6.*dQ3.*dQ6.*t5.*t6.*t9.*t10.*t11.*2.0-Iyy6.*dQ1.*dQ5.*t2.*t3.*t5.*t10.*t36.*2.0-Iyy6.*dQ1.*dQ6.*t2.*t3.*t6.*t11.*t35.*2.0+Iyy6.*dQ1.*dQ5.*t5.*t7.*t8.*t10.*t36.*2.0+Iyy6.*dQ1.*dQ6.*t2.*t8.*t9.*t10.*t36.*2.0+Iyy6.*dQ1.*dQ6.*t3.*t7.*t9.*t10.*t36.*2.0+Iyy6.*dQ1.*dQ6.*t6.*t7.*t8.*t11.*t35.*2.0-Iyy6.*dQ1.*dQ5.*t2.*t4.*t8.*t35.*t36.*2.0-Iyy6.*dQ1.*dQ5.*t3.*t4.*t7.*t35.*t36.*2.0-Iyy6.*dQ1.*dQ2.*t2.*t8.*t34.*t35.*t36.*2.0-Iyy6.*dQ1.*dQ2.*t3.*t7.*t34.*t35.*t36.*2.0-Iyy6.*dQ1.*dQ3.*t2.*t8.*t34.*t35.*t36.*2.0-Iyy6.*dQ1.*dQ3.*t3.*t7.*t34.*t35.*t36.*2.0-Iyz6.*dQ1.*dQ2.*t2.*t3.*t5.*t6.*t9-Iyz6.*dQ1.*dQ3.*t2.*t3.*t5.*t6.*t9-Iyz6.*dQ1.*dQ6.*t2.*t3.*t5.*t6.*t10+Iyz5.*dQ1.*dQ2.*t2.*t4.*t8.*t9.*t10.*2.0;
et433 = Iyz5.*dQ1.*dQ2.*t3.*t4.*t7.*t9.*t10.*2.0+Iyz5.*dQ1.*dQ3.*t2.*t4.*t8.*t9.*t10.*2.0+Iyz5.*dQ1.*dQ3.*t3.*t4.*t7.*t9.*t10.*2.0+Iyz6.*dQ1.*dQ2.*t5.*t6.*t7.*t8.*t9+Iyz6.*dQ1.*dQ3.*t5.*t6.*t7.*t8.*t9+Iyz6.*dQ1.*dQ5.*t2.*t6.*t8.*t9.*t10+Iyz6.*dQ1.*dQ5.*t3.*t6.*t7.*t9.*t10+Iyz6.*dQ1.*dQ6.*t5.*t6.*t7.*t8.*t10-Iyz6.*dQ2.*dQ3.*t4.*t5.*t9.*t10.*t11.*2.0-Iyz6.*dQ1.*dQ2.*t2.*t3.*t4.*t11.*t35.*2.0-Iyz6.*dQ1.*dQ3.*t2.*t3.*t4.*t11.*t35.*2.0-Iyz6.*dQ1.*dQ6.*t2.*t4.*t6.*t8.*t35-Iyz6.*dQ1.*dQ6.*t3.*t4.*t6.*t7.*t35+Iyz6.*dQ1.*dQ2.*t4.*t7.*t8.*t11.*t35.*2.0+Iyz6.*dQ1.*dQ3.*t4.*t7.*t8.*t11.*t35.*2.0-Izx6.*dQ1.*dQ2.*t2.*t3.*t5.*t9.*t11-Izx5.*dQ1.*dQ5.*t2.*t4.*t5.*t8.*t10.*2.0-Izx5.*dQ1.*dQ5.*t3.*t4.*t5.*t7.*t10.*2.0-Izx6.*dQ1.*dQ3.*t2.*t3.*t5.*t9.*t11;
et434 = -Izx6.*dQ1.*dQ6.*t2.*t3.*t5.*t10.*t11+Izx6.*dQ2.*dQ3.*t4.*t5.*t6.*t9.*t10.*2.0+Izx6.*dQ1.*dQ2.*t5.*t7.*t8.*t9.*t11+Izx6.*dQ1.*dQ3.*t5.*t7.*t8.*t9.*t11+Izx6.*dQ1.*dQ5.*t2.*t8.*t9.*t10.*t11+Izx6.*dQ1.*dQ5.*t3.*t7.*t9.*t10.*t11+Izx6.*dQ1.*dQ6.*t5.*t7.*t8.*t10.*t11+Izx6.*dQ1.*dQ2.*t2.*t3.*t4.*t6.*t35.*2.0+Izx6.*dQ1.*dQ3.*t2.*t3.*t4.*t6.*t35.*2.0-Izx5.*dQ1.*dQ2.*t2.*t5.*t8.*t10.*t34.*2.0-Izx5.*dQ1.*dQ2.*t3.*t5.*t7.*t10.*t34.*2.0-Izx5.*dQ1.*dQ3.*t2.*t5.*t8.*t10.*t34.*2.0-Izx5.*dQ1.*dQ3.*t3.*t5.*t7.*t10.*t34.*2.0-Izx6.*dQ1.*dQ2.*t4.*t6.*t7.*t8.*t35.*2.0-Izx6.*dQ1.*dQ3.*t4.*t6.*t7.*t8.*t35.*2.0-Izx6.*dQ1.*dQ6.*t2.*t4.*t8.*t11.*t35-Izx6.*dQ1.*dQ6.*t3.*t4.*t7.*t11.*t35-Izy6.*dQ1.*dQ2.*t2.*t3.*t5.*t6.*t9-Izy6.*dQ1.*dQ3.*t2.*t3.*t5.*t6.*t9;
et435 = -Izy6.*dQ1.*dQ6.*t2.*t3.*t5.*t6.*t10+Izy5.*dQ1.*dQ2.*t2.*t4.*t8.*t9.*t10.*2.0+Izy5.*dQ1.*dQ2.*t3.*t4.*t7.*t9.*t10.*2.0+Izy5.*dQ1.*dQ3.*t2.*t4.*t8.*t9.*t10.*2.0+Izy5.*dQ1.*dQ3.*t3.*t4.*t7.*t9.*t10.*2.0+Izy6.*dQ1.*dQ2.*t5.*t6.*t7.*t8.*t9+Izy6.*dQ1.*dQ3.*t5.*t6.*t7.*t8.*t9+Izy6.*dQ1.*dQ5.*t2.*t6.*t8.*t9.*t10+Izy6.*dQ1.*dQ5.*t3.*t6.*t7.*t9.*t10+Izy6.*dQ1.*dQ6.*t5.*t6.*t7.*t8.*t10-Izy6.*dQ2.*dQ3.*t4.*t5.*t9.*t10.*t11.*2.0-Izy6.*dQ1.*dQ2.*t2.*t3.*t4.*t11.*t35.*2.0-Izy6.*dQ1.*dQ3.*t2.*t3.*t4.*t11.*t35.*2.0-Izy6.*dQ1.*dQ6.*t2.*t4.*t6.*t8.*t35-Izy6.*dQ1.*dQ6.*t3.*t4.*t6.*t7.*t35+Izy6.*dQ1.*dQ2.*t4.*t7.*t8.*t11.*t35.*2.0+Izy6.*dQ1.*dQ3.*t4.*t7.*t8.*t11.*t35.*2.0-Izz5.*dQ1.*dQ2.*t2.*t3.*t4.*t5.*t10.*2.0-Izz5.*dQ1.*dQ3.*t2.*t3.*t4.*t5.*t10.*2.0;
et436 = Izz6.*dQ1.*dQ2.*t2.*t3.*t4.*t5.*t10.*-2.0-Izz6.*dQ1.*dQ3.*t2.*t3.*t4.*t5.*t10.*2.0+Izz5.*dQ1.*dQ2.*t4.*t5.*t7.*t8.*t10.*2.0+Izz5.*dQ1.*dQ3.*t4.*t5.*t7.*t8.*t10.*2.0+Izz6.*dQ1.*dQ2.*t4.*t5.*t7.*t8.*t10.*2.0+Izz6.*dQ1.*dQ3.*t4.*t5.*t7.*t8.*t10.*2.0-dQ1.*dQ5.*m5.*t2.*t3.*t5.*t10.*t16.*2.0-dQ1.*dQ5.*m6.*t2.*t3.*t5.*t10.*t20.*2.0+dQ1.*dQ6.*m6.*t2.*t3.*t6.*t11.*t17.*2.0+dQ1.*dQ5.*m6.*t2.*t3.*t5.*t10.*t22.*2.0-dQ1.*dQ6.*m6.*t2.*t3.*t6.*t11.*t20.*2.0+dQ1.*dQ5.*m5.*t2.*t3.*t5.*t10.*t25.*2.0+dQ2.*dQ5.*m6.*t4.*t5.*t6.*t11.*t17.*2.0+dQ1.*dQ5.*m5.*t5.*t7.*t8.*t10.*t16.*2.0+dQ3.*dQ5.*m6.*t4.*t5.*t6.*t11.*t17.*2.0+dQ1.*dQ5.*m6.*t2.*t3.*t5.*t10.*t26.*2.0-dQ1.*dQ6.*m6.*t2.*t8.*t9.*t10.*t17.*2.0-dQ1.*dQ6.*m6.*t3.*t7.*t9.*t10.*t17.*2.0-dQ2.*dQ5.*m6.*t4.*t5.*t6.*t11.*t20.*2.0;
et437 = dQ3.*dQ5.*m6.*t4.*t5.*t6.*t11.*t20.*-2.0+dQ1.*dQ5.*m6.*t5.*t7.*t8.*t10.*t20.*2.0-dQ1.*dQ6.*m6.*t6.*t7.*t8.*t11.*t17.*2.0-dQ1.*dQ5.*m6.*t5.*t7.*t8.*t10.*t22.*2.0+dQ1.*dQ6.*m6.*t6.*t7.*t8.*t11.*t20.*2.0-dQ1.*dQ5.*m5.*t5.*t7.*t8.*t10.*t25.*2.0-dQ1.*dQ5.*m6.*t5.*t7.*t8.*t10.*t26.*2.0-dQ1.*dQ5.*m5.*t2.*t4.*t8.*t16.*t35.*2.0-dQ1.*dQ5.*m5.*t3.*t4.*t7.*t16.*t35.*2.0-dQ1.*dQ5.*m6.*t2.*t4.*t8.*t20.*t35.*2.0-dQ1.*dQ5.*m6.*t3.*t4.*t7.*t20.*t35.*2.0+dQ1.*dQ5.*m6.*t2.*t4.*t8.*t22.*t35.*2.0+dQ1.*dQ5.*m6.*t3.*t4.*t7.*t22.*t35.*2.0+dQ2.*dQ3.*m6.*t5.*t6.*t11.*t17.*t34.*4.0+dQ1.*dQ5.*m5.*t2.*t4.*t8.*t25.*t35.*2.0+dQ1.*dQ5.*m5.*t3.*t4.*t7.*t25.*t35.*2.0+dQ1.*dQ5.*m6.*t2.*t4.*t8.*t26.*t35.*2.0+dQ1.*dQ5.*m6.*t3.*t4.*t7.*t26.*t35.*2.0-dQ2.*dQ3.*m6.*t5.*t6.*t11.*t20.*t34.*4.0;
et438 = dQ1.*dQ2.*m5.*t2.*t8.*t16.*t34.*t35.*-2.0-dQ1.*dQ2.*m5.*t3.*t7.*t16.*t34.*t35.*2.0-dQ1.*dQ3.*m5.*t2.*t8.*t16.*t34.*t35.*2.0-dQ1.*dQ3.*m5.*t3.*t7.*t16.*t34.*t35.*2.0-dQ1.*dQ2.*m6.*t2.*t8.*t17.*t34.*t36.*2.0-dQ1.*dQ2.*m6.*t3.*t7.*t17.*t34.*t36.*2.0-dQ1.*dQ3.*m6.*t2.*t8.*t17.*t34.*t36.*2.0-dQ1.*dQ3.*m6.*t3.*t7.*t17.*t34.*t36.*2.0-dQ1.*dQ2.*m6.*t2.*t8.*t20.*t34.*t35.*2.0-dQ1.*dQ2.*m6.*t3.*t7.*t20.*t34.*t35.*2.0+dQ1.*dQ2.*m6.*t2.*t8.*t20.*t34.*t36.*2.0+dQ1.*dQ2.*m6.*t3.*t7.*t20.*t34.*t36.*2.0-dQ1.*dQ3.*m6.*t2.*t8.*t20.*t34.*t35.*2.0-dQ1.*dQ3.*m6.*t3.*t7.*t20.*t34.*t35.*2.0+dQ1.*dQ2.*m6.*t2.*t8.*t22.*t34.*t35.*2.0+dQ1.*dQ2.*m6.*t3.*t7.*t22.*t34.*t35.*2.0+dQ1.*dQ3.*m6.*t2.*t8.*t20.*t34.*t36.*2.0+dQ1.*dQ3.*m6.*t3.*t7.*t20.*t34.*t36.*2.0;
et439 = dQ1.*dQ3.*m6.*t2.*t8.*t22.*t34.*t35.*2.0+dQ1.*dQ3.*m6.*t3.*t7.*t22.*t34.*t35.*2.0+dQ1.*dQ2.*m5.*t2.*t8.*t25.*t34.*t35.*2.0+dQ1.*dQ2.*m5.*t3.*t7.*t25.*t34.*t35.*2.0+dQ2.*dQ3.*m6.*t4.*t9.*t17.*t35.*t36.*2.0+dQ1.*dQ3.*m5.*t2.*t8.*t25.*t34.*t35.*2.0+dQ1.*dQ3.*m5.*t3.*t7.*t25.*t34.*t35.*2.0+dQ1.*dQ2.*m6.*t2.*t8.*t26.*t34.*t35.*2.0+dQ1.*dQ2.*m6.*t3.*t7.*t26.*t34.*t35.*2.0+dQ1.*dQ3.*m6.*t2.*t8.*t26.*t34.*t35.*2.0+dQ1.*dQ3.*m6.*t3.*t7.*t26.*t34.*t35.*2.0-dQ2.*dQ3.*m6.*t4.*t9.*t20.*t35.*t36.*2.0-Ixx6.*dQ1.*dQ2.*t2.*t3.*t6.*t9.*t10.*t11.*2.0-Ixx6.*dQ1.*dQ3.*t2.*t3.*t6.*t9.*t10.*t11.*2.0-Ixx6.*dQ1.*dQ5.*t2.*t5.*t6.*t8.*t9.*t11.*2.0-Ixx6.*dQ1.*dQ5.*t3.*t5.*t6.*t7.*t9.*t11.*2.0+Ixx6.*dQ1.*dQ2.*t6.*t7.*t8.*t9.*t10.*t11.*2.0+Ixx6.*dQ1.*dQ3.*t6.*t7.*t8.*t9.*t10.*t11.*2.0;
et440 = Ixx6.*dQ1.*dQ2.*t2.*t3.*t4.*t5.*t10.*t36.*2.0+Ixx6.*dQ1.*dQ3.*t2.*t3.*t4.*t5.*t10.*t36.*2.0-Ixx6.*dQ1.*dQ2.*t4.*t5.*t7.*t8.*t10.*t36.*2.0-Ixx6.*dQ1.*dQ3.*t4.*t5.*t7.*t8.*t10.*t36.*2.0+Ixy6.*dQ1.*dQ5.*t2.*t3.*t5.*t6.*t10.*t11.*2.0-Ixy6.*dQ1.*dQ5.*t5.*t6.*t7.*t8.*t10.*t11.*2.0-Ixy6.*dQ1.*dQ6.*t2.*t6.*t8.*t9.*t10.*t11.*2.0-Ixy6.*dQ1.*dQ6.*t3.*t6.*t7.*t9.*t10.*t11.*2.0+Ixy6.*dQ1.*dQ2.*t2.*t4.*t5.*t8.*t9.*t36.*4.0+Ixy6.*dQ1.*dQ2.*t3.*t4.*t5.*t7.*t9.*t36.*4.0+Ixy6.*dQ1.*dQ3.*t2.*t4.*t5.*t8.*t9.*t36.*4.0+Ixy6.*dQ1.*dQ3.*t3.*t4.*t5.*t7.*t9.*t36.*4.0+Ixy6.*dQ1.*dQ5.*t2.*t4.*t6.*t8.*t11.*t35.*2.0+Ixy6.*dQ1.*dQ5.*t3.*t4.*t6.*t7.*t11.*t35.*2.0+Ixy6.*dQ1.*dQ6.*t2.*t4.*t5.*t8.*t10.*t36.*2.0+Ixy6.*dQ1.*dQ6.*t3.*t4.*t5.*t7.*t10.*t36.*2.0+Ixy6.*dQ1.*dQ2.*t2.*t6.*t8.*t11.*t34.*t35.*2.0;
et441 = Ixy6.*dQ1.*dQ2.*t3.*t6.*t7.*t11.*t34.*t35.*2.0+Ixy6.*dQ1.*dQ3.*t2.*t6.*t8.*t11.*t34.*t35.*2.0+Ixy6.*dQ1.*dQ3.*t3.*t6.*t7.*t11.*t34.*t35.*2.0-Ixz6.*dQ1.*dQ5.*t2.*t4.*t5.*t6.*t8.*t10.*2.0-Ixz6.*dQ1.*dQ5.*t3.*t4.*t5.*t6.*t7.*t10.*2.0+Ixz6.*dQ1.*dQ2.*t2.*t4.*t8.*t9.*t10.*t11.*2.0+Ixz6.*dQ1.*dQ2.*t3.*t4.*t7.*t9.*t10.*t11.*2.0+Ixz6.*dQ1.*dQ3.*t2.*t4.*t8.*t9.*t10.*t11.*2.0+Ixz6.*dQ1.*dQ3.*t3.*t4.*t7.*t9.*t10.*t11.*2.0-Ixz6.*dQ1.*dQ2.*t2.*t5.*t6.*t8.*t10.*t34.*2.0-Ixz6.*dQ1.*dQ2.*t3.*t5.*t6.*t7.*t10.*t34.*2.0-Ixz6.*dQ1.*dQ3.*t2.*t5.*t6.*t8.*t10.*t34.*2.0-Ixz6.*dQ1.*dQ3.*t3.*t5.*t6.*t7.*t10.*t34.*2.0+Iyx6.*dQ1.*dQ5.*t2.*t3.*t5.*t6.*t10.*t11.*2.0-Iyx6.*dQ1.*dQ5.*t5.*t6.*t7.*t8.*t10.*t11.*2.0-Iyx6.*dQ1.*dQ6.*t2.*t6.*t8.*t9.*t10.*t11.*2.0-Iyx6.*dQ1.*dQ6.*t3.*t6.*t7.*t9.*t10.*t11.*2.0;
et442 = Iyx6.*dQ1.*dQ2.*t2.*t4.*t5.*t8.*t9.*t36.*4.0+Iyx6.*dQ1.*dQ2.*t3.*t4.*t5.*t7.*t9.*t36.*4.0+Iyx6.*dQ1.*dQ3.*t2.*t4.*t5.*t8.*t9.*t36.*4.0+Iyx6.*dQ1.*dQ3.*t3.*t4.*t5.*t7.*t9.*t36.*4.0+Iyx6.*dQ1.*dQ5.*t2.*t4.*t6.*t8.*t11.*t35.*2.0+Iyx6.*dQ1.*dQ5.*t3.*t4.*t6.*t7.*t11.*t35.*2.0+Iyx6.*dQ1.*dQ6.*t2.*t4.*t5.*t8.*t10.*t36.*2.0+Iyx6.*dQ1.*dQ6.*t3.*t4.*t5.*t7.*t10.*t36.*2.0+Iyx6.*dQ1.*dQ2.*t2.*t6.*t8.*t11.*t34.*t35.*2.0+Iyx6.*dQ1.*dQ2.*t3.*t6.*t7.*t11.*t34.*t35.*2.0+Iyx6.*dQ1.*dQ3.*t2.*t6.*t8.*t11.*t34.*t35.*2.0+Iyx6.*dQ1.*dQ3.*t3.*t6.*t7.*t11.*t34.*t35.*2.0+Iyy6.*dQ1.*dQ2.*t2.*t3.*t6.*t9.*t10.*t11.*2.0+Iyy6.*dQ1.*dQ3.*t2.*t3.*t6.*t9.*t10.*t11.*2.0+Iyy6.*dQ1.*dQ5.*t2.*t5.*t6.*t8.*t9.*t11.*2.0+Iyy6.*dQ1.*dQ5.*t3.*t5.*t6.*t7.*t9.*t11.*2.0-Iyy6.*dQ1.*dQ2.*t6.*t7.*t8.*t9.*t10.*t11.*2.0-Iyy6.*dQ1.*dQ3.*t6.*t7.*t8.*t9.*t10.*t11.*2.0;
et443 = Iyy6.*dQ1.*dQ2.*t2.*t3.*t4.*t5.*t10.*t36.*-2.0-Iyy6.*dQ1.*dQ3.*t2.*t3.*t4.*t5.*t10.*t36.*2.0+Iyy6.*dQ1.*dQ2.*t4.*t5.*t7.*t8.*t10.*t36.*2.0+Iyy6.*dQ1.*dQ3.*t4.*t5.*t7.*t8.*t10.*t36.*2.0+Iyz6.*dQ1.*dQ2.*t2.*t4.*t6.*t8.*t9.*t10.*2.0+Iyz6.*dQ1.*dQ2.*t3.*t4.*t6.*t7.*t9.*t10.*2.0+Iyz6.*dQ1.*dQ3.*t2.*t4.*t6.*t8.*t9.*t10.*2.0+Iyz6.*dQ1.*dQ3.*t3.*t4.*t6.*t7.*t9.*t10.*2.0+Iyz6.*dQ1.*dQ5.*t2.*t4.*t5.*t8.*t10.*t11.*2.0+Iyz6.*dQ1.*dQ5.*t3.*t4.*t5.*t7.*t10.*t11.*2.0+Iyz6.*dQ1.*dQ2.*t2.*t5.*t8.*t10.*t11.*t34.*2.0+Iyz6.*dQ1.*dQ2.*t3.*t5.*t7.*t10.*t11.*t34.*2.0+Iyz6.*dQ1.*dQ3.*t2.*t5.*t8.*t10.*t11.*t34.*2.0+Iyz6.*dQ1.*dQ3.*t3.*t5.*t7.*t10.*t11.*t34.*2.0-Izx6.*dQ1.*dQ5.*t2.*t4.*t5.*t6.*t8.*t10.*2.0-Izx6.*dQ1.*dQ5.*t3.*t4.*t5.*t6.*t7.*t10.*2.0+Izx6.*dQ1.*dQ2.*t2.*t4.*t8.*t9.*t10.*t11.*2.0;
et444 = Izx6.*dQ1.*dQ2.*t3.*t4.*t7.*t9.*t10.*t11.*2.0+Izx6.*dQ1.*dQ3.*t2.*t4.*t8.*t9.*t10.*t11.*2.0+Izx6.*dQ1.*dQ3.*t3.*t4.*t7.*t9.*t10.*t11.*2.0-Izx6.*dQ1.*dQ2.*t2.*t5.*t6.*t8.*t10.*t34.*2.0-Izx6.*dQ1.*dQ2.*t3.*t5.*t6.*t7.*t10.*t34.*2.0-Izx6.*dQ1.*dQ3.*t2.*t5.*t6.*t8.*t10.*t34.*2.0-Izx6.*dQ1.*dQ3.*t3.*t5.*t6.*t7.*t10.*t34.*2.0+Izy6.*dQ1.*dQ2.*t2.*t4.*t6.*t8.*t9.*t10.*2.0+Izy6.*dQ1.*dQ2.*t3.*t4.*t6.*t7.*t9.*t10.*2.0+Izy6.*dQ1.*dQ3.*t2.*t4.*t6.*t8.*t9.*t10.*2.0+Izy6.*dQ1.*dQ3.*t3.*t4.*t6.*t7.*t9.*t10.*2.0+Izy6.*dQ1.*dQ5.*t2.*t4.*t5.*t8.*t10.*t11.*2.0+Izy6.*dQ1.*dQ5.*t3.*t4.*t5.*t7.*t10.*t11.*2.0+Izy6.*dQ1.*dQ2.*t2.*t5.*t8.*t10.*t11.*t34.*2.0+Izy6.*dQ1.*dQ2.*t3.*t5.*t7.*t10.*t11.*t34.*2.0+Izy6.*dQ1.*dQ3.*t2.*t5.*t8.*t10.*t11.*t34.*2.0+Izy6.*dQ1.*dQ3.*t3.*t5.*t7.*t10.*t11.*t34.*2.0;
et445 = dQ1.*dQ2.*m5.*t2.*t3.*t4.*t5.*t10.*t16.*-2.0-dQ1.*dQ3.*m5.*t2.*t3.*t4.*t5.*t10.*t16.*2.0-dQ1.*dQ2.*m6.*t2.*t3.*t4.*t5.*t10.*t20.*2.0-dQ1.*dQ3.*m6.*t2.*t3.*t4.*t5.*t10.*t20.*2.0+dQ1.*dQ2.*m6.*t2.*t3.*t4.*t5.*t10.*t22.*2.0+dQ1.*dQ3.*m6.*t2.*t3.*t4.*t5.*t10.*t22.*2.0+dQ1.*dQ2.*m5.*t2.*t3.*t4.*t5.*t10.*t25.*2.0+dQ1.*dQ2.*m5.*t4.*t5.*t7.*t8.*t10.*t16.*2.0+dQ1.*dQ3.*m5.*t2.*t3.*t4.*t5.*t10.*t25.*2.0+dQ1.*dQ2.*m6.*t2.*t3.*t4.*t5.*t10.*t26.*2.0+dQ1.*dQ3.*m5.*t4.*t5.*t7.*t8.*t10.*t16.*2.0+dQ1.*dQ3.*m6.*t2.*t3.*t4.*t5.*t10.*t26.*2.0+dQ1.*dQ2.*m6.*t4.*t5.*t7.*t8.*t10.*t20.*2.0+dQ1.*dQ3.*m6.*t4.*t5.*t7.*t8.*t10.*t20.*2.0-dQ1.*dQ2.*m6.*t4.*t5.*t7.*t8.*t10.*t22.*2.0-dQ1.*dQ3.*m6.*t4.*t5.*t7.*t8.*t10.*t22.*2.0-dQ1.*dQ2.*m5.*t4.*t5.*t7.*t8.*t10.*t25.*2.0;
et446 = dQ1.*dQ3.*m5.*t4.*t5.*t7.*t8.*t10.*t25.*-2.0-dQ1.*dQ2.*m6.*t4.*t5.*t7.*t8.*t10.*t26.*2.0-dQ1.*dQ3.*m6.*t4.*t5.*t7.*t8.*t10.*t26.*2.0-dQ2.*dQ6.*m6.*t5.*t6.*t9.*t10.*t11.*t17.*2.0-dQ3.*dQ6.*m6.*t5.*t6.*t9.*t10.*t11.*t17.*2.0+dQ2.*dQ6.*m6.*t5.*t6.*t9.*t10.*t11.*t20.*2.0+dQ3.*dQ6.*m6.*t5.*t6.*t9.*t10.*t11.*t20.*2.0-dQ1.*dQ5.*m6.*t2.*t3.*t5.*t10.*t17.*t36.*2.0-dQ1.*dQ6.*m6.*t2.*t3.*t6.*t11.*t17.*t35.*2.0+dQ1.*dQ5.*m6.*t2.*t3.*t5.*t10.*t20.*t36.*2.0+dQ1.*dQ6.*m6.*t2.*t3.*t6.*t11.*t20.*t35.*2.0+dQ1.*dQ5.*m6.*t5.*t7.*t8.*t10.*t17.*t36.*2.0+dQ1.*dQ6.*m6.*t2.*t8.*t9.*t10.*t17.*t36.*2.0+dQ1.*dQ6.*m6.*t3.*t7.*t9.*t10.*t17.*t36.*2.0+dQ1.*dQ6.*m6.*t6.*t7.*t8.*t11.*t17.*t35.*2.0-dQ1.*dQ5.*m6.*t5.*t7.*t8.*t10.*t20.*t36.*2.0-dQ1.*dQ6.*m6.*t2.*t8.*t9.*t10.*t20.*t36.*2.0;
et447 = dQ1.*dQ6.*m6.*t3.*t7.*t9.*t10.*t20.*t36.*-2.0-dQ1.*dQ6.*m6.*t6.*t7.*t8.*t11.*t20.*t35.*2.0-dQ1.*dQ5.*m6.*t2.*t4.*t8.*t17.*t35.*t36.*2.0-dQ1.*dQ5.*m6.*t3.*t4.*t7.*t17.*t35.*t36.*2.0+dQ1.*dQ5.*m6.*t2.*t4.*t8.*t20.*t35.*t36.*2.0+dQ1.*dQ5.*m6.*t3.*t4.*t7.*t20.*t35.*t36.*2.0-dQ1.*dQ2.*m6.*t2.*t8.*t17.*t34.*t35.*t36.*2.0-dQ1.*dQ2.*m6.*t3.*t7.*t17.*t34.*t35.*t36.*2.0-dQ1.*dQ3.*m6.*t2.*t8.*t17.*t34.*t35.*t36.*2.0-dQ1.*dQ3.*m6.*t3.*t7.*t17.*t34.*t35.*t36.*2.0+dQ1.*dQ2.*m6.*t2.*t8.*t20.*t34.*t35.*t36.*2.0+dQ1.*dQ2.*m6.*t3.*t7.*t20.*t34.*t35.*t36.*2.0+dQ1.*dQ3.*m6.*t2.*t8.*t20.*t34.*t35.*t36.*2.0+dQ1.*dQ3.*m6.*t3.*t7.*t20.*t34.*t35.*t36.*2.0-Lx3.*Lxcm5.*dQ1.*dQ2.*m5.*t2.*t4.*t5.*t8.*2.0-Lx3.*Lxcm5.*dQ1.*dQ2.*m5.*t3.*t4.*t5.*t7.*2.0-Lx3.*Lxcm5.*dQ1.*dQ3.*m5.*t2.*t4.*t5.*t8.*2.0;
et448 = Lx3.*Lxcm5.*dQ1.*dQ3.*m5.*t3.*t4.*t5.*t7.*-2.0-Lx2.*Lxcm6.*dQ1.*dQ2.*m6.*t4.*t5.*t6.*t7.*2.0+Lx3.*Lxcm6.*dQ1.*dQ2.*m6.*t2.*t8.*t9.*t11.*2.0+Lx3.*Lxcm6.*dQ1.*dQ2.*m6.*t3.*t7.*t9.*t11.*2.0+Lx3.*Lxcm6.*dQ1.*dQ3.*m6.*t2.*t8.*t9.*t11.*2.0+Lx3.*Lxcm6.*dQ1.*dQ3.*m6.*t3.*t7.*t9.*t11.*2.0+Lx3.*Lycm6.*dQ1.*dQ2.*m6.*t2.*t6.*t8.*t9.*2.0+Lx3.*Lycm6.*dQ1.*dQ2.*m6.*t3.*t6.*t7.*t9.*2.0+Lx2.*Lycm6.*dQ1.*dQ2.*m6.*t4.*t5.*t7.*t11.*2.0+Lx3.*Lycm6.*dQ1.*dQ3.*m6.*t2.*t6.*t8.*t9.*2.0+Lx3.*Lycm6.*dQ1.*dQ3.*m6.*t3.*t6.*t7.*t9.*2.0+Lxcm4.*Lycm4.*dQ1.*dQ2.*m4.*t2.*t4.*t8.*t9.*4.0+Lxcm4.*Lycm4.*dQ1.*dQ2.*m4.*t3.*t4.*t7.*t9.*4.0+Lxcm4.*Lycm4.*dQ1.*dQ3.*m4.*t2.*t4.*t8.*t9.*4.0+Lxcm4.*Lycm4.*dQ1.*dQ3.*m4.*t3.*t4.*t7.*t9.*4.0+Lxcm5.*Lycm5.*dQ1.*dQ2.*m5.*t2.*t3.*t9.*t10.*2.0+Lxcm5.*Lycm5.*dQ1.*dQ3.*m5.*t2.*t3.*t9.*t10.*2.0+Lxcm5.*Lycm5.*dQ1.*dQ5.*m5.*t2.*t5.*t8.*t9.*2.0;
et449 = Lxcm5.*Lycm5.*dQ1.*dQ5.*m5.*t3.*t5.*t7.*t9.*2.0-Lxcm6.*Lycm6.*dQ1.*dQ2.*m6.*t2.*t3.*t9.*t10.*2.0-Lxcm6.*Lycm6.*dQ1.*dQ3.*m6.*t2.*t3.*t9.*t10.*2.0-Lxcm6.*Lycm6.*dQ1.*dQ2.*m6.*t2.*t6.*t8.*t11.*4.0-Lxcm6.*Lycm6.*dQ1.*dQ2.*m6.*t3.*t6.*t7.*t11.*4.0-Lxcm6.*Lycm6.*dQ1.*dQ5.*m6.*t2.*t5.*t8.*t9.*2.0-Lxcm6.*Lycm6.*dQ1.*dQ5.*m6.*t3.*t5.*t7.*t9.*2.0-Lxcm6.*Lycm6.*dQ1.*dQ3.*m6.*t2.*t6.*t8.*t11.*4.0-Lxcm6.*Lycm6.*dQ1.*dQ3.*m6.*t3.*t6.*t7.*t11.*4.0-Lxcm5.*Lycm5.*dQ1.*dQ2.*m5.*t7.*t8.*t9.*t10.*2.0-Lxcm5.*Lycm5.*dQ1.*dQ3.*m5.*t7.*t8.*t9.*t10.*2.0-Lxcm6.*Lycm6.*dQ2.*dQ3.*m6.*t4.*t6.*t9.*t11.*4.0+Lxcm6.*Lycm6.*dQ1.*dQ2.*m6.*t7.*t8.*t9.*t10.*2.0+Lxcm6.*Lycm6.*dQ1.*dQ3.*m6.*t7.*t8.*t9.*t10.*2.0-Lxcm6.*Lycm6.*dQ2.*dQ6.*m6.*t4.*t6.*t10.*t11.*4.0-Lxcm6.*Lycm6.*dQ3.*dQ6.*m6.*t4.*t6.*t10.*t11.*4.0+Lxcm6.*Lycm6.*dQ4.*dQ5.*m6.*t5.*t6.*t10.*t11.*4.0;
et450 = Lxcm6.*Lycm6.*dQ2.*dQ5.*m6.*t6.*t9.*t11.*t35.*-4.0-Lxcm6.*Lycm6.*dQ2.*dQ6.*m6.*t5.*t9.*t10.*t36.*4.0-Lxcm6.*Lycm6.*dQ3.*dQ5.*m6.*t6.*t9.*t11.*t35.*4.0-Lxcm6.*Lycm6.*dQ3.*dQ6.*m6.*t5.*t9.*t10.*t36.*4.0-Lxcm6.*Lycm6.*dQ1.*dQ6.*m6.*t2.*t3.*t35.*t36.*4.0+Lxcm6.*Lycm6.*dQ1.*dQ6.*m6.*t7.*t8.*t35.*t36.*4.0-Lx3.*Lz5.*dQ1.*dQ2.*m6.*t2.*t4.*t8.*t10.*2.0-Lx3.*Lz5.*dQ1.*dQ2.*m6.*t3.*t4.*t7.*t10.*2.0-Lx3.*Lz5.*dQ1.*dQ3.*m6.*t2.*t4.*t8.*t10.*2.0-Lx3.*Lz5.*dQ1.*dQ3.*m6.*t3.*t4.*t7.*t10.*2.0+Lxcm5.*Lz4.*dQ1.*dQ2.*m5.*t2.*t3.*t4.*t5.*2.0+Lxcm5.*Lz4.*dQ1.*dQ3.*m5.*t2.*t3.*t4.*t5.*2.0-Lxcm6.*Lz5.*dQ1.*dQ2.*m6.*t2.*t3.*t4.*t6.*2.0-Lxcm6.*Lz5.*dQ1.*dQ3.*m6.*t2.*t3.*t4.*t6.*2.0-Lx3.*Lzcm5.*dQ1.*dQ2.*m5.*t2.*t4.*t8.*t10.*2.0-Lx3.*Lzcm5.*dQ1.*dQ2.*m5.*t3.*t4.*t7.*t10.*2.0;
et451 = Lx3.*Lzcm5.*dQ1.*dQ3.*m5.*t2.*t4.*t8.*t10.*-2.0-Lx3.*Lzcm5.*dQ1.*dQ3.*m5.*t3.*t4.*t7.*t10.*2.0-Lxcm5.*Lz4.*dQ1.*dQ2.*m5.*t4.*t5.*t7.*t8.*2.0-Lx3.*Lzcm6.*dQ1.*dQ2.*m6.*t2.*t4.*t8.*t10.*2.0-Lx3.*Lzcm6.*dQ1.*dQ2.*m6.*t3.*t4.*t7.*t10.*2.0-Lxcm5.*Lz4.*dQ1.*dQ3.*m5.*t4.*t5.*t7.*t8.*2.0-Lx3.*Lzcm6.*dQ1.*dQ3.*m6.*t2.*t4.*t8.*t10.*2.0-Lx3.*Lzcm6.*dQ1.*dQ3.*m6.*t3.*t4.*t7.*t10.*2.0-Lxcm6.*Lz4.*dQ1.*dQ2.*m6.*t2.*t3.*t9.*t11.*2.0-Lxcm6.*Lz4.*dQ1.*dQ3.*m6.*t2.*t3.*t9.*t11.*2.0+Lxcm6.*Lz5.*dQ1.*dQ2.*m6.*t4.*t6.*t7.*t8.*2.0+Lxcm6.*Lz5.*dQ1.*dQ3.*m6.*t4.*t6.*t7.*t8.*2.0+Lxcm6.*Lz5.*dQ1.*dQ6.*m6.*t2.*t4.*t8.*t11.*2.0+Lxcm6.*Lz5.*dQ1.*dQ6.*m6.*t3.*t4.*t7.*t11.*2.0+Lxcm6.*Lz4.*dQ1.*dQ2.*m6.*t7.*t8.*t9.*t11.*2.0+Lxcm6.*Lz5.*dQ2.*dQ5.*m6.*t5.*t6.*t9.*t10.*4.0+Lxcm6.*Lz4.*dQ1.*dQ3.*m6.*t7.*t8.*t9.*t11.*2.0;
et452 = Lxcm6.*Lz5.*dQ3.*dQ5.*m6.*t5.*t6.*t9.*t10.*4.0+Lxcm6.*Lz5.*dQ1.*dQ5.*m6.*t2.*t3.*t6.*t35.*4.0-Lxcm6.*Lz5.*dQ1.*dQ5.*m6.*t6.*t7.*t8.*t35.*4.0-Lxcm6.*Lzcm6.*dQ1.*dQ2.*m6.*t2.*t3.*t4.*t6.*2.0-Lxcm6.*Lzcm6.*dQ1.*dQ3.*m6.*t2.*t3.*t4.*t6.*2.0+Lxcm6.*Lzcm6.*dQ1.*dQ2.*m6.*t4.*t6.*t7.*t8.*2.0+Lxcm6.*Lzcm6.*dQ1.*dQ3.*m6.*t4.*t6.*t7.*t8.*2.0+Lxcm5.*Lzcm5.*dQ2.*dQ3.*m5.*t4.*t5.*t9.*t10.*4.0+Lxcm6.*Lzcm6.*dQ1.*dQ6.*m6.*t2.*t4.*t8.*t11.*2.0+Lxcm6.*Lzcm6.*dQ1.*dQ6.*m6.*t3.*t4.*t7.*t11.*2.0+Lxcm6.*Lzcm6.*dQ2.*dQ5.*m6.*t5.*t6.*t9.*t10.*4.0+Lxcm6.*Lzcm6.*dQ3.*dQ5.*m6.*t5.*t6.*t9.*t10.*4.0+Lxcm5.*Lzcm5.*dQ1.*dQ2.*m5.*t2.*t3.*t4.*t35.*4.0+Lxcm5.*Lzcm5.*dQ1.*dQ3.*m5.*t2.*t3.*t4.*t35.*4.0+Lxcm6.*Lzcm6.*dQ1.*dQ5.*m6.*t2.*t3.*t6.*t35.*4.0-Lxcm5.*Lzcm5.*dQ1.*dQ2.*m5.*t4.*t7.*t8.*t35.*4.0-Lxcm5.*Lzcm5.*dQ1.*dQ3.*m5.*t4.*t7.*t8.*t35.*4.0;
et453 = Lxcm6.*Lzcm6.*dQ1.*dQ5.*m6.*t6.*t7.*t8.*t35.*-4.0-Lycm6.*Lz4.*dQ1.*dQ2.*m6.*t2.*t3.*t6.*t9.*2.0-Lycm6.*Lz4.*dQ1.*dQ3.*m6.*t2.*t3.*t6.*t9.*2.0+Lycm6.*Lz5.*dQ1.*dQ2.*m6.*t2.*t3.*t4.*t11.*2.0+Lycm6.*Lz5.*dQ1.*dQ3.*m6.*t2.*t3.*t4.*t11.*2.0+Lycm6.*Lz5.*dQ1.*dQ6.*m6.*t2.*t4.*t6.*t8.*2.0+Lycm6.*Lz5.*dQ1.*dQ6.*m6.*t3.*t4.*t6.*t7.*2.0+Lycm6.*Lz4.*dQ1.*dQ2.*m6.*t6.*t7.*t8.*t9.*2.0+Lycm6.*Lz4.*dQ1.*dQ3.*m6.*t6.*t7.*t8.*t9.*2.0-Lycm6.*Lz5.*dQ1.*dQ2.*m6.*t4.*t7.*t8.*t11.*2.0-Lycm6.*Lz5.*dQ1.*dQ3.*m6.*t4.*t7.*t8.*t11.*2.0-Lycm6.*Lz5.*dQ2.*dQ5.*m6.*t5.*t9.*t10.*t11.*4.0-Lycm6.*Lz5.*dQ3.*dQ5.*m6.*t5.*t9.*t10.*t11.*4.0-Lycm6.*Lz5.*dQ1.*dQ5.*m6.*t2.*t3.*t11.*t35.*4.0+Lycm6.*Lz5.*dQ1.*dQ5.*m6.*t7.*t8.*t11.*t35.*4.0-Lycm5.*Lzcm5.*dQ1.*dQ2.*m5.*t2.*t3.*t5.*t9.*2.0-Lycm5.*Lzcm5.*dQ1.*dQ3.*m5.*t2.*t3.*t5.*t9.*2.0;
et454 = Lycm6.*Lzcm6.*dQ1.*dQ2.*m6.*t2.*t3.*t4.*t11.*2.0+Lycm6.*Lzcm6.*dQ1.*dQ3.*m6.*t2.*t3.*t4.*t11.*2.0+Lycm6.*Lzcm6.*dQ1.*dQ6.*m6.*t2.*t4.*t6.*t8.*2.0+Lycm6.*Lzcm6.*dQ1.*dQ6.*m6.*t3.*t4.*t6.*t7.*2.0+Lycm5.*Lzcm5.*dQ1.*dQ2.*m5.*t5.*t7.*t8.*t9.*2.0+Lycm5.*Lzcm5.*dQ1.*dQ3.*m5.*t5.*t7.*t8.*t9.*2.0+Lycm5.*Lzcm5.*dQ1.*dQ5.*m5.*t2.*t8.*t9.*t10.*2.0+Lycm5.*Lzcm5.*dQ1.*dQ5.*m5.*t3.*t7.*t9.*t10.*2.0-Lycm6.*Lzcm6.*dQ1.*dQ2.*m6.*t4.*t7.*t8.*t11.*2.0-Lycm6.*Lzcm6.*dQ1.*dQ3.*m6.*t4.*t7.*t8.*t11.*2.0-Lycm6.*Lzcm6.*dQ2.*dQ5.*m6.*t5.*t9.*t10.*t11.*4.0-Lycm6.*Lzcm6.*dQ3.*dQ5.*m6.*t5.*t9.*t10.*t11.*4.0-Lycm6.*Lzcm6.*dQ1.*dQ5.*m6.*t2.*t3.*t11.*t35.*4.0+Lycm6.*Lzcm6.*dQ1.*dQ5.*m6.*t7.*t8.*t11.*t35.*4.0+Lz4.*Lz5.*dQ1.*dQ2.*m6.*t2.*t3.*t4.*t10.*2.0+Lz4.*Lz5.*dQ1.*dQ3.*m6.*t2.*t3.*t4.*t10.*2.0-Lz4.*Lz5.*dQ1.*dQ2.*m6.*t4.*t7.*t8.*t10.*2.0;
et455 = Lz4.*Lz5.*dQ1.*dQ3.*m6.*t4.*t7.*t8.*t10.*-2.0+Lz4.*Lzcm5.*dQ1.*dQ2.*m5.*t2.*t3.*t4.*t10.*2.0+Lz4.*Lzcm5.*dQ1.*dQ3.*m5.*t2.*t3.*t4.*t10.*2.0+Lz4.*Lzcm6.*dQ1.*dQ2.*m6.*t2.*t3.*t4.*t10.*2.0+Lz4.*Lzcm6.*dQ1.*dQ3.*m6.*t2.*t3.*t4.*t10.*2.0+Lz5.*Lzcm6.*dQ1.*dQ5.*m6.*t2.*t3.*t5.*t10.*4.0-Lz4.*Lzcm5.*dQ1.*dQ2.*m5.*t4.*t7.*t8.*t10.*2.0-Lz4.*Lzcm5.*dQ1.*dQ3.*m5.*t4.*t7.*t8.*t10.*2.0-Lz4.*Lzcm6.*dQ1.*dQ2.*m6.*t4.*t7.*t8.*t10.*2.0-Lz4.*Lzcm6.*dQ1.*dQ3.*m6.*t4.*t7.*t8.*t10.*2.0-Lz5.*Lzcm6.*dQ1.*dQ5.*m6.*t5.*t7.*t8.*t10.*4.0+Lz5.*Lzcm6.*dQ1.*dQ5.*m6.*t2.*t4.*t8.*t35.*4.0+Lz5.*Lzcm6.*dQ1.*dQ5.*m6.*t3.*t4.*t7.*t35.*4.0+Lz5.*Lzcm6.*dQ1.*dQ2.*m6.*t2.*t8.*t34.*t35.*4.0+Lz5.*Lzcm6.*dQ1.*dQ2.*m6.*t3.*t7.*t34.*t35.*4.0+Lz5.*Lzcm6.*dQ1.*dQ3.*m6.*t2.*t8.*t34.*t35.*4.0+Lz5.*Lzcm6.*dQ1.*dQ3.*m6.*t3.*t7.*t34.*t35.*4.0;
et456 = Lx3.*Lxcm6.*dQ1.*dQ2.*m6.*t2.*t4.*t5.*t6.*t8.*-2.0-Lx3.*Lxcm6.*dQ1.*dQ2.*m6.*t3.*t4.*t5.*t6.*t7.*2.0-Lx3.*Lxcm6.*dQ1.*dQ3.*m6.*t2.*t4.*t5.*t6.*t8.*2.0-Lx3.*Lxcm6.*dQ1.*dQ3.*m6.*t3.*t4.*t5.*t6.*t7.*2.0+Lx3.*Lycm6.*dQ1.*dQ2.*m6.*t2.*t4.*t5.*t8.*t11.*2.0+Lx3.*Lycm6.*dQ1.*dQ2.*m6.*t3.*t4.*t5.*t7.*t11.*2.0+Lx3.*Lycm6.*dQ1.*dQ3.*m6.*t2.*t4.*t5.*t8.*t11.*2.0+Lx3.*Lycm6.*dQ1.*dQ3.*m6.*t3.*t4.*t5.*t7.*t11.*2.0+Lxcm5.*Lycm5.*dQ1.*dQ2.*m5.*t2.*t4.*t5.*t8.*t9.*4.0+Lxcm5.*Lycm5.*dQ1.*dQ2.*m5.*t3.*t4.*t5.*t7.*t9.*4.0+Lxcm5.*Lycm5.*dQ1.*dQ3.*m5.*t2.*t4.*t5.*t8.*t9.*4.0+Lxcm5.*Lycm5.*dQ1.*dQ3.*m5.*t3.*t4.*t5.*t7.*t9.*4.0-Lxcm6.*Lycm6.*dQ1.*dQ2.*m6.*t2.*t4.*t5.*t8.*t9.*4.0-Lxcm6.*Lycm6.*dQ1.*dQ2.*m6.*t3.*t4.*t5.*t7.*t9.*4.0-Lxcm6.*Lycm6.*dQ1.*dQ3.*m6.*t2.*t4.*t5.*t8.*t9.*4.0-Lxcm6.*Lycm6.*dQ1.*dQ3.*m6.*t3.*t4.*t5.*t7.*t9.*4.0;
et457 = Lxcm6.*Lycm6.*dQ1.*dQ6.*m6.*t2.*t4.*t5.*t8.*t10.*-2.0-Lxcm6.*Lycm6.*dQ1.*dQ6.*m6.*t3.*t4.*t5.*t7.*t10.*2.0+Lxcm6.*Lycm6.*dQ1.*dQ2.*m6.*t2.*t3.*t9.*t10.*t36.*4.0+Lxcm6.*Lycm6.*dQ1.*dQ2.*m6.*t2.*t6.*t8.*t11.*t34.*4.0+Lxcm6.*Lycm6.*dQ1.*dQ2.*m6.*t3.*t6.*t7.*t11.*t34.*4.0+Lxcm6.*Lycm6.*dQ1.*dQ3.*m6.*t2.*t3.*t9.*t10.*t36.*4.0+Lxcm6.*Lycm6.*dQ1.*dQ3.*m6.*t2.*t6.*t8.*t11.*t34.*4.0+Lxcm6.*Lycm6.*dQ1.*dQ3.*m6.*t3.*t6.*t7.*t11.*t34.*4.0+Lxcm6.*Lycm6.*dQ1.*dQ5.*m6.*t2.*t5.*t8.*t9.*t36.*4.0+Lxcm6.*Lycm6.*dQ1.*dQ5.*m6.*t3.*t5.*t7.*t9.*t36.*4.0-Lxcm6.*Lycm6.*dQ2.*dQ3.*m6.*t4.*t6.*t9.*t11.*t35.*4.0-Lxcm6.*Lycm6.*dQ1.*dQ2.*m6.*t7.*t8.*t9.*t10.*t36.*4.0-Lxcm6.*Lycm6.*dQ1.*dQ3.*m6.*t7.*t8.*t9.*t10.*t36.*4.0+Lxcm6.*Lz4.*dQ1.*dQ2.*m6.*t2.*t3.*t4.*t5.*t6.*2.0+Lxcm6.*Lz4.*dQ1.*dQ3.*m6.*t2.*t3.*t4.*t5.*t6.*2.0-Lxcm6.*Lz4.*dQ1.*dQ2.*m6.*t4.*t5.*t6.*t7.*t8.*2.0;
et458 = Lxcm6.*Lz4.*dQ1.*dQ3.*m6.*t4.*t5.*t6.*t7.*t8.*-2.0-Lxcm6.*Lz5.*dQ1.*dQ2.*m6.*t2.*t3.*t5.*t9.*t11.*2.0-Lxcm6.*Lz5.*dQ1.*dQ3.*m6.*t2.*t3.*t5.*t9.*t11.*2.0-Lxcm6.*Lz5.*dQ1.*dQ6.*m6.*t2.*t3.*t5.*t10.*t11.*2.0+Lxcm6.*Lz5.*dQ2.*dQ3.*m6.*t4.*t5.*t6.*t9.*t10.*4.0+Lxcm6.*Lz5.*dQ1.*dQ2.*m6.*t5.*t7.*t8.*t9.*t11.*2.0+Lxcm6.*Lz5.*dQ1.*dQ3.*m6.*t5.*t7.*t8.*t9.*t11.*2.0+Lxcm6.*Lz5.*dQ1.*dQ5.*m6.*t2.*t8.*t9.*t10.*t11.*2.0+Lxcm6.*Lz5.*dQ1.*dQ5.*m6.*t3.*t7.*t9.*t10.*t11.*2.0+Lxcm6.*Lz5.*dQ1.*dQ6.*m6.*t5.*t7.*t8.*t10.*t11.*2.0+Lxcm6.*Lz5.*dQ1.*dQ2.*m6.*t2.*t3.*t4.*t6.*t35.*4.0+Lxcm6.*Lz5.*dQ1.*dQ3.*m6.*t2.*t3.*t4.*t6.*t35.*4.0-Lxcm6.*Lz5.*dQ1.*dQ2.*m6.*t4.*t6.*t7.*t8.*t35.*4.0-Lxcm6.*Lz5.*dQ1.*dQ3.*m6.*t4.*t6.*t7.*t8.*t35.*4.0-Lxcm6.*Lz5.*dQ1.*dQ6.*m6.*t2.*t4.*t8.*t11.*t35.*2.0-Lxcm6.*Lz5.*dQ1.*dQ6.*m6.*t3.*t4.*t7.*t11.*t35.*2.0;
et459 = Lxcm5.*Lzcm5.*dQ1.*dQ5.*m5.*t2.*t4.*t5.*t8.*t10.*-4.0-Lxcm5.*Lzcm5.*dQ1.*dQ5.*m5.*t3.*t4.*t5.*t7.*t10.*4.0-Lxcm6.*Lzcm6.*dQ1.*dQ2.*m6.*t2.*t3.*t5.*t9.*t11.*2.0-Lxcm6.*Lzcm6.*dQ1.*dQ3.*m6.*t2.*t3.*t5.*t9.*t11.*2.0-Lxcm6.*Lzcm6.*dQ1.*dQ6.*m6.*t2.*t3.*t5.*t10.*t11.*2.0+Lxcm6.*Lzcm6.*dQ2.*dQ3.*m6.*t4.*t5.*t6.*t9.*t10.*4.0+Lxcm6.*Lzcm6.*dQ1.*dQ2.*m6.*t5.*t7.*t8.*t9.*t11.*2.0+Lxcm6.*Lzcm6.*dQ1.*dQ3.*m6.*t5.*t7.*t8.*t9.*t11.*2.0+Lxcm6.*Lzcm6.*dQ1.*dQ5.*m6.*t2.*t8.*t9.*t10.*t11.*2.0+Lxcm6.*Lzcm6.*dQ1.*dQ5.*m6.*t3.*t7.*t9.*t10.*t11.*2.0+Lxcm6.*Lzcm6.*dQ1.*dQ6.*m6.*t5.*t7.*t8.*t10.*t11.*2.0+Lxcm6.*Lzcm6.*dQ1.*dQ2.*m6.*t2.*t3.*t4.*t6.*t35.*4.0+Lxcm6.*Lzcm6.*dQ1.*dQ3.*m6.*t2.*t3.*t4.*t6.*t35.*4.0-Lxcm5.*Lzcm5.*dQ1.*dQ2.*m5.*t2.*t5.*t8.*t10.*t34.*4.0-Lxcm5.*Lzcm5.*dQ1.*dQ2.*m5.*t3.*t5.*t7.*t10.*t34.*4.0-Lxcm5.*Lzcm5.*dQ1.*dQ3.*m5.*t2.*t5.*t8.*t10.*t34.*4.0;
et460 = Lxcm5.*Lzcm5.*dQ1.*dQ3.*m5.*t3.*t5.*t7.*t10.*t34.*-4.0-Lxcm6.*Lzcm6.*dQ1.*dQ2.*m6.*t4.*t6.*t7.*t8.*t35.*4.0-Lxcm6.*Lzcm6.*dQ1.*dQ3.*m6.*t4.*t6.*t7.*t8.*t35.*4.0-Lxcm6.*Lzcm6.*dQ1.*dQ6.*m6.*t2.*t4.*t8.*t11.*t35.*2.0-Lxcm6.*Lzcm6.*dQ1.*dQ6.*m6.*t3.*t4.*t7.*t11.*t35.*2.0-Lycm6.*Lz4.*dQ1.*dQ2.*m6.*t2.*t3.*t4.*t5.*t11.*2.0-Lycm6.*Lz4.*dQ1.*dQ3.*m6.*t2.*t3.*t4.*t5.*t11.*2.0-Lycm6.*Lz5.*dQ1.*dQ2.*m6.*t2.*t3.*t5.*t6.*t9.*2.0-Lycm6.*Lz5.*dQ1.*dQ3.*m6.*t2.*t3.*t5.*t6.*t9.*2.0-Lycm6.*Lz5.*dQ1.*dQ6.*m6.*t2.*t3.*t5.*t6.*t10.*2.0+Lycm6.*Lz4.*dQ1.*dQ2.*m6.*t4.*t5.*t7.*t8.*t11.*2.0+Lycm6.*Lz4.*dQ1.*dQ3.*m6.*t4.*t5.*t7.*t8.*t11.*2.0+Lycm6.*Lz5.*dQ1.*dQ2.*m6.*t5.*t6.*t7.*t8.*t9.*2.0+Lycm6.*Lz5.*dQ1.*dQ3.*m6.*t5.*t6.*t7.*t8.*t9.*2.0+Lycm6.*Lz5.*dQ1.*dQ5.*m6.*t2.*t6.*t8.*t9.*t10.*2.0;
et461 = Lycm6.*Lz5.*dQ1.*dQ5.*m6.*t3.*t6.*t7.*t9.*t10.*2.0+Lycm6.*Lz5.*dQ1.*dQ6.*m6.*t5.*t6.*t7.*t8.*t10.*2.0-Lycm6.*Lz5.*dQ2.*dQ3.*m6.*t4.*t5.*t9.*t10.*t11.*4.0-Lycm6.*Lz5.*dQ1.*dQ2.*m6.*t2.*t3.*t4.*t11.*t35.*4.0-Lycm6.*Lz5.*dQ1.*dQ3.*m6.*t2.*t3.*t4.*t11.*t35.*4.0-Lycm6.*Lz5.*dQ1.*dQ6.*m6.*t2.*t4.*t6.*t8.*t35.*2.0-Lycm6.*Lz5.*dQ1.*dQ6.*m6.*t3.*t4.*t6.*t7.*t35.*2.0+Lycm6.*Lz5.*dQ1.*dQ2.*m6.*t4.*t7.*t8.*t11.*t35.*4.0+Lycm6.*Lz5.*dQ1.*dQ3.*m6.*t4.*t7.*t8.*t11.*t35.*4.0-Lycm6.*Lzcm6.*dQ1.*dQ2.*m6.*t2.*t3.*t5.*t6.*t9.*2.0-Lycm6.*Lzcm6.*dQ1.*dQ3.*m6.*t2.*t3.*t5.*t6.*t9.*2.0+Lycm5.*Lzcm5.*dQ1.*dQ2.*m5.*t2.*t4.*t8.*t9.*t10.*4.0+Lycm5.*Lzcm5.*dQ1.*dQ2.*m5.*t3.*t4.*t7.*t9.*t10.*4.0-Lycm6.*Lzcm6.*dQ1.*dQ6.*m6.*t2.*t3.*t5.*t6.*t10.*2.0+Lycm5.*Lzcm5.*dQ1.*dQ3.*m5.*t2.*t4.*t8.*t9.*t10.*4.0+Lycm5.*Lzcm5.*dQ1.*dQ3.*m5.*t3.*t4.*t7.*t9.*t10.*4.0;
et462 = Lycm6.*Lzcm6.*dQ1.*dQ2.*m6.*t5.*t6.*t7.*t8.*t9.*2.0+Lycm6.*Lzcm6.*dQ1.*dQ3.*m6.*t5.*t6.*t7.*t8.*t9.*2.0+Lycm6.*Lzcm6.*dQ1.*dQ5.*m6.*t2.*t6.*t8.*t9.*t10.*2.0+Lycm6.*Lzcm6.*dQ1.*dQ5.*m6.*t3.*t6.*t7.*t9.*t10.*2.0+Lycm6.*Lzcm6.*dQ1.*dQ6.*m6.*t5.*t6.*t7.*t8.*t10.*2.0-Lycm6.*Lzcm6.*dQ2.*dQ3.*m6.*t4.*t5.*t9.*t10.*t11.*4.0-Lycm6.*Lzcm6.*dQ1.*dQ2.*m6.*t2.*t3.*t4.*t11.*t35.*4.0-Lycm6.*Lzcm6.*dQ1.*dQ3.*m6.*t2.*t3.*t4.*t11.*t35.*4.0-Lycm6.*Lzcm6.*dQ1.*dQ6.*m6.*t2.*t4.*t6.*t8.*t35.*2.0-Lycm6.*Lzcm6.*dQ1.*dQ6.*m6.*t3.*t4.*t6.*t7.*t35.*2.0+Lycm6.*Lzcm6.*dQ1.*dQ2.*m6.*t4.*t7.*t8.*t11.*t35.*4.0+Lycm6.*Lzcm6.*dQ1.*dQ3.*m6.*t4.*t7.*t8.*t11.*t35.*4.0+Lz5.*Lzcm6.*dQ1.*dQ2.*m6.*t2.*t3.*t4.*t5.*t10.*4.0+Lz5.*Lzcm6.*dQ1.*dQ3.*m6.*t2.*t3.*t4.*t5.*t10.*4.0-Lz5.*Lzcm6.*dQ1.*dQ2.*m6.*t4.*t5.*t7.*t8.*t10.*4.0-Lz5.*Lzcm6.*dQ1.*dQ3.*m6.*t4.*t5.*t7.*t8.*t10.*4.0;
et463 = Ixx6.*dQ1.*dQ2.*t2.*t4.*t5.*t6.*t8.*t9.*t11.*-4.0-Ixx6.*dQ1.*dQ2.*t3.*t4.*t5.*t6.*t7.*t9.*t11.*4.0-Ixx6.*dQ1.*dQ3.*t2.*t4.*t5.*t6.*t8.*t9.*t11.*4.0-Ixx6.*dQ1.*dQ3.*t3.*t4.*t5.*t6.*t7.*t9.*t11.*4.0+Ixy6.*dQ1.*dQ2.*t2.*t3.*t4.*t5.*t6.*t10.*t11.*2.0+Ixy6.*dQ1.*dQ3.*t2.*t3.*t4.*t5.*t6.*t10.*t11.*2.0-Ixy6.*dQ1.*dQ2.*t4.*t5.*t6.*t7.*t8.*t10.*t11.*2.0-Ixy6.*dQ1.*dQ3.*t4.*t5.*t6.*t7.*t8.*t10.*t11.*2.0+Iyx6.*dQ1.*dQ2.*t2.*t3.*t4.*t5.*t6.*t10.*t11.*2.0+Iyx6.*dQ1.*dQ3.*t2.*t3.*t4.*t5.*t6.*t10.*t11.*2.0-Iyx6.*dQ1.*dQ2.*t4.*t5.*t6.*t7.*t8.*t10.*t11.*2.0-Iyx6.*dQ1.*dQ3.*t4.*t5.*t6.*t7.*t8.*t10.*t11.*2.0+Iyy6.*dQ1.*dQ2.*t2.*t4.*t5.*t6.*t8.*t9.*t11.*4.0+Iyy6.*dQ1.*dQ2.*t3.*t4.*t5.*t6.*t7.*t9.*t11.*4.0+Iyy6.*dQ1.*dQ3.*t2.*t4.*t5.*t6.*t8.*t9.*t11.*4.0+Iyy6.*dQ1.*dQ3.*t3.*t4.*t5.*t6.*t7.*t9.*t11.*4.0;
et464 = dQ1.*dQ2.*m6.*t2.*t3.*t6.*t9.*t10.*t11.*t17.*2.0+dQ1.*dQ3.*m6.*t2.*t3.*t6.*t9.*t10.*t11.*t17.*2.0-dQ1.*dQ2.*m6.*t2.*t3.*t6.*t9.*t10.*t11.*t20.*2.0+dQ1.*dQ5.*m6.*t2.*t5.*t6.*t8.*t9.*t11.*t17.*2.0+dQ1.*dQ5.*m6.*t3.*t5.*t6.*t7.*t9.*t11.*t17.*2.0-dQ1.*dQ3.*m6.*t2.*t3.*t6.*t9.*t10.*t11.*t20.*2.0-dQ1.*dQ5.*m6.*t2.*t5.*t6.*t8.*t9.*t11.*t20.*2.0-dQ1.*dQ5.*m6.*t3.*t5.*t6.*t7.*t9.*t11.*t20.*2.0-dQ1.*dQ2.*m6.*t6.*t7.*t8.*t9.*t10.*t11.*t17.*2.0-dQ1.*dQ3.*m6.*t6.*t7.*t8.*t9.*t10.*t11.*t17.*2.0+dQ1.*dQ2.*m6.*t6.*t7.*t8.*t9.*t10.*t11.*t20.*2.0+dQ1.*dQ3.*m6.*t6.*t7.*t8.*t9.*t10.*t11.*t20.*2.0-dQ1.*dQ2.*m6.*t2.*t3.*t4.*t5.*t10.*t17.*t36.*2.0-dQ1.*dQ3.*m6.*t2.*t3.*t4.*t5.*t10.*t17.*t36.*2.0+dQ1.*dQ2.*m6.*t2.*t3.*t4.*t5.*t10.*t20.*t36.*2.0+dQ1.*dQ3.*m6.*t2.*t3.*t4.*t5.*t10.*t20.*t36.*2.0;
et465 = dQ1.*dQ2.*m6.*t4.*t5.*t7.*t8.*t10.*t17.*t36.*2.0+dQ1.*dQ3.*m6.*t4.*t5.*t7.*t8.*t10.*t17.*t36.*2.0-dQ1.*dQ2.*m6.*t4.*t5.*t7.*t8.*t10.*t20.*t36.*2.0-dQ1.*dQ3.*m6.*t4.*t5.*t7.*t8.*t10.*t20.*t36.*2.0+dQ1.*dQ2.*m6.*t2.*t4.*t5.*t6.*t8.*t9.*t11.*t17.*4.0+dQ1.*dQ2.*m6.*t3.*t4.*t5.*t6.*t7.*t9.*t11.*t17.*4.0+dQ1.*dQ3.*m6.*t2.*t4.*t5.*t6.*t8.*t9.*t11.*t17.*4.0+dQ1.*dQ3.*m6.*t3.*t4.*t5.*t6.*t7.*t9.*t11.*t17.*4.0-dQ1.*dQ2.*m6.*t2.*t4.*t5.*t6.*t8.*t9.*t11.*t20.*4.0-dQ1.*dQ2.*m6.*t3.*t4.*t5.*t6.*t7.*t9.*t11.*t20.*4.0-dQ1.*dQ3.*m6.*t2.*t4.*t5.*t6.*t8.*t9.*t11.*t20.*4.0-dQ1.*dQ3.*m6.*t3.*t4.*t5.*t6.*t7.*t9.*t11.*t20.*4.0-dQ1.*dQ6.*m6.*t2.*t4.*t5.*t6.*t8.*t10.*t11.*t20.*2.0-dQ1.*dQ6.*m6.*t3.*t4.*t5.*t6.*t7.*t10.*t11.*t20.*2.0+Lxcm6.*Lycm6.*dQ1.*dQ5.*m6.*t2.*t3.*t5.*t6.*t10.*t11.*4.0;
et466 = Lxcm6.*Lycm6.*dQ1.*dQ5.*m6.*t5.*t6.*t7.*t8.*t10.*t11.*-4.0-Lxcm6.*Lycm6.*dQ1.*dQ6.*m6.*t2.*t6.*t8.*t9.*t10.*t11.*4.0-Lxcm6.*Lycm6.*dQ1.*dQ6.*m6.*t3.*t6.*t7.*t9.*t10.*t11.*4.0+Lxcm6.*Lycm6.*dQ1.*dQ2.*m6.*t2.*t4.*t5.*t8.*t9.*t36.*8.0+Lxcm6.*Lycm6.*dQ1.*dQ2.*m6.*t3.*t4.*t5.*t7.*t9.*t36.*8.0+Lxcm6.*Lycm6.*dQ1.*dQ3.*m6.*t2.*t4.*t5.*t8.*t9.*t36.*8.0+Lxcm6.*Lycm6.*dQ1.*dQ3.*m6.*t3.*t4.*t5.*t7.*t9.*t36.*8.0+Lxcm6.*Lycm6.*dQ1.*dQ5.*m6.*t2.*t4.*t6.*t8.*t11.*t35.*4.0+Lxcm6.*Lycm6.*dQ1.*dQ5.*m6.*t3.*t4.*t6.*t7.*t11.*t35.*4.0+Lxcm6.*Lycm6.*dQ1.*dQ6.*m6.*t2.*t4.*t5.*t8.*t10.*t36.*4.0+Lxcm6.*Lycm6.*dQ1.*dQ6.*m6.*t3.*t4.*t5.*t7.*t10.*t36.*4.0+Lxcm6.*Lycm6.*dQ1.*dQ2.*m6.*t2.*t6.*t8.*t11.*t34.*t35.*4.0+Lxcm6.*Lycm6.*dQ1.*dQ2.*m6.*t3.*t6.*t7.*t11.*t34.*t35.*4.0+Lxcm6.*Lycm6.*dQ1.*dQ3.*m6.*t2.*t6.*t8.*t11.*t34.*t35.*4.0;
et467 = Lxcm6.*Lycm6.*dQ1.*dQ3.*m6.*t3.*t6.*t7.*t11.*t34.*t35.*4.0-Lxcm6.*Lz5.*dQ1.*dQ5.*m6.*t2.*t4.*t5.*t6.*t8.*t10.*4.0-Lxcm6.*Lz5.*dQ1.*dQ5.*m6.*t3.*t4.*t5.*t6.*t7.*t10.*4.0+Lxcm6.*Lz5.*dQ1.*dQ2.*m6.*t2.*t4.*t8.*t9.*t10.*t11.*4.0+Lxcm6.*Lz5.*dQ1.*dQ2.*m6.*t3.*t4.*t7.*t9.*t10.*t11.*4.0+Lxcm6.*Lz5.*dQ1.*dQ3.*m6.*t2.*t4.*t8.*t9.*t10.*t11.*4.0+Lxcm6.*Lz5.*dQ1.*dQ3.*m6.*t3.*t4.*t7.*t9.*t10.*t11.*4.0-Lxcm6.*Lz5.*dQ1.*dQ2.*m6.*t2.*t5.*t6.*t8.*t10.*t34.*4.0-Lxcm6.*Lz5.*dQ1.*dQ2.*m6.*t3.*t5.*t6.*t7.*t10.*t34.*4.0-Lxcm6.*Lz5.*dQ1.*dQ3.*m6.*t2.*t5.*t6.*t8.*t10.*t34.*4.0-Lxcm6.*Lz5.*dQ1.*dQ3.*m6.*t3.*t5.*t6.*t7.*t10.*t34.*4.0-Lxcm6.*Lzcm6.*dQ1.*dQ5.*m6.*t2.*t4.*t5.*t6.*t8.*t10.*4.0-Lxcm6.*Lzcm6.*dQ1.*dQ5.*m6.*t3.*t4.*t5.*t6.*t7.*t10.*4.0+Lxcm6.*Lzcm6.*dQ1.*dQ2.*m6.*t2.*t4.*t8.*t9.*t10.*t11.*4.0;
et468 = Lxcm6.*Lzcm6.*dQ1.*dQ2.*m6.*t3.*t4.*t7.*t9.*t10.*t11.*4.0+Lxcm6.*Lzcm6.*dQ1.*dQ3.*m6.*t2.*t4.*t8.*t9.*t10.*t11.*4.0+Lxcm6.*Lzcm6.*dQ1.*dQ3.*m6.*t3.*t4.*t7.*t9.*t10.*t11.*4.0-Lxcm6.*Lzcm6.*dQ1.*dQ2.*m6.*t2.*t5.*t6.*t8.*t10.*t34.*4.0-Lxcm6.*Lzcm6.*dQ1.*dQ2.*m6.*t3.*t5.*t6.*t7.*t10.*t34.*4.0-Lxcm6.*Lzcm6.*dQ1.*dQ3.*m6.*t2.*t5.*t6.*t8.*t10.*t34.*4.0-Lxcm6.*Lzcm6.*dQ1.*dQ3.*m6.*t3.*t5.*t6.*t7.*t10.*t34.*4.0+Lycm6.*Lz5.*dQ1.*dQ2.*m6.*t2.*t4.*t6.*t8.*t9.*t10.*4.0+Lycm6.*Lz5.*dQ1.*dQ2.*m6.*t3.*t4.*t6.*t7.*t9.*t10.*4.0+Lycm6.*Lz5.*dQ1.*dQ3.*m6.*t2.*t4.*t6.*t8.*t9.*t10.*4.0+Lycm6.*Lz5.*dQ1.*dQ3.*m6.*t3.*t4.*t6.*t7.*t9.*t10.*4.0+Lycm6.*Lz5.*dQ1.*dQ5.*m6.*t2.*t4.*t5.*t8.*t10.*t11.*4.0+Lycm6.*Lz5.*dQ1.*dQ5.*m6.*t3.*t4.*t5.*t7.*t10.*t11.*4.0+Lycm6.*Lz5.*dQ1.*dQ2.*m6.*t2.*t5.*t8.*t10.*t11.*t34.*4.0+Lycm6.*Lz5.*dQ1.*dQ2.*m6.*t3.*t5.*t7.*t10.*t11.*t34.*4.0;
et469 = Lycm6.*Lz5.*dQ1.*dQ3.*m6.*t2.*t5.*t8.*t10.*t11.*t34.*4.0+Lycm6.*Lz5.*dQ1.*dQ3.*m6.*t3.*t5.*t7.*t10.*t11.*t34.*4.0+Lycm6.*Lzcm6.*dQ1.*dQ2.*m6.*t2.*t4.*t6.*t8.*t9.*t10.*4.0+Lycm6.*Lzcm6.*dQ1.*dQ2.*m6.*t3.*t4.*t6.*t7.*t9.*t10.*4.0+Lycm6.*Lzcm6.*dQ1.*dQ3.*m6.*t2.*t4.*t6.*t8.*t9.*t10.*4.0+Lycm6.*Lzcm6.*dQ1.*dQ3.*m6.*t3.*t4.*t6.*t7.*t9.*t10.*4.0+Lycm6.*Lzcm6.*dQ1.*dQ5.*m6.*t2.*t4.*t5.*t8.*t10.*t11.*4.0+Lycm6.*Lzcm6.*dQ1.*dQ5.*m6.*t3.*t4.*t5.*t7.*t10.*t11.*4.0+Lycm6.*Lzcm6.*dQ1.*dQ2.*m6.*t2.*t5.*t8.*t10.*t11.*t34.*4.0+Lycm6.*Lzcm6.*dQ1.*dQ2.*m6.*t3.*t5.*t7.*t10.*t11.*t34.*4.0+Lycm6.*Lzcm6.*dQ1.*dQ3.*m6.*t2.*t5.*t8.*t10.*t11.*t34.*4.0+Lycm6.*Lzcm6.*dQ1.*dQ3.*m6.*t3.*t5.*t7.*t10.*t11.*t34.*4.0+Lxcm6.*Lycm6.*dQ1.*dQ2.*m6.*t2.*t3.*t4.*t5.*t6.*t10.*t11.*4.0+Lxcm6.*Lycm6.*dQ1.*dQ3.*m6.*t2.*t3.*t4.*t5.*t6.*t10.*t11.*4.0-Lxcm6.*Lycm6.*dQ1.*dQ2.*m6.*t4.*t5.*t6.*t7.*t8.*t10.*t11.*4.0;
et470 = Lxcm6.*Lycm6.*dQ1.*dQ3.*m6.*t4.*t5.*t6.*t7.*t8.*t10.*t11.*-4.0;
et471 = -t4.*t50-t4.*t51+t4.*t52+t4.*t53-t4.*t57-t4.*t58+t4.*t59+t4.*t60-t4.*t68-t4.*t69-t4.*t72-t4.*t73+t4.*t128+t4.*t129+t4.*t130+t4.*t131+t4.*t136+t4.*t137+t4.*t138+t4.*t139-t4.*t142-t4.*t143-t4.*t144-t4.*t145-t4.*t148-t4.*t149-t4.*t150-t4.*t151-t4.*t154-t4.*t155-t4.*t156-t4.*t157+t4.*t172+t4.*t173+t4.*t239+t4.*t240-t4.*t243-t4.*t244+t4.*t263+t4.*t264+t4.*t413+t4.*t414+t4.*t948+t4.*t949+t4.*t1236+t4.*t1237+t4.*t1808+t4.*t1809+Ixy6.*dQ5.*dQ6-Ixz5.*dQ2.*dQ3;
et472 = Iyx6.*dQ5.*dQ6-Izx5.*dQ2.*dQ3-t4.*t36.*t52.*2.0-t4.*t36.*t53.*2.0-t4.*t36.*t59.*2.0-t4.*t36.*t60.*2.0-t4.*t35.*t128.*2.0-t4.*t35.*t129.*2.0-t4.*t35.*t138.*2.0-t4.*t35.*t139.*2.0+t4.*t35.*t148.*2.0+t4.*t35.*t149.*2.0+t4.*t35.*t150.*2.0+t4.*t35.*t151.*2.0-t4.*t36.*t239.*2.0-t4.*t36.*t240.*2.0+t4.*t35.*t796+t4.*t35.*t797+t4.*t35.*t1461+t4.*t35.*t1462-t4.*t35.*t36.*t130.*2.0-t4.*t35.*t36.*t131.*2.0-Ixx5.*dQ2.*dQ4.*t9-Ixx5.*dQ3.*dQ4.*t9-Ixx6.*dQ2.*dQ4.*t9-Ixx6.*dQ3.*dQ4.*t9+Ixx6.*dQ4.*dQ6.*t10+Ixx5.*dQ2.*dQ3.*t40+Ixx6.*dQ5.*dQ6.*t41+Ixy6.*dQ2.*dQ6.*t4+Ixy6.*dQ3.*dQ6.*t4-Ixy6.*dQ5.*dQ6.*t36.*2.0-Ixz6.*dQ2.*dQ3.*t6+Ixz5.*dQ2.*dQ3.*t34+Ixz5.*dQ2.*dQ3.*t35.*2.0;
et473 = Iyx6.*dQ2.*dQ6.*t4+Iyx6.*dQ3.*dQ6.*t4-Iyx6.*dQ5.*dQ6.*t36.*2.0-Iyy5.*dQ2.*dQ4.*t9-Iyy5.*dQ3.*dQ4.*t9-Iyy6.*dQ2.*dQ4.*t9-Iyy6.*dQ3.*dQ4.*t9-Iyy6.*dQ4.*dQ6.*t10+Iyy6.*dQ2.*dQ3.*t40-Iyy6.*dQ5.*dQ6.*t41+Iyz6.*dQ2.*dQ3.*t11-Izx6.*dQ2.*dQ3.*t6+Izx5.*dQ2.*dQ3.*t34+Izx5.*dQ2.*dQ3.*t35.*2.0+Izy6.*dQ2.*dQ3.*t11+Izz5.*dQ2.*dQ4.*t9+Izz5.*dQ3.*dQ4.*t9+Izz6.*dQ2.*dQ4.*t9+Izz6.*dQ3.*dQ4.*t9+Izz6.*dQ4.*dQ6.*t10-Izz5.*dQ2.*dQ3.*t40-Izz6.*dQ2.*dQ3.*t40+Lxcm6.*Lycm6.*dQ5.*dQ6.*m6.*2.0-Lxcm5.*Lzcm5.*dQ2.*dQ3.*m5.*2.0-Ixx6.*dQ2.*dQ6.*t5.*t9-Ixx6.*dQ3.*dQ6.*t5.*t9+Ixx5.*dQ2.*dQ4.*t9.*t35.*2.0+Ixx5.*dQ3.*dQ4.*t9.*t35.*2.0-Ixx6.*dQ4.*dQ6.*t10.*t36.*2.0-Ixy6.*dQ2.*dQ6.*t4.*t36.*2.0-Ixy6.*dQ3.*dQ6.*t4.*t36.*2.0;
et474 = Ixz5.*dQ1.*dQ4.*t2.*t3-Ixz5.*dQ1.*dQ4.*t7.*t8-Ixz6.*dQ4.*dQ6.*t5.*t6+Ixz6.*dQ2.*dQ3.*t6.*t34+Ixz6.*dQ2.*dQ3.*t6.*t35.*2.0-Ixz5.*dQ2.*dQ3.*t34.*t35.*2.0-Iyx6.*dQ2.*dQ6.*t4.*t36.*2.0-Iyx6.*dQ3.*dQ6.*t4.*t36.*2.0+Iyy6.*dQ2.*dQ6.*t5.*t9+Iyy6.*dQ3.*dQ6.*t5.*t9+Iyy6.*dQ2.*dQ4.*t9.*t35.*2.0+Iyy6.*dQ3.*dQ4.*t9.*t35.*2.0+Iyy6.*dQ4.*dQ6.*t10.*t36.*2.0+Iyz6.*dQ4.*dQ6.*t5.*t11-Iyz6.*dQ2.*dQ3.*t11.*t34-Iyz6.*dQ2.*dQ3.*t11.*t35.*2.0+Izx5.*dQ1.*dQ4.*t2.*t3-Izx5.*dQ1.*dQ4.*t7.*t8-Izx6.*dQ4.*dQ6.*t5.*t6+Izx6.*dQ2.*dQ3.*t6.*t34+Izx6.*dQ2.*dQ3.*t6.*t35.*2.0-Izx5.*dQ2.*dQ3.*t34.*t35.*2.0+Izy6.*dQ4.*dQ6.*t5.*t11-Izy6.*dQ2.*dQ3.*t11.*t34-Izy6.*dQ2.*dQ3.*t11.*t35.*2.0-Izz6.*dQ2.*dQ6.*t5.*t9-Izz6.*dQ3.*dQ6.*t5.*t9;
et475 = Izz5.*dQ2.*dQ4.*t9.*t35.*-2.0-Izz5.*dQ3.*dQ4.*t9.*t35.*2.0-Izz6.*dQ2.*dQ4.*t9.*t35.*2.0-Izz6.*dQ3.*dQ4.*t9.*t35.*2.0-dQ2.*dQ4.*m6.*t9.*t22.*2.0-dQ3.*dQ4.*m6.*t9.*t22.*2.0-dQ2.*dQ4.*m5.*t9.*t25.*2.0-dQ3.*dQ4.*m5.*t9.*t25.*2.0+dQ4.*dQ6.*m6.*t10.*t20.*2.0-dQ2.*dQ4.*m6.*t9.*t26.*2.0-dQ3.*dQ4.*m6.*t9.*t26.*2.0-dQ2.*dQ3.*m5.*t16.*t40-dQ2.*dQ3.*m6.*t20.*t40+dQ2.*dQ3.*m6.*t22.*t40+dQ2.*dQ3.*m5.*t25.*t40-dQ5.*dQ6.*m6.*t17.*t41+dQ2.*dQ3.*m6.*t26.*t40+dQ5.*dQ6.*m6.*t20.*t41+t5.*t6.*t9.*t11.*t130.*2.0+t5.*t6.*t9.*t11.*t131.*2.0-t5.*t6.*t9.*t11.*t138.*2.0-t5.*t6.*t9.*t11.*t139.*2.0+Lxcm6.*Lycm6.*dQ2.*dQ6.*m6.*t4.*2.0+Lxcm6.*Lycm6.*dQ3.*dQ6.*m6.*t4.*2.0-Lxcm6.*Lycm6.*dQ5.*dQ6.*m6.*t36.*4.0+Lxcm5.*Lz4.*dQ2.*dQ3.*m5.*t5.*2.0;
et476 = Lxcm6.*Lz5.*dQ2.*dQ3.*m6.*t6.*-2.0-Lxcm6.*Lzcm6.*dQ2.*dQ3.*m6.*t6.*2.0+Lxcm5.*Lzcm5.*dQ2.*dQ3.*m5.*t34.*2.0+Lxcm5.*Lzcm5.*dQ2.*dQ3.*m5.*t35.*4.0+Lycm6.*Lz5.*dQ2.*dQ3.*m6.*t11.*2.0+Lycm6.*Lzcm6.*dQ2.*dQ3.*m6.*t11.*2.0+Lz4.*Lz5.*dQ2.*dQ3.*m6.*t10.*2.0+Lz4.*Lzcm5.*dQ2.*dQ3.*m5.*t10.*2.0+Lz4.*Lzcm6.*dQ2.*dQ3.*m6.*t10.*2.0-Lz5.*Lzcm6.*dQ2.*dQ4.*m6.*t9.*4.0-Lz5.*Lzcm6.*dQ3.*dQ4.*m6.*t9.*4.0+Lz5.*Lzcm6.*dQ2.*dQ3.*m6.*t40.*2.0-Ixx5.*dQ1.*dQ2.*t2.*t3.*t9-Ixx5.*dQ1.*dQ3.*t2.*t3.*t9+Ixx6.*dQ1.*dQ2.*t2.*t3.*t9+Ixx6.*dQ1.*dQ3.*t2.*t3.*t9+Ixx6.*dQ1.*dQ6.*t2.*t3.*t10+Ixx5.*dQ1.*dQ2.*t7.*t8.*t9+Ixx5.*dQ1.*dQ3.*t7.*t8.*t9-Ixx6.*dQ1.*dQ2.*t7.*t8.*t9-Ixx6.*dQ1.*dQ3.*t7.*t8.*t9+Ixx6.*dQ2.*dQ6.*t4.*t6.*t11.*2.0+Ixx6.*dQ3.*dQ6.*t4.*t6.*t11.*2.0-Ixx6.*dQ1.*dQ6.*t7.*t8.*t10;
et477 = Ixx5.*dQ2.*dQ3.*t5.*t10.*t34.*-2.0+Ixx6.*dQ2.*dQ3.*t5.*t10.*t36.*2.0+Ixx6.*dQ2.*dQ6.*t5.*t9.*t36.*2.0+Ixx6.*dQ3.*dQ6.*t5.*t9.*t36.*2.0+Ixx6.*dQ2.*dQ4.*t9.*t35.*t36.*2.0+Ixx6.*dQ3.*dQ4.*t9.*t35.*t36.*2.0-Ixy5.*dQ1.*dQ2.*t2.*t8.*t10-Ixy5.*dQ1.*dQ2.*t3.*t7.*t10-Ixy5.*dQ1.*dQ3.*t2.*t8.*t10-Ixy5.*dQ1.*dQ3.*t3.*t7.*t10+Ixy6.*dQ1.*dQ2.*t2.*t8.*t10+Ixy6.*dQ1.*dQ2.*t3.*t7.*t10+Ixy6.*dQ1.*dQ3.*t2.*t8.*t10+Ixy6.*dQ1.*dQ3.*t3.*t7.*t10+Ixy6.*dQ1.*dQ6.*t2.*t8.*t9+Ixy6.*dQ1.*dQ6.*t3.*t7.*t9-Ixy5.*dQ2.*dQ3.*t4.*t9.*t10+Ixy6.*dQ2.*dQ3.*t4.*t9.*t10-Ixy6.*dQ4.*dQ6.*t6.*t10.*t11.*2.0+Ixz6.*dQ1.*dQ4.*t2.*t3.*t6-Ixz6.*dQ1.*dQ4.*t6.*t7.*t8-Ixz5.*dQ2.*dQ4.*t5.*t9.*t10.*2.0-Ixz5.*dQ3.*dQ4.*t5.*t9.*t10.*2.0-Ixz6.*dQ2.*dQ6.*t6.*t9.*t10;
et478 = -Ixz6.*dQ3.*dQ6.*t6.*t9.*t10-Ixz5.*dQ1.*dQ4.*t2.*t3.*t35.*2.0+Ixz5.*dQ1.*dQ4.*t7.*t8.*t35.*2.0-Ixz6.*dQ2.*dQ3.*t6.*t34.*t35.*2.0-Iyx5.*dQ1.*dQ2.*t2.*t8.*t10-Iyx5.*dQ1.*dQ2.*t3.*t7.*t10-Iyx5.*dQ1.*dQ3.*t2.*t8.*t10-Iyx5.*dQ1.*dQ3.*t3.*t7.*t10+Iyx6.*dQ1.*dQ2.*t2.*t8.*t10+Iyx6.*dQ1.*dQ2.*t3.*t7.*t10+Iyx6.*dQ1.*dQ3.*t2.*t8.*t10+Iyx6.*dQ1.*dQ3.*t3.*t7.*t10+Iyx6.*dQ1.*dQ6.*t2.*t8.*t9+Iyx6.*dQ1.*dQ6.*t3.*t7.*t9-Iyx5.*dQ2.*dQ3.*t4.*t9.*t10+Iyx6.*dQ2.*dQ3.*t4.*t9.*t10-Iyx6.*dQ4.*dQ6.*t6.*t10.*t11.*2.0+Iyy5.*dQ1.*dQ2.*t2.*t3.*t9+Iyy5.*dQ1.*dQ3.*t2.*t3.*t9-Iyy6.*dQ1.*dQ2.*t2.*t3.*t9-Iyy6.*dQ1.*dQ3.*t2.*t3.*t9-Iyy6.*dQ1.*dQ6.*t2.*t3.*t10-Iyy5.*dQ1.*dQ2.*t7.*t8.*t9-Iyy5.*dQ1.*dQ3.*t7.*t8.*t9;
et479 = Iyy6.*dQ1.*dQ2.*t7.*t8.*t9+Iyy6.*dQ1.*dQ3.*t7.*t8.*t9-Iyy6.*dQ2.*dQ6.*t4.*t6.*t11.*2.0-Iyy6.*dQ3.*dQ6.*t4.*t6.*t11.*2.0+Iyy6.*dQ1.*dQ6.*t7.*t8.*t10-Iyy6.*dQ2.*dQ3.*t5.*t10.*t34.*2.0-Iyy6.*dQ2.*dQ3.*t5.*t10.*t36.*2.0-Iyy6.*dQ2.*dQ6.*t5.*t9.*t36.*2.0-Iyy6.*dQ3.*dQ6.*t5.*t9.*t36.*2.0-Iyy6.*dQ2.*dQ4.*t9.*t35.*t36.*2.0-Iyy6.*dQ3.*dQ4.*t9.*t35.*t36.*2.0+Iyz5.*dQ1.*dQ2.*t2.*t5.*t8+Iyz5.*dQ1.*dQ2.*t3.*t5.*t7+Iyz5.*dQ1.*dQ3.*t2.*t5.*t8+Iyz5.*dQ1.*dQ3.*t3.*t5.*t7-Iyz6.*dQ1.*dQ4.*t2.*t3.*t11+Iyz5.*dQ2.*dQ3.*t4.*t5.*t9+Iyz6.*dQ1.*dQ4.*t7.*t8.*t11+Iyz6.*dQ2.*dQ6.*t9.*t10.*t11+Iyz6.*dQ3.*dQ6.*t9.*t10.*t11+Iyz6.*dQ2.*dQ3.*t11.*t34.*t35.*2.0+Izx6.*dQ1.*dQ4.*t2.*t3.*t6-Izx6.*dQ1.*dQ4.*t6.*t7.*t8-Izx5.*dQ2.*dQ4.*t5.*t9.*t10.*2.0-Izx5.*dQ3.*dQ4.*t5.*t9.*t10.*2.0;
et480 = -Izx6.*dQ2.*dQ6.*t6.*t9.*t10-Izx6.*dQ3.*dQ6.*t6.*t9.*t10-Izx5.*dQ1.*dQ4.*t2.*t3.*t35.*2.0+Izx5.*dQ1.*dQ4.*t7.*t8.*t35.*2.0-Izx6.*dQ2.*dQ3.*t6.*t34.*t35.*2.0+Izy5.*dQ1.*dQ2.*t2.*t5.*t8+Izy5.*dQ1.*dQ2.*t3.*t5.*t7+Izy5.*dQ1.*dQ3.*t2.*t5.*t8+Izy5.*dQ1.*dQ3.*t3.*t5.*t7-Izy6.*dQ1.*dQ4.*t2.*t3.*t11+Izy5.*dQ2.*dQ3.*t4.*t5.*t9+Izy6.*dQ1.*dQ4.*t7.*t8.*t11+Izy6.*dQ2.*dQ6.*t9.*t10.*t11+Izy6.*dQ3.*dQ6.*t9.*t10.*t11+Izy6.*dQ2.*dQ3.*t11.*t34.*t35.*2.0+Izz5.*dQ1.*dQ2.*t2.*t3.*t9+Izz5.*dQ1.*dQ3.*t2.*t3.*t9+Izz6.*dQ1.*dQ2.*t2.*t3.*t9+Izz6.*dQ1.*dQ3.*t2.*t3.*t9+Izz6.*dQ1.*dQ6.*t2.*t3.*t10-Izz5.*dQ1.*dQ2.*t7.*t8.*t9-Izz5.*dQ1.*dQ3.*t7.*t8.*t9-Izz6.*dQ1.*dQ2.*t7.*t8.*t9-Izz6.*dQ1.*dQ3.*t7.*t8.*t9-Izz6.*dQ1.*dQ6.*t7.*t8.*t10;
et481 = Izz5.*dQ2.*dQ3.*t5.*t10.*t34.*2.0+Izz6.*dQ2.*dQ3.*t5.*t10.*t34.*2.0-dQ2.*dQ6.*m6.*t5.*t9.*t20.*2.0-dQ3.*dQ6.*m6.*t5.*t9.*t20.*2.0-dQ2.*dQ4.*m5.*t9.*t16.*t35.*2.0-dQ3.*dQ4.*m5.*t9.*t16.*t35.*2.0-dQ2.*dQ4.*m6.*t9.*t20.*t35.*2.0-dQ3.*dQ4.*m6.*t9.*t20.*t35.*2.0+dQ2.*dQ4.*m6.*t9.*t22.*t35.*2.0+dQ3.*dQ4.*m6.*t9.*t22.*t35.*2.0+dQ4.*dQ6.*m6.*t10.*t17.*t36.*2.0+dQ2.*dQ4.*m5.*t9.*t25.*t35.*2.0+dQ3.*dQ4.*m5.*t9.*t25.*t35.*2.0+dQ2.*dQ4.*m6.*t9.*t26.*t35.*2.0-dQ4.*dQ6.*m6.*t10.*t20.*t36.*2.0+dQ3.*dQ4.*m6.*t9.*t26.*t35.*2.0+Lx3.*Lxcm5.*dQ2.*dQ3.*m5.*t4.*t10.*2.0-Lxcm5.*Lycm5.*dQ2.*dQ4.*m5.*t4.*t5.*2.0-Lxcm5.*Lycm5.*dQ3.*dQ4.*m5.*t4.*t5.*2.0-Lxcm6.*Lycm6.*dQ2.*dQ6.*m6.*t4.*t36.*4.0-Lxcm6.*Lycm6.*dQ3.*dQ6.*m6.*t4.*t36.*4.0-Lx3.*Lz5.*dQ2.*dQ3.*m6.*t4.*t5.*2.0;
et482 = Lx3.*Lzcm5.*dQ2.*dQ3.*m5.*t4.*t5.*-2.0-Lx3.*Lzcm6.*dQ2.*dQ3.*m6.*t4.*t5.*2.0+Lxcm6.*Lz4.*dQ2.*dQ3.*m6.*t5.*t6.*2.0-Lxcm6.*Lz5.*dQ4.*dQ6.*m6.*t5.*t6.*2.0+Lxcm6.*Lz5.*dQ2.*dQ3.*m6.*t6.*t34.*2.0+Lxcm6.*Lz5.*dQ2.*dQ3.*m6.*t6.*t35.*4.0+Lxcm5.*Lzcm5.*dQ1.*dQ4.*m5.*t2.*t3.*2.0-Lxcm5.*Lzcm5.*dQ1.*dQ4.*m5.*t7.*t8.*2.0-Lxcm6.*Lzcm6.*dQ4.*dQ6.*m6.*t5.*t6.*2.0+Lxcm6.*Lzcm6.*dQ2.*dQ3.*m6.*t6.*t34.*2.0+Lxcm6.*Lzcm6.*dQ2.*dQ3.*m6.*t6.*t35.*4.0-Lxcm5.*Lzcm5.*dQ2.*dQ3.*m5.*t34.*t35.*4.0-Lycm6.*Lz4.*dQ2.*dQ3.*m6.*t5.*t11.*2.0+Lycm6.*Lz5.*dQ4.*dQ6.*m6.*t5.*t11.*2.0-Lycm6.*Lz5.*dQ2.*dQ3.*m6.*t11.*t34.*2.0-Lycm6.*Lz5.*dQ2.*dQ3.*m6.*t11.*t35.*4.0-Lycm5.*Lzcm5.*dQ2.*dQ4.*m5.*t4.*t10.*2.0-Lycm5.*Lzcm5.*dQ3.*dQ4.*m5.*t4.*t10.*2.0+Lycm6.*Lzcm6.*dQ4.*dQ6.*m6.*t5.*t11.*2.0-Lycm6.*Lzcm6.*dQ2.*dQ3.*m6.*t11.*t34.*2.0;
et483 = Lycm6.*Lzcm6.*dQ2.*dQ3.*m6.*t11.*t35.*-4.0+Lz5.*Lzcm6.*dQ2.*dQ4.*m6.*t9.*t35.*4.0+Lz5.*Lzcm6.*dQ3.*dQ4.*m6.*t9.*t35.*4.0-Ixx5.*dQ1.*dQ4.*t2.*t3.*t5.*t10.*2.0+Ixx5.*dQ1.*dQ4.*t5.*t7.*t8.*t10.*2.0+Ixx5.*dQ1.*dQ2.*t2.*t3.*t9.*t35.*2.0+Ixx5.*dQ1.*dQ3.*t2.*t3.*t9.*t35.*2.0-Ixx6.*dQ1.*dQ2.*t2.*t3.*t9.*t36.*2.0-Ixx6.*dQ1.*dQ3.*t2.*t3.*t9.*t36.*2.0-Ixx6.*dQ1.*dQ6.*t2.*t3.*t10.*t36.*2.0-Ixx5.*dQ1.*dQ2.*t7.*t8.*t9.*t35.*2.0-Ixx5.*dQ1.*dQ3.*t7.*t8.*t9.*t35.*2.0+Ixx6.*dQ1.*dQ2.*t7.*t8.*t9.*t36.*2.0+Ixx6.*dQ1.*dQ3.*t7.*t8.*t9.*t36.*2.0+Ixx6.*dQ1.*dQ6.*t7.*t8.*t10.*t36.*2.0-Ixx6.*dQ2.*dQ3.*t5.*t10.*t34.*t36.*2.0-Ixy5.*dQ1.*dQ4.*t2.*t5.*t8.*t9-Ixy5.*dQ1.*dQ4.*t3.*t5.*t7.*t9+Ixy6.*dQ1.*dQ4.*t2.*t5.*t8.*t9+Ixy6.*dQ1.*dQ4.*t3.*t5.*t7.*t9+Ixy6.*dQ2.*dQ3.*t5.*t6.*t10.*t11.*2.0;
et484 = Ixy6.*dQ2.*dQ6.*t5.*t6.*t9.*t11.*2.0+Ixy6.*dQ3.*dQ6.*t5.*t6.*t9.*t11.*2.0+Ixy5.*dQ1.*dQ2.*t2.*t8.*t10.*t34+Ixy5.*dQ1.*dQ2.*t3.*t7.*t10.*t34+Ixy5.*dQ1.*dQ3.*t2.*t8.*t10.*t34+Ixy5.*dQ1.*dQ3.*t3.*t7.*t10.*t34-Ixy6.*dQ1.*dQ2.*t2.*t8.*t10.*t34-Ixy6.*dQ1.*dQ2.*t3.*t7.*t10.*t34-Ixy6.*dQ1.*dQ3.*t2.*t8.*t10.*t34-Ixy6.*dQ1.*dQ3.*t3.*t7.*t10.*t34-Ixy6.*dQ1.*dQ2.*t2.*t8.*t10.*t36.*2.0-Ixy6.*dQ1.*dQ2.*t3.*t7.*t10.*t36.*2.0-Ixy6.*dQ1.*dQ3.*t2.*t8.*t10.*t36.*2.0-Ixy6.*dQ1.*dQ3.*t3.*t7.*t10.*t36.*2.0-Ixy6.*dQ1.*dQ6.*t2.*t8.*t9.*t36.*2.0-Ixy6.*dQ1.*dQ6.*t3.*t7.*t9.*t36.*2.0-Ixy6.*dQ2.*dQ3.*t4.*t9.*t10.*t36.*2.0+Ixy6.*dQ2.*dQ4.*t6.*t9.*t11.*t35.*2.0+Ixy6.*dQ3.*dQ4.*t6.*t9.*t11.*t35.*2.0-Ixz6.*dQ1.*dQ6.*t2.*t3.*t5.*t6+Ixz5.*dQ1.*dQ2.*t2.*t4.*t8.*t9;
et485 = Ixz5.*dQ1.*dQ2.*t3.*t4.*t7.*t9+Ixz5.*dQ1.*dQ3.*t2.*t4.*t8.*t9+Ixz5.*dQ1.*dQ3.*t3.*t4.*t7.*t9+Ixz6.*dQ1.*dQ2.*t2.*t5.*t8.*t11+Ixz6.*dQ1.*dQ2.*t3.*t5.*t7.*t11+Ixz6.*dQ1.*dQ3.*t2.*t5.*t8.*t11+Ixz6.*dQ1.*dQ3.*t3.*t5.*t7.*t11+Ixz6.*dQ1.*dQ6.*t5.*t6.*t7.*t8+Ixz6.*dQ2.*dQ3.*t4.*t5.*t9.*t11-Ixz6.*dQ2.*dQ4.*t5.*t6.*t9.*t10.*2.0-Ixz6.*dQ3.*dQ4.*t5.*t6.*t9.*t10.*2.0-Ixz6.*dQ1.*dQ4.*t2.*t3.*t6.*t35.*2.0+Ixz6.*dQ1.*dQ4.*t6.*t7.*t8.*t35.*2.0-Iyx5.*dQ1.*dQ4.*t2.*t5.*t8.*t9-Iyx5.*dQ1.*dQ4.*t3.*t5.*t7.*t9+Iyx6.*dQ1.*dQ4.*t2.*t5.*t8.*t9+Iyx6.*dQ1.*dQ4.*t3.*t5.*t7.*t9+Iyx6.*dQ2.*dQ3.*t5.*t6.*t10.*t11.*2.0+Iyx6.*dQ2.*dQ6.*t5.*t6.*t9.*t11.*2.0+Iyx6.*dQ3.*dQ6.*t5.*t6.*t9.*t11.*2.0+Iyx5.*dQ1.*dQ2.*t2.*t8.*t10.*t34+Iyx5.*dQ1.*dQ2.*t3.*t7.*t10.*t34+Iyx5.*dQ1.*dQ3.*t2.*t8.*t10.*t34;
et486 = Iyx5.*dQ1.*dQ3.*t3.*t7.*t10.*t34-Iyx6.*dQ1.*dQ2.*t2.*t8.*t10.*t34-Iyx6.*dQ1.*dQ2.*t3.*t7.*t10.*t34-Iyx6.*dQ1.*dQ3.*t2.*t8.*t10.*t34-Iyx6.*dQ1.*dQ3.*t3.*t7.*t10.*t34-Iyx6.*dQ1.*dQ2.*t2.*t8.*t10.*t36.*2.0-Iyx6.*dQ1.*dQ2.*t3.*t7.*t10.*t36.*2.0-Iyx6.*dQ1.*dQ3.*t2.*t8.*t10.*t36.*2.0-Iyx6.*dQ1.*dQ3.*t3.*t7.*t10.*t36.*2.0-Iyx6.*dQ1.*dQ6.*t2.*t8.*t9.*t36.*2.0-Iyx6.*dQ1.*dQ6.*t3.*t7.*t9.*t36.*2.0-Iyx6.*dQ2.*dQ3.*t4.*t9.*t10.*t36.*2.0+Iyx6.*dQ2.*dQ4.*t6.*t9.*t11.*t35.*2.0+Iyx6.*dQ3.*dQ4.*t6.*t9.*t11.*t35.*2.0-Iyy6.*dQ1.*dQ4.*t2.*t3.*t5.*t10.*2.0-Iyy6.*dQ2.*dQ4.*t4.*t5.*t6.*t11.*2.0-Iyy6.*dQ3.*dQ4.*t4.*t5.*t6.*t11.*2.0+Iyy6.*dQ1.*dQ4.*t5.*t7.*t8.*t10.*2.0+Iyy6.*dQ1.*dQ2.*t2.*t3.*t9.*t35.*2.0+Iyy6.*dQ1.*dQ2.*t2.*t3.*t9.*t36.*2.0;
et487 = Iyy6.*dQ1.*dQ3.*t2.*t3.*t9.*t35.*2.0+Iyy6.*dQ1.*dQ3.*t2.*t3.*t9.*t36.*2.0+Iyy6.*dQ1.*dQ6.*t2.*t3.*t10.*t36.*2.0-Iyy6.*dQ1.*dQ2.*t7.*t8.*t9.*t35.*2.0-Iyy6.*dQ1.*dQ2.*t7.*t8.*t9.*t36.*2.0-Iyy6.*dQ1.*dQ3.*t7.*t8.*t9.*t35.*2.0-Iyy6.*dQ1.*dQ3.*t7.*t8.*t9.*t36.*2.0-Iyy6.*dQ1.*dQ6.*t7.*t8.*t10.*t36.*2.0+Iyy6.*dQ2.*dQ3.*t5.*t10.*t34.*t36.*2.0+Iyz6.*dQ1.*dQ2.*t2.*t5.*t6.*t8+Iyz6.*dQ1.*dQ2.*t3.*t5.*t6.*t7+Iyz6.*dQ1.*dQ3.*t2.*t5.*t6.*t8+Iyz6.*dQ1.*dQ3.*t3.*t5.*t6.*t7+Iyz6.*dQ1.*dQ6.*t2.*t3.*t5.*t11+Iyz6.*dQ2.*dQ3.*t4.*t5.*t6.*t9-Iyz5.*dQ1.*dQ4.*t2.*t8.*t9.*t10-Iyz5.*dQ1.*dQ4.*t3.*t7.*t9.*t10-Iyz6.*dQ1.*dQ6.*t5.*t7.*t8.*t11+Iyz6.*dQ2.*dQ4.*t5.*t9.*t10.*t11.*2.0+Iyz6.*dQ3.*dQ4.*t5.*t9.*t10.*t11.*2.0-Iyz5.*dQ1.*dQ2.*t2.*t5.*t8.*t34;
et488 = -Iyz5.*dQ1.*dQ2.*t3.*t5.*t7.*t34-Iyz5.*dQ1.*dQ3.*t2.*t5.*t8.*t34-Iyz5.*dQ1.*dQ3.*t3.*t5.*t7.*t34+Iyz6.*dQ1.*dQ4.*t2.*t3.*t11.*t35.*2.0-Iyz6.*dQ1.*dQ4.*t7.*t8.*t11.*t35.*2.0-Izx6.*dQ1.*dQ6.*t2.*t3.*t5.*t6+Izx5.*dQ1.*dQ2.*t2.*t4.*t8.*t9+Izx5.*dQ1.*dQ2.*t3.*t4.*t7.*t9+Izx5.*dQ1.*dQ3.*t2.*t4.*t8.*t9+Izx5.*dQ1.*dQ3.*t3.*t4.*t7.*t9+Izx6.*dQ1.*dQ2.*t2.*t5.*t8.*t11+Izx6.*dQ1.*dQ2.*t3.*t5.*t7.*t11+Izx6.*dQ1.*dQ3.*t2.*t5.*t8.*t11+Izx6.*dQ1.*dQ3.*t3.*t5.*t7.*t11+Izx6.*dQ1.*dQ6.*t5.*t6.*t7.*t8+Izx6.*dQ2.*dQ3.*t4.*t5.*t9.*t11-Izx6.*dQ2.*dQ4.*t5.*t6.*t9.*t10.*2.0-Izx6.*dQ3.*dQ4.*t5.*t6.*t9.*t10.*2.0-Izx6.*dQ1.*dQ4.*t2.*t3.*t6.*t35.*2.0+Izx6.*dQ1.*dQ4.*t6.*t7.*t8.*t35.*2.0+Izy6.*dQ1.*dQ2.*t2.*t5.*t6.*t8+Izy6.*dQ1.*dQ2.*t3.*t5.*t6.*t7;
et489 = Izy6.*dQ1.*dQ3.*t2.*t5.*t6.*t8+Izy6.*dQ1.*dQ3.*t3.*t5.*t6.*t7+Izy6.*dQ1.*dQ6.*t2.*t3.*t5.*t11+Izy6.*dQ2.*dQ3.*t4.*t5.*t6.*t9-Izy5.*dQ1.*dQ4.*t2.*t8.*t9.*t10-Izy5.*dQ1.*dQ4.*t3.*t7.*t9.*t10-Izy6.*dQ1.*dQ6.*t5.*t7.*t8.*t11+Izy6.*dQ2.*dQ4.*t5.*t9.*t10.*t11.*2.0+Izy6.*dQ3.*dQ4.*t5.*t9.*t10.*t11.*2.0-Izy5.*dQ1.*dQ2.*t2.*t5.*t8.*t34-Izy5.*dQ1.*dQ2.*t3.*t5.*t7.*t34-Izy5.*dQ1.*dQ3.*t2.*t5.*t8.*t34-Izy5.*dQ1.*dQ3.*t3.*t5.*t7.*t34+Izy6.*dQ1.*dQ4.*t2.*t3.*t11.*t35.*2.0-Izy6.*dQ1.*dQ4.*t7.*t8.*t11.*t35.*2.0+Izz5.*dQ1.*dQ4.*t2.*t3.*t5.*t10.*2.0+Izz6.*dQ1.*dQ4.*t2.*t3.*t5.*t10.*2.0-Izz5.*dQ1.*dQ4.*t5.*t7.*t8.*t10.*2.0-Izz6.*dQ1.*dQ4.*t5.*t7.*t8.*t10.*2.0-Izz5.*dQ1.*dQ2.*t2.*t3.*t9.*t35.*2.0-Izz5.*dQ1.*dQ3.*t2.*t3.*t9.*t35.*2.0;
et490 = Izz6.*dQ1.*dQ2.*t2.*t3.*t9.*t35.*-2.0-Izz6.*dQ1.*dQ3.*t2.*t3.*t9.*t35.*2.0+Izz5.*dQ1.*dQ2.*t7.*t8.*t9.*t35.*2.0+Izz5.*dQ1.*dQ3.*t7.*t8.*t9.*t35.*2.0+Izz6.*dQ1.*dQ2.*t7.*t8.*t9.*t35.*2.0+Izz6.*dQ1.*dQ3.*t7.*t8.*t9.*t35.*2.0+dQ1.*dQ2.*m5.*t2.*t3.*t9.*t16.*2.0+dQ1.*dQ3.*m5.*t2.*t3.*t9.*t16.*2.0+dQ1.*dQ2.*m6.*t2.*t3.*t9.*t20.*2.0+dQ1.*dQ3.*m6.*t2.*t3.*t9.*t20.*2.0+dQ1.*dQ4.*m6.*t2.*t4.*t8.*t22.*2.0+dQ1.*dQ4.*m6.*t3.*t4.*t7.*t22.*2.0-dQ1.*dQ2.*m5.*t7.*t8.*t9.*t16.*2.0+dQ1.*dQ6.*m6.*t2.*t3.*t10.*t20.*2.0-dQ1.*dQ3.*m5.*t7.*t8.*t9.*t16.*2.0+dQ1.*dQ4.*m5.*t2.*t4.*t8.*t25.*2.0+dQ1.*dQ4.*m5.*t3.*t4.*t7.*t25.*2.0+dQ1.*dQ4.*m6.*t2.*t4.*t8.*t26.*2.0+dQ1.*dQ4.*m6.*t3.*t4.*t7.*t26.*2.0-dQ2.*dQ6.*m6.*t4.*t6.*t11.*t17.*2.0-dQ1.*dQ2.*m6.*t7.*t8.*t9.*t20.*2.0;
et491 = dQ3.*dQ6.*m6.*t4.*t6.*t11.*t17.*-2.0-dQ1.*dQ3.*m6.*t7.*t8.*t9.*t20.*2.0+dQ2.*dQ6.*m6.*t4.*t6.*t11.*t20.*2.0+dQ3.*dQ6.*m6.*t4.*t6.*t11.*t20.*2.0-dQ1.*dQ6.*m6.*t7.*t8.*t10.*t20.*2.0+dQ2.*dQ3.*m5.*t5.*t10.*t16.*t34.*2.0-dQ2.*dQ3.*m6.*t5.*t10.*t17.*t36.*2.0+dQ2.*dQ3.*m6.*t5.*t10.*t20.*t34.*2.0-dQ2.*dQ6.*m6.*t5.*t9.*t17.*t36.*2.0+dQ2.*dQ3.*m6.*t5.*t10.*t20.*t36.*2.0-dQ2.*dQ3.*m6.*t5.*t10.*t22.*t34.*2.0-dQ3.*dQ6.*m6.*t5.*t9.*t17.*t36.*2.0-dQ2.*dQ3.*m5.*t5.*t10.*t25.*t34.*2.0+dQ2.*dQ6.*m6.*t5.*t9.*t20.*t36.*2.0+dQ3.*dQ6.*m6.*t5.*t9.*t20.*t36.*2.0-dQ2.*dQ3.*m6.*t5.*t10.*t26.*t34.*2.0-dQ2.*dQ4.*m6.*t9.*t17.*t35.*t36.*2.0-dQ3.*dQ4.*m6.*t9.*t17.*t35.*t36.*2.0+dQ2.*dQ4.*m6.*t9.*t20.*t35.*t36.*2.0+dQ3.*dQ4.*m6.*t9.*t20.*t35.*t36.*2.0;
et492 = Lx3.*Lxcm6.*dQ2.*dQ3.*m6.*t4.*t6.*t10.*2.0+Lx2.*Lxcm5.*dQ1.*dQ2.*m5.*t7.*t9.*t10.*2.0-Lx3.*Lycm6.*dQ2.*dQ3.*m6.*t4.*t10.*t11.*2.0-Lxcm5.*Lycm5.*dQ1.*dQ2.*m5.*t2.*t8.*t10.*2.0-Lxcm5.*Lycm5.*dQ1.*dQ2.*m5.*t3.*t7.*t10.*2.0-Lxcm5.*Lycm5.*dQ1.*dQ3.*m5.*t2.*t8.*t10.*2.0-Lxcm5.*Lycm5.*dQ1.*dQ3.*m5.*t3.*t7.*t10.*2.0+Lxcm6.*Lycm6.*dQ1.*dQ2.*m6.*t2.*t8.*t10.*2.0+Lxcm6.*Lycm6.*dQ1.*dQ2.*m6.*t3.*t7.*t10.*2.0+Lxcm6.*Lycm6.*dQ1.*dQ3.*m6.*t2.*t8.*t10.*2.0+Lxcm6.*Lycm6.*dQ1.*dQ3.*m6.*t3.*t7.*t10.*2.0-Lxcm5.*Lycm5.*dQ2.*dQ3.*m5.*t4.*t9.*t10.*2.0+Lxcm6.*Lycm6.*dQ1.*dQ6.*m6.*t2.*t8.*t9.*2.0+Lxcm6.*Lycm6.*dQ1.*dQ6.*m6.*t3.*t7.*t9.*2.0+Lxcm6.*Lycm6.*dQ2.*dQ3.*m6.*t4.*t9.*t10.*2.0-Lxcm6.*Lycm6.*dQ4.*dQ6.*m6.*t6.*t10.*t11.*4.0-Lxcm6.*Lycm6.*dQ2.*dQ4.*m6.*t4.*t5.*t36.*4.0-Lxcm6.*Lycm6.*dQ3.*dQ4.*m6.*t4.*t5.*t36.*4.0-Lx2.*Lz5.*dQ1.*dQ2.*m6.*t5.*t7.*t9.*2.0;
et493 = Lxcm6.*Lz5.*dQ1.*dQ4.*m6.*t2.*t3.*t6.*2.0-Lx2.*Lzcm5.*dQ1.*dQ2.*m5.*t5.*t7.*t9.*2.0-Lx2.*Lzcm6.*dQ1.*dQ2.*m6.*t5.*t7.*t9.*2.0-Lxcm6.*Lz5.*dQ1.*dQ4.*m6.*t6.*t7.*t8.*2.0-Lxcm6.*Lz5.*dQ2.*dQ4.*m6.*t4.*t10.*t11.*2.0-Lxcm6.*Lz5.*dQ3.*dQ4.*m6.*t4.*t10.*t11.*2.0-Lxcm6.*Lz5.*dQ2.*dQ6.*m6.*t6.*t9.*t10.*2.0-Lxcm6.*Lz5.*dQ3.*dQ6.*m6.*t6.*t9.*t10.*2.0-Lxcm6.*Lz5.*dQ2.*dQ3.*m6.*t6.*t34.*t35.*4.0+Lxcm6.*Lzcm6.*dQ1.*dQ4.*m6.*t2.*t3.*t6.*2.0-Lxcm6.*Lzcm6.*dQ1.*dQ4.*m6.*t6.*t7.*t8.*2.0-Lxcm5.*Lzcm5.*dQ2.*dQ4.*m5.*t5.*t9.*t10.*4.0-Lxcm5.*Lzcm5.*dQ3.*dQ4.*m5.*t5.*t9.*t10.*4.0-Lxcm6.*Lzcm6.*dQ2.*dQ4.*m6.*t4.*t10.*t11.*2.0-Lxcm6.*Lzcm6.*dQ3.*dQ4.*m6.*t4.*t10.*t11.*2.0-Lxcm6.*Lzcm6.*dQ2.*dQ6.*m6.*t6.*t9.*t10.*2.0-Lxcm6.*Lzcm6.*dQ3.*dQ6.*m6.*t6.*t9.*t10.*2.0-Lxcm5.*Lzcm5.*dQ1.*dQ4.*m5.*t2.*t3.*t35.*4.0;
et494 = Lxcm5.*Lzcm5.*dQ1.*dQ4.*m5.*t7.*t8.*t35.*4.0-Lxcm6.*Lzcm6.*dQ2.*dQ3.*m6.*t6.*t34.*t35.*4.0-Lycm6.*Lz5.*dQ1.*dQ4.*m6.*t2.*t3.*t11.*2.0-Lycm6.*Lz5.*dQ2.*dQ4.*m6.*t4.*t6.*t10.*2.0-Lycm6.*Lz5.*dQ3.*dQ4.*m6.*t4.*t6.*t10.*2.0+Lycm6.*Lz5.*dQ1.*dQ4.*m6.*t7.*t8.*t11.*2.0+Lycm6.*Lz5.*dQ2.*dQ6.*m6.*t9.*t10.*t11.*2.0+Lycm6.*Lz5.*dQ3.*dQ6.*m6.*t9.*t10.*t11.*2.0+Lycm6.*Lz5.*dQ2.*dQ3.*m6.*t11.*t34.*t35.*4.0+Lycm5.*Lzcm5.*dQ1.*dQ2.*m5.*t2.*t5.*t8.*2.0+Lycm5.*Lzcm5.*dQ1.*dQ2.*m5.*t3.*t5.*t7.*2.0+Lycm5.*Lzcm5.*dQ1.*dQ3.*m5.*t2.*t5.*t8.*2.0+Lycm5.*Lzcm5.*dQ1.*dQ3.*m5.*t3.*t5.*t7.*2.0+Lycm5.*Lzcm5.*dQ2.*dQ3.*m5.*t4.*t5.*t9.*2.0-Lycm6.*Lzcm6.*dQ1.*dQ4.*m6.*t2.*t3.*t11.*2.0-Lycm6.*Lzcm6.*dQ2.*dQ4.*m6.*t4.*t6.*t10.*2.0-Lycm6.*Lzcm6.*dQ3.*dQ4.*m6.*t4.*t6.*t10.*2.0+Lycm6.*Lzcm6.*dQ1.*dQ4.*m6.*t7.*t8.*t11.*2.0+Lycm6.*Lzcm6.*dQ2.*dQ6.*m6.*t9.*t10.*t11.*2.0;
et495 = Lycm6.*Lzcm6.*dQ3.*dQ6.*m6.*t9.*t10.*t11.*2.0+Lycm6.*Lzcm6.*dQ2.*dQ3.*m6.*t11.*t34.*t35.*4.0+Lz5.*Lzcm6.*dQ1.*dQ4.*m6.*t2.*t4.*t8.*4.0+Lz5.*Lzcm6.*dQ1.*dQ4.*m6.*t3.*t4.*t7.*4.0-Lz5.*Lzcm6.*dQ2.*dQ3.*m6.*t5.*t10.*t34.*4.0+Ixx6.*dQ1.*dQ2.*t2.*t6.*t8.*t10.*t11.*2.0+Ixx6.*dQ1.*dQ2.*t3.*t6.*t7.*t10.*t11.*2.0+Ixx6.*dQ1.*dQ3.*t2.*t6.*t8.*t10.*t11.*2.0+Ixx6.*dQ1.*dQ3.*t3.*t6.*t7.*t10.*t11.*2.0+Ixx6.*dQ1.*dQ6.*t2.*t6.*t8.*t9.*t11.*2.0+Ixx6.*dQ1.*dQ6.*t3.*t6.*t7.*t9.*t11.*2.0+Ixx6.*dQ2.*dQ3.*t4.*t6.*t9.*t10.*t11.*2.0-Ixx6.*dQ1.*dQ4.*t2.*t3.*t5.*t10.*t36.*2.0+Ixx6.*dQ1.*dQ4.*t5.*t7.*t8.*t10.*t36.*2.0+Ixx6.*dQ1.*dQ2.*t2.*t3.*t9.*t35.*t36.*2.0+Ixx6.*dQ1.*dQ3.*t2.*t3.*t9.*t35.*t36.*2.0-Ixx6.*dQ1.*dQ2.*t7.*t8.*t9.*t35.*t36.*2.0-Ixx6.*dQ1.*dQ3.*t7.*t8.*t9.*t35.*t36.*2.0-Ixy6.*dQ1.*dQ2.*t2.*t3.*t6.*t9.*t11.*2.0;
et496 = Ixy6.*dQ1.*dQ3.*t2.*t3.*t6.*t9.*t11.*-2.0-Ixy6.*dQ1.*dQ6.*t2.*t3.*t6.*t10.*t11.*2.0+Ixy6.*dQ1.*dQ2.*t6.*t7.*t8.*t9.*t11.*2.0+Ixy6.*dQ1.*dQ3.*t6.*t7.*t8.*t9.*t11.*2.0+Ixy6.*dQ1.*dQ6.*t6.*t7.*t8.*t10.*t11.*2.0-Ixy6.*dQ1.*dQ4.*t2.*t5.*t8.*t9.*t36.*2.0-Ixy6.*dQ1.*dQ4.*t3.*t5.*t7.*t9.*t36.*2.0-Ixy6.*dQ2.*dQ3.*t5.*t6.*t10.*t11.*t34.*2.0+Ixy6.*dQ1.*dQ2.*t2.*t8.*t10.*t34.*t36.*2.0+Ixy6.*dQ1.*dQ2.*t3.*t7.*t10.*t34.*t36.*2.0+Ixy6.*dQ1.*dQ3.*t2.*t8.*t10.*t34.*t36.*2.0+Ixy6.*dQ1.*dQ3.*t3.*t7.*t10.*t34.*t36.*2.0-Ixz5.*dQ1.*dQ2.*t2.*t3.*t5.*t9.*t10.*2.0-Ixz5.*dQ1.*dQ3.*t2.*t3.*t5.*t9.*t10.*2.0+Ixz6.*dQ1.*dQ2.*t2.*t4.*t6.*t8.*t9+Ixz6.*dQ1.*dQ2.*t3.*t4.*t6.*t7.*t9+Ixz5.*dQ1.*dQ4.*t2.*t4.*t5.*t8.*t10.*2.0+Ixz5.*dQ1.*dQ4.*t3.*t4.*t5.*t7.*t10.*2.0+Ixz6.*dQ1.*dQ3.*t2.*t4.*t6.*t8.*t9;
et497 = Ixz6.*dQ1.*dQ3.*t3.*t4.*t6.*t7.*t9+Ixz6.*dQ1.*dQ6.*t2.*t4.*t6.*t8.*t10+Ixz6.*dQ1.*dQ6.*t3.*t4.*t6.*t7.*t10+Ixz5.*dQ1.*dQ2.*t5.*t7.*t8.*t9.*t10.*2.0+Ixz5.*dQ1.*dQ3.*t5.*t7.*t8.*t9.*t10.*2.0-Ixz6.*dQ1.*dQ4.*t2.*t8.*t9.*t10.*t11-Ixz6.*dQ1.*dQ4.*t3.*t7.*t9.*t10.*t11-Ixz5.*dQ1.*dQ2.*t2.*t4.*t8.*t9.*t35.*2.0-Ixz5.*dQ1.*dQ2.*t3.*t4.*t7.*t9.*t35.*2.0-Ixz5.*dQ1.*dQ3.*t2.*t4.*t8.*t9.*t35.*2.0-Ixz5.*dQ1.*dQ3.*t3.*t4.*t7.*t9.*t35.*2.0-Ixz6.*dQ1.*dQ2.*t2.*t5.*t8.*t11.*t34-Ixz6.*dQ1.*dQ2.*t3.*t5.*t7.*t11.*t34-Ixz6.*dQ1.*dQ3.*t2.*t5.*t8.*t11.*t34-Ixz6.*dQ1.*dQ3.*t3.*t5.*t7.*t11.*t34-Iyx6.*dQ1.*dQ2.*t2.*t3.*t6.*t9.*t11.*2.0-Iyx6.*dQ1.*dQ3.*t2.*t3.*t6.*t9.*t11.*2.0-Iyx6.*dQ1.*dQ6.*t2.*t3.*t6.*t10.*t11.*2.0+Iyx6.*dQ1.*dQ2.*t6.*t7.*t8.*t9.*t11.*2.0;
et498 = Iyx6.*dQ1.*dQ3.*t6.*t7.*t8.*t9.*t11.*2.0+Iyx6.*dQ1.*dQ6.*t6.*t7.*t8.*t10.*t11.*2.0-Iyx6.*dQ1.*dQ4.*t2.*t5.*t8.*t9.*t36.*2.0-Iyx6.*dQ1.*dQ4.*t3.*t5.*t7.*t9.*t36.*2.0-Iyx6.*dQ2.*dQ3.*t5.*t6.*t10.*t11.*t34.*2.0+Iyx6.*dQ1.*dQ2.*t2.*t8.*t10.*t34.*t36.*2.0+Iyx6.*dQ1.*dQ2.*t3.*t7.*t10.*t34.*t36.*2.0+Iyx6.*dQ1.*dQ3.*t2.*t8.*t10.*t34.*t36.*2.0+Iyx6.*dQ1.*dQ3.*t3.*t7.*t10.*t34.*t36.*2.0-Iyy6.*dQ1.*dQ2.*t2.*t6.*t8.*t10.*t11.*2.0-Iyy6.*dQ1.*dQ2.*t3.*t6.*t7.*t10.*t11.*2.0-Iyy6.*dQ1.*dQ3.*t2.*t6.*t8.*t10.*t11.*2.0-Iyy6.*dQ1.*dQ3.*t3.*t6.*t7.*t10.*t11.*2.0-Iyy6.*dQ1.*dQ6.*t2.*t6.*t8.*t9.*t11.*2.0-Iyy6.*dQ1.*dQ6.*t3.*t6.*t7.*t9.*t11.*2.0-Iyy6.*dQ2.*dQ3.*t4.*t6.*t9.*t10.*t11.*2.0+Iyy6.*dQ1.*dQ4.*t2.*t3.*t5.*t10.*t36.*2.0-Iyy6.*dQ1.*dQ4.*t5.*t7.*t8.*t10.*t36.*2.0;
et499 = Iyy6.*dQ1.*dQ2.*t2.*t3.*t9.*t35.*t36.*-2.0-Iyy6.*dQ1.*dQ3.*t2.*t3.*t9.*t35.*t36.*2.0+Iyy6.*dQ1.*dQ2.*t7.*t8.*t9.*t35.*t36.*2.0+Iyy6.*dQ1.*dQ3.*t7.*t8.*t9.*t35.*t36.*2.0-Iyz6.*dQ1.*dQ2.*t2.*t4.*t8.*t9.*t11-Iyz6.*dQ1.*dQ2.*t3.*t4.*t7.*t9.*t11-Iyz6.*dQ1.*dQ3.*t2.*t4.*t8.*t9.*t11-Iyz6.*dQ1.*dQ3.*t3.*t4.*t7.*t9.*t11-Iyz6.*dQ1.*dQ4.*t2.*t6.*t8.*t9.*t10-Iyz6.*dQ1.*dQ4.*t3.*t6.*t7.*t9.*t10-Iyz6.*dQ1.*dQ6.*t2.*t4.*t8.*t10.*t11-Iyz6.*dQ1.*dQ6.*t3.*t4.*t7.*t10.*t11-Iyz6.*dQ1.*dQ2.*t2.*t5.*t6.*t8.*t34-Iyz6.*dQ1.*dQ2.*t3.*t5.*t6.*t7.*t34-Iyz6.*dQ1.*dQ3.*t2.*t5.*t6.*t8.*t34-Iyz6.*dQ1.*dQ3.*t3.*t5.*t6.*t7.*t34-Izx5.*dQ1.*dQ2.*t2.*t3.*t5.*t9.*t10.*2.0-Izx5.*dQ1.*dQ3.*t2.*t3.*t5.*t9.*t10.*2.0;
et500 = Izx6.*dQ1.*dQ2.*t2.*t4.*t6.*t8.*t9+Izx6.*dQ1.*dQ2.*t3.*t4.*t6.*t7.*t9+Izx5.*dQ1.*dQ4.*t2.*t4.*t5.*t8.*t10.*2.0+Izx5.*dQ1.*dQ4.*t3.*t4.*t5.*t7.*t10.*2.0+Izx6.*dQ1.*dQ3.*t2.*t4.*t6.*t8.*t9+Izx6.*dQ1.*dQ3.*t3.*t4.*t6.*t7.*t9+Izx6.*dQ1.*dQ6.*t2.*t4.*t6.*t8.*t10+Izx6.*dQ1.*dQ6.*t3.*t4.*t6.*t7.*t10+Izx5.*dQ1.*dQ2.*t5.*t7.*t8.*t9.*t10.*2.0+Izx5.*dQ1.*dQ3.*t5.*t7.*t8.*t9.*t10.*2.0-Izx6.*dQ1.*dQ4.*t2.*t8.*t9.*t10.*t11-Izx6.*dQ1.*dQ4.*t3.*t7.*t9.*t10.*t11-Izx5.*dQ1.*dQ2.*t2.*t4.*t8.*t9.*t35.*2.0-Izx5.*dQ1.*dQ2.*t3.*t4.*t7.*t9.*t35.*2.0-Izx5.*dQ1.*dQ3.*t2.*t4.*t8.*t9.*t35.*2.0-Izx5.*dQ1.*dQ3.*t3.*t4.*t7.*t9.*t35.*2.0-Izx6.*dQ1.*dQ2.*t2.*t5.*t8.*t11.*t34-Izx6.*dQ1.*dQ2.*t3.*t5.*t7.*t11.*t34-Izx6.*dQ1.*dQ3.*t2.*t5.*t8.*t11.*t34;
et501 = -Izx6.*dQ1.*dQ3.*t3.*t5.*t7.*t11.*t34-Izy6.*dQ1.*dQ2.*t2.*t4.*t8.*t9.*t11-Izy6.*dQ1.*dQ2.*t3.*t4.*t7.*t9.*t11-Izy6.*dQ1.*dQ3.*t2.*t4.*t8.*t9.*t11-Izy6.*dQ1.*dQ3.*t3.*t4.*t7.*t9.*t11-Izy6.*dQ1.*dQ4.*t2.*t6.*t8.*t9.*t10-Izy6.*dQ1.*dQ4.*t3.*t6.*t7.*t9.*t10-Izy6.*dQ1.*dQ6.*t2.*t4.*t8.*t10.*t11-Izy6.*dQ1.*dQ6.*t3.*t4.*t7.*t10.*t11-Izy6.*dQ1.*dQ2.*t2.*t5.*t6.*t8.*t34-Izy6.*dQ1.*dQ2.*t3.*t5.*t6.*t7.*t34-Izy6.*dQ1.*dQ3.*t2.*t5.*t6.*t8.*t34-Izy6.*dQ1.*dQ3.*t3.*t5.*t6.*t7.*t34+dQ1.*dQ4.*m5.*t2.*t3.*t5.*t10.*t16.*2.0+dQ1.*dQ4.*m6.*t2.*t3.*t5.*t10.*t20.*2.0+dQ1.*dQ6.*m6.*t2.*t4.*t5.*t8.*t20.*2.0+dQ1.*dQ6.*m6.*t3.*t4.*t5.*t7.*t20.*2.0-dQ1.*dQ4.*m6.*t2.*t3.*t5.*t10.*t22.*2.0;
et502 = dQ1.*dQ4.*m5.*t2.*t3.*t5.*t10.*t25.*-2.0-dQ2.*dQ4.*m6.*t4.*t5.*t6.*t11.*t17.*2.0-dQ1.*dQ4.*m5.*t5.*t7.*t8.*t10.*t16.*2.0-dQ3.*dQ4.*m6.*t4.*t5.*t6.*t11.*t17.*2.0-dQ1.*dQ4.*m6.*t2.*t3.*t5.*t10.*t26.*2.0-dQ1.*dQ4.*m6.*t5.*t7.*t8.*t10.*t20.*2.0+dQ1.*dQ4.*m6.*t5.*t7.*t8.*t10.*t22.*2.0+dQ1.*dQ4.*m5.*t5.*t7.*t8.*t10.*t25.*2.0+dQ1.*dQ4.*m6.*t5.*t7.*t8.*t10.*t26.*2.0-dQ1.*dQ2.*m5.*t2.*t3.*t9.*t16.*t35.*2.0-dQ1.*dQ3.*m5.*t2.*t3.*t9.*t16.*t35.*2.0+dQ1.*dQ4.*m5.*t2.*t4.*t8.*t16.*t35.*2.0+dQ1.*dQ4.*m5.*t3.*t4.*t7.*t16.*t35.*2.0+dQ1.*dQ2.*m6.*t2.*t3.*t9.*t17.*t36.*2.0+dQ1.*dQ3.*m6.*t2.*t3.*t9.*t17.*t36.*2.0-dQ1.*dQ2.*m6.*t2.*t3.*t9.*t20.*t35.*2.0-dQ1.*dQ2.*m6.*t2.*t3.*t9.*t20.*t36.*2.0-dQ1.*dQ3.*m6.*t2.*t3.*t9.*t20.*t35.*2.0;
et503 = dQ1.*dQ2.*m6.*t2.*t3.*t9.*t22.*t35.*2.0-dQ1.*dQ3.*m6.*t2.*t3.*t9.*t20.*t36.*2.0+dQ1.*dQ4.*m6.*t2.*t4.*t8.*t20.*t35.*2.0+dQ1.*dQ4.*m6.*t3.*t4.*t7.*t20.*t35.*2.0+dQ1.*dQ3.*m6.*t2.*t3.*t9.*t22.*t35.*2.0+dQ1.*dQ6.*m6.*t2.*t3.*t10.*t17.*t36.*2.0+dQ1.*dQ2.*m5.*t2.*t3.*t9.*t25.*t35.*2.0-dQ1.*dQ4.*m6.*t2.*t4.*t8.*t22.*t35.*2.0-dQ1.*dQ4.*m6.*t3.*t4.*t7.*t22.*t35.*2.0+dQ1.*dQ2.*m5.*t7.*t8.*t9.*t16.*t35.*2.0+dQ1.*dQ3.*m5.*t2.*t3.*t9.*t25.*t35.*2.0+dQ1.*dQ2.*m6.*t2.*t3.*t9.*t26.*t35.*2.0+dQ1.*dQ3.*m5.*t7.*t8.*t9.*t16.*t35.*2.0-dQ1.*dQ4.*m5.*t2.*t4.*t8.*t25.*t35.*2.0-dQ1.*dQ4.*m5.*t3.*t4.*t7.*t25.*t35.*2.0-dQ1.*dQ6.*m6.*t2.*t3.*t10.*t20.*t36.*2.0+dQ1.*dQ3.*m6.*t2.*t3.*t9.*t26.*t35.*2.0-dQ1.*dQ2.*m6.*t7.*t8.*t9.*t17.*t36.*2.0-dQ1.*dQ4.*m6.*t2.*t4.*t8.*t26.*t35.*2.0;
et504 = dQ1.*dQ4.*m6.*t3.*t4.*t7.*t26.*t35.*-2.0-dQ1.*dQ3.*m6.*t7.*t8.*t9.*t17.*t36.*2.0+dQ1.*dQ2.*m6.*t7.*t8.*t9.*t20.*t35.*2.0+dQ1.*dQ2.*m6.*t7.*t8.*t9.*t20.*t36.*2.0+dQ1.*dQ3.*m6.*t7.*t8.*t9.*t20.*t35.*2.0-dQ1.*dQ2.*m6.*t7.*t8.*t9.*t22.*t35.*2.0+dQ1.*dQ3.*m6.*t7.*t8.*t9.*t20.*t36.*2.0-dQ1.*dQ3.*m6.*t7.*t8.*t9.*t22.*t35.*2.0-dQ1.*dQ6.*m6.*t7.*t8.*t10.*t17.*t36.*2.0-dQ1.*dQ2.*m5.*t7.*t8.*t9.*t25.*t35.*2.0-dQ1.*dQ3.*m5.*t7.*t8.*t9.*t25.*t35.*2.0-dQ1.*dQ2.*m6.*t7.*t8.*t9.*t26.*t35.*2.0+dQ1.*dQ6.*m6.*t7.*t8.*t10.*t20.*t36.*2.0-dQ1.*dQ3.*m6.*t7.*t8.*t9.*t26.*t35.*2.0+dQ2.*dQ3.*m6.*t5.*t10.*t17.*t34.*t36.*2.0-dQ2.*dQ3.*m6.*t5.*t10.*t20.*t34.*t36.*2.0-Ixx5.*dQ1.*dQ2.*t2.*t4.*t5.*t8.*t9.*t10.*2.0-Ixx5.*dQ1.*dQ2.*t3.*t4.*t5.*t7.*t9.*t10.*2.0;
et505 = Ixx5.*dQ1.*dQ3.*t2.*t4.*t5.*t8.*t9.*t10.*-2.0-Ixx5.*dQ1.*dQ3.*t3.*t4.*t5.*t7.*t9.*t10.*2.0-Ixx6.*dQ1.*dQ2.*t2.*t6.*t8.*t10.*t11.*t34.*2.0-Ixx6.*dQ1.*dQ2.*t3.*t6.*t7.*t10.*t11.*t34.*2.0-Ixx6.*dQ1.*dQ3.*t2.*t6.*t8.*t10.*t11.*t34.*2.0-Ixx6.*dQ1.*dQ3.*t3.*t6.*t7.*t10.*t11.*t34.*2.0-Ixy6.*dQ1.*dQ4.*t2.*t3.*t5.*t6.*t10.*t11.*2.0-Ixy6.*dQ1.*dQ6.*t2.*t4.*t5.*t6.*t8.*t11.*2.0-Ixy6.*dQ1.*dQ6.*t3.*t4.*t5.*t6.*t7.*t11.*2.0+Ixy6.*dQ1.*dQ4.*t5.*t6.*t7.*t8.*t10.*t11.*2.0+Ixy6.*dQ1.*dQ2.*t2.*t3.*t6.*t9.*t11.*t35.*2.0+Ixy6.*dQ1.*dQ3.*t2.*t3.*t6.*t9.*t11.*t35.*2.0-Ixy6.*dQ1.*dQ4.*t2.*t4.*t6.*t8.*t11.*t35.*2.0-Ixy6.*dQ1.*dQ4.*t3.*t4.*t6.*t7.*t11.*t35.*2.0-Ixy6.*dQ1.*dQ2.*t6.*t7.*t8.*t9.*t11.*t35.*2.0-Ixy6.*dQ1.*dQ3.*t6.*t7.*t8.*t9.*t11.*t35.*2.0;
et506 = Ixz6.*dQ1.*dQ2.*t2.*t3.*t5.*t6.*t9.*t10.*-2.0-Ixz6.*dQ1.*dQ3.*t2.*t3.*t5.*t6.*t9.*t10.*2.0+Ixz6.*dQ1.*dQ4.*t2.*t4.*t5.*t6.*t8.*t10.*2.0+Ixz6.*dQ1.*dQ4.*t3.*t4.*t5.*t6.*t7.*t10.*2.0+Ixz6.*dQ1.*dQ2.*t5.*t6.*t7.*t8.*t9.*t10.*2.0+Ixz6.*dQ1.*dQ3.*t5.*t6.*t7.*t8.*t9.*t10.*2.0-Ixz6.*dQ1.*dQ2.*t2.*t4.*t6.*t8.*t9.*t35.*2.0-Ixz6.*dQ1.*dQ2.*t3.*t4.*t6.*t7.*t9.*t35.*2.0-Ixz6.*dQ1.*dQ3.*t2.*t4.*t6.*t8.*t9.*t35.*2.0-Ixz6.*dQ1.*dQ3.*t3.*t4.*t6.*t7.*t9.*t35.*2.0-Iyx6.*dQ1.*dQ4.*t2.*t3.*t5.*t6.*t10.*t11.*2.0-Iyx6.*dQ1.*dQ6.*t2.*t4.*t5.*t6.*t8.*t11.*2.0-Iyx6.*dQ1.*dQ6.*t3.*t4.*t5.*t6.*t7.*t11.*2.0+Iyx6.*dQ1.*dQ4.*t5.*t6.*t7.*t8.*t10.*t11.*2.0+Iyx6.*dQ1.*dQ2.*t2.*t3.*t6.*t9.*t11.*t35.*2.0+Iyx6.*dQ1.*dQ3.*t2.*t3.*t6.*t9.*t11.*t35.*2.0-Iyx6.*dQ1.*dQ4.*t2.*t4.*t6.*t8.*t11.*t35.*2.0;
et507 = Iyx6.*dQ1.*dQ4.*t3.*t4.*t6.*t7.*t11.*t35.*-2.0-Iyx6.*dQ1.*dQ2.*t6.*t7.*t8.*t9.*t11.*t35.*2.0-Iyx6.*dQ1.*dQ3.*t6.*t7.*t8.*t9.*t11.*t35.*2.0-Iyy6.*dQ1.*dQ2.*t2.*t4.*t5.*t8.*t9.*t10.*2.0-Iyy6.*dQ1.*dQ2.*t3.*t4.*t5.*t7.*t9.*t10.*2.0-Iyy6.*dQ1.*dQ3.*t2.*t4.*t5.*t8.*t9.*t10.*2.0-Iyy6.*dQ1.*dQ3.*t3.*t4.*t5.*t7.*t9.*t10.*2.0+Iyy6.*dQ1.*dQ2.*t2.*t6.*t8.*t10.*t11.*t34.*2.0+Iyy6.*dQ1.*dQ2.*t3.*t6.*t7.*t10.*t11.*t34.*2.0+Iyy6.*dQ1.*dQ3.*t2.*t6.*t8.*t10.*t11.*t34.*2.0+Iyy6.*dQ1.*dQ3.*t3.*t6.*t7.*t10.*t11.*t34.*2.0+Iyz6.*dQ1.*dQ2.*t2.*t3.*t5.*t9.*t10.*t11.*2.0+Iyz6.*dQ1.*dQ3.*t2.*t3.*t5.*t9.*t10.*t11.*2.0-Iyz6.*dQ1.*dQ4.*t2.*t4.*t5.*t8.*t10.*t11.*2.0-Iyz6.*dQ1.*dQ4.*t3.*t4.*t5.*t7.*t10.*t11.*2.0-Iyz6.*dQ1.*dQ2.*t5.*t7.*t8.*t9.*t10.*t11.*2.0-Iyz6.*dQ1.*dQ3.*t5.*t7.*t8.*t9.*t10.*t11.*2.0;
et508 = Iyz6.*dQ1.*dQ2.*t2.*t4.*t8.*t9.*t11.*t35.*2.0+Iyz6.*dQ1.*dQ2.*t3.*t4.*t7.*t9.*t11.*t35.*2.0+Iyz6.*dQ1.*dQ3.*t2.*t4.*t8.*t9.*t11.*t35.*2.0+Iyz6.*dQ1.*dQ3.*t3.*t4.*t7.*t9.*t11.*t35.*2.0-Izx6.*dQ1.*dQ2.*t2.*t3.*t5.*t6.*t9.*t10.*2.0-Izx6.*dQ1.*dQ3.*t2.*t3.*t5.*t6.*t9.*t10.*2.0+Izx6.*dQ1.*dQ4.*t2.*t4.*t5.*t6.*t8.*t10.*2.0+Izx6.*dQ1.*dQ4.*t3.*t4.*t5.*t6.*t7.*t10.*2.0+Izx6.*dQ1.*dQ2.*t5.*t6.*t7.*t8.*t9.*t10.*2.0+Izx6.*dQ1.*dQ3.*t5.*t6.*t7.*t8.*t9.*t10.*2.0-Izx6.*dQ1.*dQ2.*t2.*t4.*t6.*t8.*t9.*t35.*2.0-Izx6.*dQ1.*dQ2.*t3.*t4.*t6.*t7.*t9.*t35.*2.0-Izx6.*dQ1.*dQ3.*t2.*t4.*t6.*t8.*t9.*t35.*2.0-Izx6.*dQ1.*dQ3.*t3.*t4.*t6.*t7.*t9.*t35.*2.0+Izy6.*dQ1.*dQ2.*t2.*t3.*t5.*t9.*t10.*t11.*2.0+Izy6.*dQ1.*dQ3.*t2.*t3.*t5.*t9.*t10.*t11.*2.0-Izy6.*dQ1.*dQ4.*t2.*t4.*t5.*t8.*t10.*t11.*2.0;
et509 = Izy6.*dQ1.*dQ4.*t3.*t4.*t5.*t7.*t10.*t11.*-2.0-Izy6.*dQ1.*dQ2.*t5.*t7.*t8.*t9.*t10.*t11.*2.0-Izy6.*dQ1.*dQ3.*t5.*t7.*t8.*t9.*t10.*t11.*2.0+Izy6.*dQ1.*dQ2.*t2.*t4.*t8.*t9.*t11.*t35.*2.0+Izy6.*dQ1.*dQ2.*t3.*t4.*t7.*t9.*t11.*t35.*2.0+Izy6.*dQ1.*dQ3.*t2.*t4.*t8.*t9.*t11.*t35.*2.0+Izy6.*dQ1.*dQ3.*t3.*t4.*t7.*t9.*t11.*t35.*2.0+Izz5.*dQ1.*dQ2.*t2.*t4.*t5.*t8.*t9.*t10.*2.0+Izz5.*dQ1.*dQ2.*t3.*t4.*t5.*t7.*t9.*t10.*2.0+Izz5.*dQ1.*dQ3.*t2.*t4.*t5.*t8.*t9.*t10.*2.0+Izz5.*dQ1.*dQ3.*t3.*t4.*t5.*t7.*t9.*t10.*2.0+Izz6.*dQ1.*dQ2.*t2.*t4.*t5.*t8.*t9.*t10.*2.0+Izz6.*dQ1.*dQ2.*t3.*t4.*t5.*t7.*t9.*t10.*2.0+Izz6.*dQ1.*dQ3.*t2.*t4.*t5.*t8.*t9.*t10.*2.0+Izz6.*dQ1.*dQ3.*t3.*t4.*t5.*t7.*t9.*t10.*2.0-dQ1.*dQ2.*m6.*t2.*t6.*t8.*t10.*t11.*t17.*2.0-dQ1.*dQ2.*m6.*t3.*t6.*t7.*t10.*t11.*t17.*2.0;
